simulink model "dynamicsSimulation"  (R2023a)
settings: Solver=VariableStepAuto  StartTime=0.0  StopTime=35  RelTol=1e-3
(part 2 of 2)

== matlab function dynamicsSimulation/MATLAB Function ==
  data: q input; qpp output; qp input; T input
function qpp = qpp_rrr(q,qp,T)
q2 = q(2);
q3 = q(3);
qp1 = qp(1);
qp2 = qp(2);
qp3 = qp(3);
t1 = T(1);
t2 = T(2);
t3 = T(3);
Ixx1 = 0.1;
Ixx2 = 0.1;
Ixx3 = 0.1;
Iyy2 = 0.1;
Iyy3 = 0.1;
Izz2 = 0.1;
Izz3 = 0.1;
g = 9.81;
l2 = 0.15;
lcm2 = 0.075;
lcm3 = 0.1;
m2 = 0.5;
m3 = 0.4;
%    This function was generated by the Symbolic Math Toolbox version 9.3.
%    05-Oct-2023 00:48:23

t5 = cos(q2);
t6 = cos(q3);
t7 = sin(q2);
t8 = sin(q3);
t9 = Ixx2.^2;
t10 = Ixx3.^2;
t11 = Iyy3.^2;
t12 = Izz2.^2;
t13 = Izz3.^2;
t14 = l2.^2;
t15 = l2.^3;
t17 = l2.^5;
t18 = lcm2.^2;
t19 = lcm2.^3;
t20 = lcm3.^2;
t22 = lcm3.^3;
t24 = lcm3.^5;
t25 = m2.^2;
t26 = m3.^2;
t27 = m3.^3;
t28 = q2.*2.0;
t29 = q3.*2.0;
t30 = qp1.^2;
t31 = qp2.^2;
t32 = qp3.^2;
t40 = Ixx1.*Iyy2.*Iyy3;
t41 = Ixx1.*Iyy3.*Izz3;
t42 = Iyy2.*Iyy3.*Izz2;
t43 = Iyy3.*Izz2.*Izz3;
t16 = t14.^2;
t21 = t18.^2;
t23 = t20.^2;
t33 = t5.^2;
t34 = t5.^3;
t35 = t6.^2;
t37 = t6.^3;
t39 = t6.^5;
t44 = sin(t28);
t45 = sin(t29);
t46 = t7.^2;
t47 = t7.^3;
t48 = t8.^2;
t49 = t8.^3;
t50 = Ixx1.*Iyy3.*m3.*t14;
t51 = Iyy2.*Iyy3.*m3.*t14;
t52 = Iyy3.*Izz2.*m3.*t14;
t53 = Iyy3.*Izz3.*m3.*t14;
t54 = Ixx1.*Iyy3.*m2.*t18;
t55 = Ixx1.*Iyy2.*m3.*t20;
t56 = Iyy2.*Iyy3.*m2.*t18;
t57 = Ixx1.*Izz3.*m3.*t20;
t58 = Iyy3.*Izz2.*m2.*t18;
t59 = Iyy2.*Izz2.*m3.*t20;
t60 = Iyy3.*Izz3.*m2.*t18;
t61 = Izz2.*Izz3.*m3.*t20;
t78 = Ixx1.*Iyy3.*l2.*lcm3.*m3.*t6.*2.0;
t79 = Iyy3.*Izz2.*l2.*lcm3.*m3.*t6.*2.0;
t80 = Ixx1.*m2.*m3.*t18.*t20;
t81 = Iyy2.*m2.*m3.*t18.*t20;
t82 = Izz2.*m2.*m3.*t18.*t20;
t83 = Izz3.*m2.*m3.*t18.*t20;
t91 = Ixx1.*t14.*t20.*t26;
t92 = Iyy2.*t14.*t20.*t26;
t93 = Izz2.*t14.*t20.*t26;
t94 = Izz3.*t14.*t20.*t26;
t95 = Iyy3.*m2.*m3.*t14.*t18.*2.0;
t131 = Ixx1.*l2.*t6.*t22.*t26.*2.0;
t132 = Iyy3.*lcm3.*t6.*t15.*t26.*2.0;
t133 = Izz2.*l2.*t6.*t22.*t26.*2.0;
t140 = Iyy3.*l2.*lcm3.*m2.*m3.*t6.*t18.*2.0;
t156 = t6.*t15.*t22.*t27.*2.0;
t190 = l2.*m2.*t6.*t18.*t22.*t26.*2.0;
t201 = m2.*t14.*t18.*t20.*t26.*2.0;
t36 = t33.^2;
t38 = t35.^2;
t62 = -t47;
t63 = -t49;
t64 = t46-1.0;
t65 = t48-1.0;
t66 = Iyy3.*t16.*t26;
t67 = Iyy3.*t21.*t25;
t68 = Ixx1.*Ixx3.*Iyy3.*t35;
t69 = Ixx2.*Iyy2.*Iyy3.*t33;
t70 = Ixx3.*Iyy2.*Iyy3.*t33;
t71 = t35.*t41;
t72 = Ixx2.*Iyy3.*Izz3.*t33;
t73 = Ixx3.*Iyy3.*Izz2.*t35;
t74 = Ixx3.*Iyy3.*Izz3.*t33;
t75 = t33.*t42;
t76 = t33.*t43;
t77 = t35.*t43;
t88 = t16.*t20.*t27;
t96 = m3.*t20.*t21.*t25;
t97 = Ixx2.*Iyy3.*m3.*t14.*t33;
t98 = Ixx3.*Iyy3.*m3.*t14.*t33;
t99 = Ixx3.*Iyy3.*m3.*t14.*t35;
t100 = t33.*t51;
t101 = t33.*t52;
t102 = t33.*t53;
t103 = t35.*t53;
t104 = Ixx1.*Ixx3.*m3.*t20.*t35;
t105 = Ixx2.*Iyy3.*m2.*t18.*t33;
t106 = Ixx2.*Iyy2.*m3.*t20.*t33;
t107 = Ixx3.*Iyy3.*m2.*t18.*t33;
t108 = Ixx1.*Iyy3.*m3.*t20.*t35;
t109 = Ixx3.*Iyy2.*m3.*t20.*t33;
t110 = Ixx3.*Iyy3.*m2.*t18.*t35;
t111 = t33.*t56;
t112 = t35.*t57;
t113 = Ixx2.*Izz3.*m3.*t20.*t33;
t114 = Iyy2.*Iyy3.*m3.*t20.*t33;
t115 = Ixx3.*Izz2.*m3.*t20.*t35;
t116 = Ixx3.*Izz3.*m3.*t20.*t33;
t117 = t33.*t58;
t118 = t33.*t59;
t119 = t33.*t60;
t120 = t35.*t60;
t121 = Iyy3.*Izz2.*m3.*t20.*t35;
t122 = Iyy3.*Izz3.*m3.*t20.*t33;
t123 = t33.*t61;
t124 = t35.*t61;
t126 = Ixx1.*t23.*t26.*t35;
t128 = Iyy2.*t23.*t26.*t33;
t129 = Izz2.*t23.*t26.*t35;
t130 = Izz3.*t23.*t26.*t33;
t134 = Ixx2.*Ixx3.*Iyy3.*t33.*t35;
t138 = Iyy2.*Iyy3.*Izz3.*t33.*t35;
t141 = Ixx2.*Iyy3.*l2.*lcm3.*m3.*t6.*t33.*2.0;
t143 = Iyy3.*Izz3.*l2.*lcm3.*m3.*t6.*t33.*2.0;
t157 = Iyy3.*Izz2.*l2.*lcm3.*m3.*t6.*t33.*-2.0;
t158 = Ixx2.*m2.*m3.*t18.*t20.*t33;
t159 = Ixx3.*m2.*m3.*t18.*t20.*t33;
t160 = Ixx3.*m2.*m3.*t18.*t20.*t35;
t161 = t33.*t81;
t162 = Iyy3.*m2.*m3.*t18.*t20.*t33;
t163 = Iyy3.*m2.*m3.*t18.*t20.*t35;
t164 = t33.*t82;
t165 = t33.*t83;
t166 = t35.*t83;
t173 = t14.*t23.*t27.*t35;
t176 = Ixx2.*t14.*t20.*t26.*t33;
t177 = Ixx3.*t14.*t20.*t26.*t33;
t178 = Ixx3.*t14.*t20.*t26.*t35;
t180 = t33.*t92;
t181 = t35.*t92;
t182 = Iyy3.*t14.*t20.*t26.*t35;
t183 = t33.*t93;
t184 = t33.*t94;
t187 = m2.*t18.*t23.*t26.*t33;
t189 = m2.*t18.*t23.*t26.*t35;
t191 = Ixx2.*Ixx3.*m3.*t20.*t33.*t35;
t192 = Ixx2.*Iyy3.*m3.*t20.*t33.*t35;
t197 = Iyy2.*Izz3.*m3.*t20.*t33.*t35;
t200 = t15.*t22.*t27.*t37.*2.0;
t203 = t35.*t94.*2.0;
t204 = Iyy3.*m2.*m3.*t14.*t18.*t33.*-2.0;
t213 = Ixx2.*t23.*t26.*t33.*t35;
t216 = Ixx2.*l2.*t6.*t22.*t26.*t33.*2.0;
t219 = Izz3.*l2.*t6.*t22.*t26.*t33.*2.0;
t224 = Iyy3.*l2.*lcm3.*m2.*m3.*t6.*t18.*t33.*-2.0;
t239 = Iyy3.*lcm3.*t6.*t15.*t26.*t33.*-2.0;
t240 = Izz2.*l2.*t6.*t22.*t26.*t33.*-2.0;
t245 = m2.*t14.*t18.*t20.*t26.*t35;
t248 = t6.*t15.*t22.*t27.*t33.*-2.0;
t250 = t33.*t201;
t260 = m2.*t14.*t18.*t20.*t26.*t33.*-2.0;
t267 = l2.*m2.*t6.*t18.*t22.*t26.*t33.*-2.0;
t84 = -t71;
t85 = -t75;
t86 = -t76;
t87 = -t77;
t89 = t7+t62;
t90 = t8+t63;
t125 = t33.*t66;
t127 = t33.*t67;
t135 = t35.*t70;
t136 = t35.*t72;
t137 = t33.*t73;
t139 = t35.*t76;
t144 = -t100;
t145 = -t101;
t146 = -t102;
t147 = -t103;
t148 = -t111;
t149 = -t112;
t150 = -t117;
t151 = -t118;
t152 = -t119;
t153 = -t120;
t154 = -t123;
t155 = -t124;
t172 = t33.*t88;
t174 = t35.*t88;
t175 = t14.*t23.*t27.*t38;
t179 = Ixx3.*t14.*t20.*t26.*t38;
t185 = t38.*t94;
t188 = t33.*t96;
t193 = t35.*t109;
t194 = t35.*t113;
t195 = t33.*t115;
t196 = t35.*t114;
t198 = t33.*t121;
t199 = t35.*t123;
t205 = -t161;
t206 = -t164;
t207 = -t165;
t208 = -t166;
t209 = t35.*t98.*2.0;
t210 = t35.*t102.*2.0;
t211 = t35.*t107.*2.0;
t212 = t35.*t119.*2.0;
t214 = t35.*t128;
t215 = t33.*t129;
t223 = -t200;
t226 = -t180;
t227 = -t181;
t228 = -t183;
t229 = -t184;
t230 = -t203;
t242 = t33.*t173;
t249 = t33.*t200;
t251 = t38.*t177;
t252 = t35.*t180;
t253 = t33.*t182;
t255 = t35.*t159.*2.0;
t256 = t35.*t162.*2.0;
t257 = t35.*t165.*2.0;
t261 = -t245;
t262 = t35.*t177.*2.0;
t263 = t35.*t184.*3.0;
t266 = t35.*t187.*2.0;
t272 = t33.*t245;
t167 = -t125;
t168 = -t127;
t169 = -t135;
t170 = -t136;
t171 = -t137;
t220 = -t172;
t221 = -t174;
t222 = -t175;
t225 = -t179;
t231 = -t188;
t232 = -t209;
t233 = -t193;
t234 = -t211;
t235 = -t194;
t236 = -t195;
t237 = -t196;
t238 = -t198;
t243 = t35.*t172;
t244 = t33.*t175;
t246 = -t214;
t247 = -t215;
t259 = -t242;
t264 = -t255;
t265 = -t256;
t268 = -t262;
t269 = -t253;
t270 = t38.*t229;
t271 = -t266;
t273 = t40+t41+t42+t43+t50+t51+t52+t53+t54+t55+t56+t57+t58+t59+t60+t61+t66+t67+t68+t69+t70+t72+t73+t74+t78+t79+t80+t81+t82+t83+t84+t85+t86+t87+t88+t91+t92+t93+t94+t95+t96+t97+t98+t99+t104+t105+t106+t107+t108+t109+t110+t113+t114+t115+t116+t121+t122+t126+t128+t129+t130+t131+t132+t133+t134+t138+t139+t140+t141+t143+t144+t145+t146+t147+t148+t149+t150+t151+t152+t153+t154+t155+t156+t157+t158+t159+t160+t162+t163+t167+t168+t169+t170+t171+t173+t176+t177+t178+t182+t185+t187+t189+t190+t191+t192+t197+t199+t201+t204+t205+t206+t207+t208+t210+t212+t213+t216+t219+t220+t221+t222+t223+t224+t225+t226+t227+t228+t229+t230+t231+t232+t233+t234+t235+t236+t237+t238+t239+t240+t243+t244+t246+t247+t248+t249+t251+t252+t257+t259+t260+t261+t263+t264+t265+t267+t268+t269+t270+t271+t272;
t274 = 1.0./t273;
et1 = Iyy2.*Iyy3.*t1+Iyy3.*Izz3.*t1-qp2.*qp3.*t5.*t53-qp2.*qp3.*t5.*t60-qp1.*qp2.*t42.*t44-qp1.*qp2.*t43.*t44-qp2.*qp3.*t5.*t83-qp1.*qp2.*t44.*t51-qp1.*qp2.*t44.*t52-(qp1.*qp2.*t44.*t53)./2.0-qp1.*qp2.*t44.*t56-qp2.*qp3.*t5.*t94-qp1.*qp2.*t44.*t58-qp1.*qp2.*t44.*t59-(qp1.*qp2.*t44.*t60)./2.0-qp1.*qp2.*t44.*t61-qp2.*qp3.*t5.*t99.*2.0-qp1.*qp2.*t44.*t66+qp2.*qp3.*t5.*t103.*2.0-qp1.*qp2.*t44.*t67-qp2.*qp3.*t5.*t110.*2.0-qp1.*qp2.*t44.*t81-qp1.*qp2.*t44.*t82-(qp1.*qp2.*t44.*t83)./2.0+qp2.*qp3.*t5.*t120.*2.0-qp1.*qp2.*t44.*t88-qp1.*qp2.*t44.*t92-qp1.*qp2.*t44.*t93;
et2 = qp1.*qp2.*t44.*t94.*(-1.0./2.0)-qp1.*qp2.*t44.*t96-qp2.*qp3.*t5.*t160.*2.0-qp2.*qp3.*t5.*t163.*2.0+qp2.*qp3.*t5.*t166.*2.0-qp2.*qp3.*t5.*t178.*2.0-qp2.*qp3.*t5.*t189.*2.0+qp2.*qp3.*t5.*t203+t1.*t14.*t20.*t26+t1.*t23.*t26.*t35+Ixx3.*Iyy3.*t1.*t35+Iyy2.*Iyy3.*t3.*t7+Iyy3.*Izz3.*t3.*t7-Iyy3.*Izz3.*t1.*t35+Iyy3.*m3.*t1.*t14+Iyy3.*m2.*t1.*t18+Iyy2.*m3.*t1.*t20+Izz3.*m3.*t1.*t20+Ixx3.*Iyy3.*t3.*t7.*t35-Iyy3.*Izz3.*t3.*t7.*t35+Ixx3.*m3.*t1.*t20.*t35+Iyy3.*m3.*t3.*t7.*t14+Iyy3.*m2.*t3.*t7.*t18+Iyy2.*m3.*t3.*t7.*t20+Iyy3.*m3.*t1.*t20.*t35+Izz3.*m3.*t3.*t7.*t20-Izz3.*m3.*t1.*t20.*t35+Iyy2.*qp2.*qp3.*t5.*t11-Iyy3.*qp2.*qp3.*t5.*t13-(Iyy2.*qp1.*qp2.*t11.*t44)./2.0+(Iyy3.*qp1.*qp2.*t13.*t44)./2.0;
et3 = Izz3.*qp2.*qp3.*t5.*t11-(Izz3.*qp1.*qp2.*t11.*t44)./2.0+m2.*m3.*t1.*t18.*t20+l2.*t1.*t6.*t22.*t26.*2.0-qp1.*qp2.*t5.*t7.*t73.*2.0-qp1.*qp3.*t6.*t8.*t70.*2.0+qp1.*qp2.*t5.*t7.*t77.*2.0-qp1.*qp2.*t5.*t7.*t99.*2.0-qp1.*qp3.*t6.*t8.*t98.*2.0+qp1.*qp2.*t5.*t7.*t103.*2.0+qp1.*qp3.*t6.*t8.*t102.*2.0-qp1.*qp2.*t5.*t7.*t110.*2.0-qp1.*qp3.*t6.*t8.*t107.*2.0-qp1.*qp3.*t6.*t8.*t109.*2.0-qp1.*qp2.*t5.*t7.*t115.*2.0-qp1.*qp3.*t6.*t8.*t114.*2.0+qp1.*qp2.*t5.*t7.*t120.*2.0-qp1.*qp2.*t5.*t7.*t121.*2.0+qp1.*qp3.*t6.*t8.*t119.*2.0+qp1.*qp2.*t5.*t7.*t124.*2.0-qp1.*qp3.*t6.*t8.*t122.*2.0-qp1.*qp2.*t5.*t7.*t129.*2.0-qp1.*qp3.*t6.*t8.*t128.*2.0-qp1.*qp3.*t6.*t8.*t130-qp1.*qp2.*t5.*t7.*t160.*2.0-qp1.*qp3.*t6.*t8.*t159.*2.0;
et4 = qp1.*qp2.*t5.*t7.*t163.*-2.0-qp1.*qp3.*t6.*t8.*t162.*2.0+qp1.*qp2.*t5.*t7.*t166.*2.0+qp1.*qp3.*t6.*t8.*t165.*2.0-qp1.*qp2.*t5.*t7.*t173.*6.0+qp1.*qp2.*t5.*t7.*t174.*2.0+qp1.*qp2.*t5.*t7.*t175.*6.0-qp1.*qp2.*t5.*t7.*t178.*4.0+qp1.*qp2.*t5.*t7.*t179.*6.0-qp1.*qp3.*t6.*t8.*t177.*2.0+qp1.*qp2.*t5.*t7.*t181.*2.0-qp1.*qp2.*t5.*t7.*t182.*4.0-qp1.*qp2.*t5.*t7.*t185.*6.0+qp1.*qp3.*t6.*t8.*t184.*2.0-qp1.*qp2.*t5.*t7.*t189.*2.0-qp1.*qp3.*t6.*t8.*t187.*2.0+t3.*t7.*t14.*t20.*t26+t3.*t7.*t23.*t26.*t35+t6.*t7.*t8.*t30.*t70-t6.*t7.*t8.*t30.*t72+t6.*t7.*t8.*t30.*t76-t6.*t7.*t8.*t30.*t88-t6.*t7.*t8.*t31.*t88-t6.*t7.*t8.*t30.*t92-t6.*t7.*t8.*t31.*t92-t6.*t7.*t8.*t30.*t94;
et5 = -t6.*t7.*t8.*t31.*t94+t6.*t7.*t8.*t30.*t109-t6.*t7.*t8.*t30.*t113+t6.*t7.*t8.*t30.*t114+t6.*t7.*t8.*t30.*t122.*2.0+t6.*t7.*t8.*t30.*t123+t7.*t8.*t30.*t37.*t94+t7.*t8.*t31.*t37.*t94.*3.0+t6.*t7.*t8.*t30.*t128+t6.*t7.*t8.*t30.*t130+t6.*t7.*t8.*t30.*t172+t6.*t7.*t8.*t30.*t180+t6.*t7.*t8.*t30.*t184+t7.*t8.*t30.*t37.*t177.*3.0-t7.*t8.*t30.*t37.*t184.*3.0+m2.*m3.*t3.*t7.*t18.*t20+l2.*qp1.*qp3.*t24.*t27.*t90.*2.0+m3.*qp2.*qp3.*t5.*t11.*t14+m2.*qp2.*qp3.*t5.*t11.*t18-m3.*qp2.*qp3.*t5.*t13.*t20-(m3.*qp1.*qp2.*t11.*t14.*t44)./2.0-(m2.*qp1.*qp2.*t11.*t18.*t44)./2.0+(m3.*qp1.*qp2.*t13.*t20.*t44)./2.0-l2.*t2.*t5.*t8.*t22.*t26+l2.*t3.*t6.*t7.*t22.*t26.*2.0+l2.*t3.*t7.*t22.*t26.*t37+lcm3.*t3.*t6.*t7.*t15.*t26;
et6 = qp1.*qp3.*t8.*t15.*t22.*t27.*2.0+qp1.*qp3.*t14.*t23.*t27.*t45.*2.0+qp1.*qp2.*t5.*t7.*t35.*t94.*6.0+qp1.*qp2.*t5.*t7.*t35.*t201-t2.*t5.*t6.*t8.*t23.*t26+t3.*t7.*t14.*t20.*t26.*t35.*2.0-t7.*t8.*t15.*t22.*t27.*t30-t7.*t8.*t15.*t22.*t27.*t32+Ixx3.*Iyy2.*Iyy3.*qp2.*qp3.*t5+Ixx2.*Iyy2.*Iyy3.*qp1.*qp2.*t44+(Ixx3.*Iyy2.*Iyy3.*qp1.*qp2.*t44)./2.0+Ixx3.*Iyy3.*Izz3.*qp2.*qp3.*t5+Ixx2.*Iyy3.*Izz3.*qp1.*qp2.*t44+(Ixx3.*Iyy3.*Izz3.*qp1.*qp2.*t44)./2.0-Iyy2.*Iyy3.*Izz3.*qp2.*qp3.*t5+(Iyy2.*Iyy3.*Izz3.*qp1.*qp2.*t44)./2.0-Ixx3.*Iyy3.*t2.*t5.*t6.*t8+Iyy3.*Izz3.*t2.*t5.*t6.*t8+Iyy3.*l2.*lcm3.*m3.*t1.*t6.*2.0+Ixx3.*m3.*t3.*t7.*t20.*t35+Iyy3.*m3.*t3.*t7.*t20.*t35-Izz3.*m3.*t3.*t7.*t20.*t35+Ixx3.*qp2.*qp3.*t5.*t11.*t35-Iyy3.*qp2.*qp3.*t5.*t10.*t35;
et7 = Iyy2.*qp2.*qp3.*t5.*t23.*t26.*2.0+Iyy3.*qp2.*qp3.*t5.*t13.*t35-Izz3.*qp2.*qp3.*t5.*t11.*t35+Izz3.*qp2.*qp3.*t5.*t23.*t26.*2.0-Ixx3.*Iyy2.*Iyy3.*qp2.*qp3.*t5.*t35.*2.0+Iyy2.*Iyy3.*Izz3.*qp2.*qp3.*t5.*t35.*2.0+Ixx3.*Iyy3.*m3.*qp2.*qp3.*t5.*t14+Ixx3.*Iyy3.*m2.*qp2.*qp3.*t5.*t18+Ixx3.*Iyy2.*m3.*qp2.*qp3.*t5.*t20+Ixx2.*Iyy3.*m3.*qp1.*qp2.*t14.*t44+(Ixx3.*Iyy3.*m3.*qp1.*qp2.*t14.*t44)./2.0+Ixx2.*Iyy3.*m2.*qp1.*qp2.*t18.*t44+(Ixx3.*Iyy3.*m2.*qp1.*qp2.*t18.*t44)./2.0+Ixx2.*Iyy2.*m3.*qp1.*qp2.*t20.*t44+(Ixx3.*Iyy2.*m3.*qp1.*qp2.*t20.*t44)./2.0+Iyy2.*Iyy3.*m3.*qp2.*qp3.*t5.*t20.*3.0+Ixx3.*Izz3.*m3.*qp2.*qp3.*t5.*t20+Ixx2.*Izz3.*m3.*qp1.*qp2.*t20.*t44-(Iyy2.*Iyy3.*m3.*qp1.*qp2.*t20.*t44)./2.0+(Ixx3.*Izz3.*m3.*qp1.*qp2.*t20.*t44)./2.0-Iyy2.*Izz3.*m3.*qp2.*qp3.*t5.*t20+Iyy3.*Izz3.*m3.*qp2.*qp3.*t5.*t20.*3.0;
et8 = (Iyy2.*Izz3.*m3.*qp1.*qp2.*t20.*t44)./2.0-(Iyy3.*Izz3.*m3.*qp1.*qp2.*t20.*t44)./2.0+Ixx3.*l2.*lcm3.*m3.*t3.*t7.*t37+Iyy2.*l2.*lcm3.*m3.*t3.*t6.*t7-Iyy3.*l2.*lcm3.*m3.*t2.*t5.*t8+Iyy3.*l2.*lcm3.*m3.*t3.*t6.*t7.*2.0+Izz3.*l2.*lcm3.*m3.*t3.*t6.*t7-Izz3.*l2.*lcm3.*m3.*t3.*t7.*t37+Ixx3.*l2.*qp1.*qp3.*t22.*t26.*t90.*2.0+Iyy2.*l2.*qp1.*qp3.*t8.*t22.*t26.*2.0+Iyy3.*l2.*qp1.*qp3.*t22.*t26.*t90.*2.0+Izz3.*l2.*qp1.*qp3.*t8.*t22.*t26.*2.0-Izz3.*l2.*qp1.*qp3.*t22.*t26.*t90.*2.0+Iyy2.*g.*t5.*t7.*t8.*t22.*t26+Izz3.*g.*t5.*t7.*t8.*t22.*t26+Iyy3.*lcm3.*qp1.*qp3.*t8.*t15.*t26.*2.0-Iyy2.*l2.*t7.*t8.*t22.*t26.*t30-Iyy2.*l2.*t7.*t8.*t22.*t26.*t32-Izz3.*l2.*t7.*t8.*t22.*t26.*t30-Izz3.*l2.*t7.*t8.*t22.*t26.*t32-Iyy3.*lcm3.*t7.*t8.*t15.*t26.*t30;
et9 = -Iyy3.*lcm3.*t7.*t8.*t15.*t26.*t32-Ixx3.*m3.*t2.*t5.*t6.*t8.*t20-Iyy3.*m3.*t2.*t5.*t6.*t8.*t20+Izz3.*m3.*t2.*t5.*t6.*t8.*t20-Ixx3.*qp1.*qp2.*t5.*t7.*t11.*t35+Ixx3.*qp1.*qp3.*t6.*t8.*t11.*t33+Ixx3.*qp2.*qp3.*t5.*t14.*t20.*t26-Ixx3.*qp2.*qp3.*t5.*t23.*t26.*t35+Ixx2.*qp1.*qp2.*t14.*t20.*t26.*t44+(Ixx3.*qp1.*qp2.*t14.*t20.*t26.*t44)./2.0+Iyy3.*qp1.*qp2.*t5.*t7.*t10.*t35-Iyy3.*qp1.*qp3.*t6.*t8.*t10.*t33-Iyy3.*qp1.*qp2.*t5.*t7.*t13.*t35+Iyy3.*qp1.*qp3.*t6.*t8.*t13.*t33+Iyy3.*qp2.*qp3.*t5.*t14.*t20.*t26-Iyy2.*qp2.*qp3.*t5.*t23.*t26.*t35.*2.0+Iyy3.*qp2.*qp3.*t5.*t23.*t26.*t35-(Iyy3.*qp1.*qp2.*t14.*t20.*t26.*t44)./2.0+Iyy3.*qp1.*qp3.*t14.*t20.*t26.*t45.*2.0+Izz3.*qp1.*qp2.*t5.*t7.*t11.*t35-Izz3.*qp1.*qp3.*t6.*t8.*t11.*t33;
et10 = -Izz3.*qp2.*qp3.*t5.*t23.*t26.*t35-Ixx3.*t6.*t7.*t8.*t11.*t30.*t33+Iyy3.*t6.*t7.*t8.*t10.*t30.*t33-Iyy3.*t6.*t7.*t8.*t13.*t30.*t33+Izz3.*t6.*t7.*t8.*t11.*t30.*t33-m3.*qp2.*qp3.*t5.*t10.*t20.*t35+m2.*qp2.*qp3.*t5.*t18.*t23.*t26.*2.0+m3.*qp2.*qp3.*t5.*t11.*t20.*t35+m3.*qp2.*qp3.*t5.*t13.*t20.*t35-l2.*t7.*t8.*t24.*t27.*t31.*t38+l2.*t7.*t8.*t24.*t27.*t30.*t65+l2.*t7.*t8.*t24.*t27.*t32.*t65-qp1.*qp3.*t8.*t15.*t22.*t27.*t33.*2.0-t6.*t7.*t8.*t14.*t23.*t27.*t30.*2.0-t6.*t7.*t8.*t14.*t23.*t27.*t32.*2.0-t7.*t8.*t14.*t23.*t27.*t30.*t37-t7.*t8.*t14.*t23.*t27.*t31.*t37.*3.0+t7.*t8.*t15.*t22.*t27.*t30.*t65.*2.0+t7.*t8.*t15.*t22.*t27.*t31.*t65.*3.0+Ixx2.*Ixx3.*Iyy3.*qp1.*qp2.*t5.*t7.*t35.*2.0-Ixx2.*Iyy3.*Izz3.*qp1.*qp2.*t5.*t7.*t35.*2.0;
et11 = Iyy2.*Iyy3.*Izz3.*qp1.*qp3.*t6.*t8.*t33.*2.0+Ixx2.*Ixx3.*Iyy3.*t6.*t7.*t8.*t30.*t33-Ixx3.*Iyy3.*Izz2.*t6.*t7.*t8.*t30.*t33-Iyy2.*Iyy3.*Izz3.*t6.*t7.*t8.*t30.*t33+Ixx3.*Iyy3.*l2.*lcm3.*m3.*qp1.*qp3.*t90.*2.0+Iyy2.*Iyy3.*l2.*lcm3.*m3.*qp1.*qp3.*t8.*2.0+Iyy3.*Izz3.*l2.*lcm3.*m3.*qp1.*qp3.*t8.*2.0-Iyy3.*Izz3.*l2.*lcm3.*m3.*qp1.*qp3.*t90.*2.0+Iyy2.*Iyy3.*g.*lcm3.*m3.*t5.*t7.*t8+Iyy3.*Izz3.*g.*lcm3.*m3.*t5.*t7.*t8-Iyy2.*Iyy3.*l2.*lcm3.*m3.*t7.*t8.*t30-Iyy2.*Iyy3.*l2.*lcm3.*m3.*t7.*t8.*t32-Iyy3.*Izz3.*l2.*lcm3.*m3.*t7.*t8.*t30-Iyy3.*Izz3.*l2.*lcm3.*m3.*t7.*t8.*t32-Ixx3.*Iyy2.*m3.*qp2.*qp3.*t5.*t20.*t35.*2.0-Iyy2.*Iyy3.*m3.*qp2.*qp3.*t5.*t20.*t35.*2.0+Iyy2.*Izz3.*m3.*qp2.*qp3.*t5.*t20.*t35.*2.0-Iyy3.*Izz3.*m3.*qp2.*qp3.*t5.*t20.*t35.*2.0+Ixx3.*m2.*m3.*qp2.*qp3.*t5.*t18.*t20;
et12 = Ixx2.*m2.*m3.*qp1.*qp2.*t18.*t20.*t44+(Ixx3.*m2.*m3.*qp1.*qp2.*t18.*t20.*t44)./2.0+Iyy3.*m2.*m3.*qp2.*qp3.*t5.*t18.*t20.*3.0-Iyy3.*m2.*m3.*qp1.*qp2.*t14.*t18.*t44.*2.0-(Iyy3.*m2.*m3.*qp1.*qp2.*t18.*t20.*t44)./2.0-Ixx3.*l2.*qp2.*qp3.*t5.*t6.*t22.*t26.*2.0-Ixx3.*l2.*qp1.*qp3.*t8.*t22.*t26.*t33+Iyy3.*l2.*qp2.*qp3.*t5.*t6.*t22.*t26.*2.0-Iyy2.*l2.*qp1.*qp3.*t8.*t22.*t26.*t33.*2.0+Iyy3.*l2.*qp1.*qp3.*t8.*t22.*t26.*t33+Izz3.*l2.*qp2.*qp3.*t5.*t6.*t22.*t26.*2.0-Izz3.*l2.*qp1.*qp3.*t8.*t22.*t26.*t33-Iyy3.*lcm3.*qp1.*qp3.*t8.*t15.*t26.*t33.*2.0-Ixx3.*l2.*t7.*t8.*t22.*t26.*t31.*t38.*2.0-Ixx2.*l2.*t7.*t8.*t22.*t26.*t30.*t64-Ixx3.*l2.*t7.*t8.*t22.*t26.*t30.*t64+Ixx3.*l2.*t7.*t8.*t22.*t26.*t30.*t65+Ixx3.*l2.*t7.*t8.*t22.*t26.*t32.*t65;
et13 = -Iyy2.*l2.*t7.*t8.*t22.*t26.*t30.*t64+Iyy3.*l2.*t7.*t8.*t22.*t26.*t30.*t64+Iyy2.*l2.*t7.*t8.*t22.*t26.*t31.*t65+Iyy3.*l2.*t7.*t8.*t22.*t26.*t30.*t65+Iyy3.*l2.*t7.*t8.*t22.*t26.*t32.*t65+Izz3.*l2.*t7.*t8.*t22.*t26.*t31.*t38.*2.0+Izz2.*l2.*t7.*t8.*t22.*t26.*t30.*t64-Izz3.*l2.*t7.*t8.*t22.*t26.*t30.*t64-Izz3.*l2.*t7.*t8.*t22.*t26.*t30.*t65+Izz3.*l2.*t7.*t8.*t22.*t26.*t31.*t65-Izz3.*l2.*t7.*t8.*t22.*t26.*t32.*t65+Ixx3.*lcm3.*t7.*t8.*t15.*t26.*t31.*t65-Izz3.*lcm3.*t7.*t8.*t15.*t26.*t31.*t65+Ixx2.*qp1.*qp2.*t5.*t7.*t23.*t26.*t35.*2.0+Ixx3.*qp1.*qp2.*t5.*t7.*t23.*t26.*t35-Ixx3.*qp1.*qp3.*t6.*t8.*t23.*t26.*t33-Iyy3.*qp1.*qp2.*t5.*t7.*t23.*t26.*t35+Iyy3.*qp1.*qp3.*t6.*t8.*t23.*t26.*t33+Izz3.*qp1.*qp2.*t5.*t7.*t23.*t26.*t35+Ixx2.*t6.*t7.*t8.*t23.*t26.*t30.*t33;
et14 = Ixx3.*t6.*t7.*t8.*t23.*t26.*t30.*t33-Ixx3.*t7.*t8.*t14.*t20.*t26.*t30.*t37-Ixx3.*t7.*t8.*t14.*t20.*t26.*t31.*t37.*3.0-Iyy3.*t6.*t7.*t8.*t14.*t20.*t26.*t30.*2.0-Iyy3.*t6.*t7.*t8.*t14.*t20.*t26.*t32.*2.0-Iyy3.*t6.*t7.*t8.*t23.*t26.*t30.*t33-Izz2.*t6.*t7.*t8.*t23.*t26.*t30.*t33+l2.*lcm3.*m2.*m3.*t3.*t6.*t7.*t18+l2.*lcm3.*m3.*qp2.*qp3.*t5.*t6.*t11.*2.0+l2.*lcm3.*m3.*qp1.*qp3.*t8.*t11.*t33-l2.*lcm3.*m3.*t7.*t8.*t10.*t31.*t38-l2.*lcm3.*m3.*t7.*t8.*t13.*t31.*t38+l2.*lcm3.*m3.*t7.*t8.*t11.*t30.*t64-l2.*lcm3.*m3.*t7.*t8.*t13.*t31.*t65+g.*l2.*t5.*t7.*t8.*t23.*t27.*t37+l2.*m2.*qp1.*qp3.*t8.*t18.*t22.*t26.*2.0+g.*m2.*t5.*t7.*t8.*t18.*t22.*t26-l2.*m2.*t7.*t8.*t18.*t22.*t26.*t30-l2.*m2.*t7.*t8.*t18.*t22.*t26.*t32;
et15 = l2.*qp1.*qp2.*t5.*t7.*t24.*t27.*t37.*-2.0+l2.*qp1.*qp2.*t5.*t7.*t24.*t27.*t39.*2.0-l2.*qp1.*qp3.*t8.*t24.*t27.*t33.*t35.*2.0+g.*t5.*t6.*t7.*t8.*t15.*t20.*t27+g.*t5.*t7.*t8.*t14.*t22.*t27.*t35.*2.0+m3.*qp1.*qp2.*t5.*t7.*t10.*t20.*t35-m3.*qp1.*qp2.*t5.*t7.*t11.*t20.*t35-m3.*qp1.*qp3.*t6.*t8.*t10.*t20.*t33+m3.*qp1.*qp3.*t6.*t8.*t11.*t20.*t33-m3.*qp1.*qp2.*t5.*t7.*t13.*t20.*t35+m3.*qp1.*qp3.*t6.*t8.*t13.*t20.*t33-m2.*qp1.*qp2.*t14.*t18.*t20.*t26.*t44.*2.0+l2.*t7.*t8.*t24.*t27.*t30.*t33.*t38+m3.*t6.*t7.*t8.*t10.*t20.*t30.*t33-m3.*t6.*t7.*t8.*t11.*t20.*t30.*t33-m3.*t6.*t7.*t8.*t13.*t20.*t30.*t33-qp1.*qp2.*t5.*t6.*t7.*t15.*t22.*t27.*6.0-qp1.*qp3.*t6.*t8.*t14.*t23.*t27.*t33.*4.0+qp1.*qp2.*t5.*t7.*t15.*t22.*t27.*t37.*6.0;
et16 = t7.*t8.*t15.*t22.*t27.*t30.*t33.*t35.*3.0+t7.*t8.*t14.*t23.*t27.*t30.*t33.*t37.*3.0-Ixx3.*Iyy3.*g.*l2.*m3.*t5.*t6.*t7.*t8+Iyy3.*Izz3.*g.*l2.*m3.*t5.*t6.*t7.*t8-Ixx3.*Iyy3.*l2.*lcm3.*m3.*qp2.*qp3.*t5.*t6.*2.0-Ixx3.*Iyy3.*l2.*lcm3.*m3.*qp1.*qp3.*t8.*t33-Iyy2.*Iyy3.*l2.*lcm3.*m3.*qp1.*qp3.*t8.*t33.*2.0+Iyy3.*Izz3.*l2.*lcm3.*m3.*qp2.*qp3.*t5.*t6.*2.0-Iyy3.*Izz3.*l2.*lcm3.*m3.*qp1.*qp3.*t8.*t33-Ixx3.*Iyy3.*g.*lcm2.*m2.*t5.*t6.*t7.*t8+Iyy3.*Izz3.*g.*lcm2.*m2.*t5.*t6.*t7.*t8-Ixx2.*Iyy3.*l2.*lcm3.*m3.*t7.*t8.*t30.*t64-Ixx3.*Iyy3.*l2.*lcm3.*m3.*t7.*t8.*t30.*t64+Ixx3.*Iyy2.*l2.*lcm3.*m3.*t7.*t8.*t31.*t65+Ixx3.*Iyy3.*l2.*lcm3.*m3.*t7.*t8.*t30.*t65+Ixx3.*Iyy3.*l2.*lcm3.*m3.*t7.*t8.*t32.*t65+Ixx3.*Izz3.*l2.*lcm3.*m3.*t7.*t8.*t31.*t38.*2.0-Iyy2.*Iyy3.*l2.*lcm3.*m3.*t7.*t8.*t30.*t64;
et17 = Ixx3.*Izz3.*l2.*lcm3.*m3.*t7.*t8.*t31.*t65+Iyy3.*Izz2.*l2.*lcm3.*m3.*t7.*t8.*t30.*t64-Iyy3.*Izz3.*l2.*lcm3.*m3.*t7.*t8.*t30.*t64-Iyy2.*Izz3.*l2.*lcm3.*m3.*t7.*t8.*t31.*t65-Iyy3.*Izz3.*l2.*lcm3.*m3.*t7.*t8.*t30.*t65-Iyy3.*Izz3.*l2.*lcm3.*m3.*t7.*t8.*t32.*t65+Ixx2.*Ixx3.*m3.*qp1.*qp2.*t5.*t7.*t20.*t35.*2.0+Ixx2.*Iyy3.*m3.*qp1.*qp2.*t5.*t7.*t20.*t35.*2.0-Ixx2.*Izz3.*m3.*qp1.*qp2.*t5.*t7.*t20.*t35.*2.0+Iyy2.*Izz3.*m3.*qp1.*qp3.*t6.*t8.*t20.*t33.*2.0+Iyy3.*Izz3.*m3.*qp1.*qp2.*t5.*t7.*t20.*t35.*2.0+Ixx2.*Ixx3.*m3.*t6.*t7.*t8.*t20.*t30.*t33+Ixx2.*Iyy3.*m3.*t6.*t7.*t8.*t20.*t30.*t33-Ixx3.*Izz2.*m3.*t6.*t7.*t8.*t20.*t30.*t33-Iyy2.*Izz3.*m3.*t6.*t7.*t8.*t20.*t30.*t33-Iyy3.*Izz2.*m3.*t6.*t7.*t8.*t20.*t30.*t33+Iyy3.*l2.*lcm3.*m2.*m3.*qp1.*qp3.*t8.*t18.*2.0;
et18 = Iyy3.*g.*lcm3.*m2.*m3.*t5.*t7.*t8.*t18-Iyy3.*l2.*lcm3.*m2.*m3.*t7.*t8.*t18.*t30-Iyy3.*l2.*lcm3.*m2.*m3.*t7.*t8.*t18.*t32-Ixx3.*g.*l2.*t5.*t6.*t7.*t8.*t20.*t26+Ixx3.*g.*l2.*t5.*t7.*t8.*t20.*t26.*t37+Iyy2.*g.*l2.*t5.*t6.*t7.*t8.*t20.*t26+Izz3.*g.*l2.*t5.*t6.*t7.*t8.*t20.*t26.*2.0-Izz3.*g.*l2.*t5.*t7.*t8.*t20.*t26.*t37+Ixx2.*l2.*qp1.*qp2.*t5.*t6.*t7.*t22.*t26.*4.0+Ixx3.*l2.*qp1.*qp2.*t5.*t6.*t7.*t22.*t26.*2.0-Ixx3.*l2.*qp1.*qp2.*t5.*t7.*t22.*t26.*t37.*3.0+Ixx3.*l2.*qp1.*qp2.*t5.*t7.*t22.*t26.*t39.*4.0-Ixx3.*l2.*qp1.*qp3.*t8.*t22.*t26.*t33.*t35.*2.0-Iyy2.*l2.*qp1.*qp2.*t5.*t6.*t7.*t22.*t26.*2.0-Iyy3.*l2.*qp1.*qp2.*t5.*t6.*t7.*t22.*t26.*2.0+Iyy2.*l2.*qp1.*qp2.*t5.*t7.*t22.*t26.*t37.*2.0-Iyy3.*l2.*qp1.*qp2.*t5.*t7.*t22.*t26.*t37;
et19 = Iyy3.*l2.*qp1.*qp3.*t8.*t22.*t26.*t33.*t35.*-2.0-Izz2.*l2.*qp1.*qp2.*t5.*t6.*t7.*t22.*t26.*4.0+Izz3.*l2.*qp1.*qp2.*t5.*t7.*t22.*t26.*t37.*5.0-Izz3.*l2.*qp1.*qp2.*t5.*t7.*t22.*t26.*t39.*4.0+Izz3.*l2.*qp1.*qp3.*t8.*t22.*t26.*t33.*t35.*2.0-Ixx3.*lcm3.*qp1.*qp2.*t5.*t6.*t7.*t15.*t26+Ixx3.*lcm3.*qp1.*qp2.*t5.*t7.*t15.*t26.*t37.*2.0-Iyy3.*lcm3.*qp1.*qp2.*t5.*t6.*t7.*t15.*t26.*5.0+Izz3.*lcm3.*qp1.*qp2.*t5.*t6.*t7.*t15.*t26-Izz3.*lcm3.*qp1.*qp2.*t5.*t7.*t15.*t26.*t37.*2.0+Ixx3.*l2.*t7.*t8.*t22.*t26.*t30.*t33.*t38.*2.0+Iyy2.*l2.*t7.*t8.*t22.*t26.*t30.*t33.*t35+Izz3.*l2.*t7.*t8.*t22.*t26.*t30.*t33.*t35-Izz3.*l2.*t7.*t8.*t22.*t26.*t30.*t33.*t38.*2.0+Ixx3.*lcm3.*t7.*t8.*t15.*t26.*t30.*t33.*t35-Izz3.*lcm3.*t7.*t8.*t15.*t26.*t30.*t33.*t35-Iyy3.*qp1.*qp3.*t6.*t8.*t14.*t20.*t26.*t33.*4.0;
et20 = -g.*l2.*lcm2.*m2.*t5.*t7.*t8.*t22.*t26-l2.*lcm3.*m3.*qp1.*qp2.*t5.*t6.*t7.*t11.*2.0+l2.*lcm3.*m3.*qp1.*qp2.*t5.*t6.*t7.*t13-l2.*lcm3.*m3.*qp1.*qp2.*t5.*t7.*t10.*t37+l2.*lcm3.*m3.*qp1.*qp2.*t5.*t7.*t10.*t39.*2.0-l2.*lcm3.*m3.*qp1.*qp2.*t5.*t7.*t13.*t37.*3.0+l2.*lcm3.*m3.*qp1.*qp2.*t5.*t7.*t13.*t39.*2.0-g.*lcm2.*m2.*t5.*t6.*t7.*t8.*t23.*t26+l2.*lcm3.*m3.*t7.*t8.*t10.*t30.*t33.*t38-l2.*lcm3.*m3.*t7.*t8.*t13.*t30.*t33.*t35+l2.*lcm3.*m3.*t7.*t8.*t13.*t30.*t33.*t38-l2.*m2.*qp1.*qp3.*t8.*t18.*t22.*t26.*t33.*2.0+l2.*m2.*t7.*t8.*t18.*t22.*t26.*t31.*t65-m2.*t6.*t7.*t8.*t14.*t18.*t20.*t26.*t30-m2.*t6.*t7.*t8.*t14.*t18.*t20.*t26.*t31+Ixx2.*Iyy3.*l2.*lcm3.*m3.*qp1.*qp2.*t5.*t6.*t7.*4.0-Ixx3.*Iyy2.*l2.*lcm3.*m3.*qp1.*qp2.*t5.*t6.*t7;
et21 = Ixx3.*Iyy3.*l2.*lcm3.*m3.*qp1.*qp2.*t5.*t6.*t7.*2.0+Ixx3.*Iyy2.*l2.*lcm3.*m3.*qp1.*qp2.*t5.*t7.*t37.*2.0-Ixx3.*Iyy3.*l2.*lcm3.*m3.*qp1.*qp2.*t5.*t7.*t37-Ixx3.*Iyy3.*l2.*lcm3.*m3.*qp1.*qp3.*t8.*t33.*t35.*2.0-Iyy2.*Iyy3.*l2.*lcm3.*m3.*qp1.*qp2.*t5.*t6.*t7-Ixx3.*Izz3.*l2.*lcm3.*m3.*qp1.*qp2.*t5.*t6.*t7+Ixx3.*Izz3.*l2.*lcm3.*m3.*qp1.*qp2.*t5.*t7.*t37.*4.0-Ixx3.*Izz3.*l2.*lcm3.*m3.*qp1.*qp2.*t5.*t7.*t39.*4.0+Iyy2.*Izz3.*l2.*lcm3.*m3.*qp1.*qp2.*t5.*t6.*t7-Iyy3.*Izz2.*l2.*lcm3.*m3.*qp1.*qp2.*t5.*t6.*t7.*4.0+Iyy3.*Izz3.*l2.*lcm3.*m3.*qp1.*qp2.*t5.*t6.*t7-Iyy2.*Izz3.*l2.*lcm3.*m3.*qp1.*qp2.*t5.*t7.*t37.*2.0+Iyy3.*Izz3.*l2.*lcm3.*m3.*qp1.*qp2.*t5.*t7.*t37+Iyy3.*Izz3.*l2.*lcm3.*m3.*qp1.*qp3.*t8.*t33.*t35.*2.0+Ixx3.*Iyy2.*l2.*lcm3.*m3.*t7.*t8.*t30.*t33.*t35+Ixx3.*Izz3.*l2.*lcm3.*m3.*t7.*t8.*t30.*t33.*t35;
et22 = Ixx3.*Izz3.*l2.*lcm3.*m3.*t7.*t8.*t30.*t33.*t38.*-2.0-Iyy2.*Izz3.*l2.*lcm3.*m3.*t7.*t8.*t30.*t33.*t35-Iyy3.*g.*l2.*lcm2.*lcm3.*m2.*m3.*t5.*t7.*t8-Iyy3.*l2.*lcm3.*m2.*m3.*qp1.*qp3.*t8.*t18.*t33.*2.0-Ixx3.*g.*lcm2.*m2.*m3.*t5.*t6.*t7.*t8.*t20-Iyy3.*g.*lcm2.*m2.*m3.*t5.*t6.*t7.*t8.*t20+Izz3.*g.*lcm2.*m2.*m3.*t5.*t6.*t7.*t8.*t20+Ixx3.*l2.*lcm3.*m2.*m3.*t7.*t8.*t18.*t31.*t65-Izz3.*l2.*lcm3.*m2.*m3.*t7.*t8.*t18.*t31.*t65+g.*l2.*m2.*t5.*t6.*t7.*t8.*t18.*t20.*t26-l2.*m2.*qp1.*qp2.*t5.*t6.*t7.*t18.*t22.*t26.*6.0+l2.*m2.*qp1.*qp2.*t5.*t7.*t18.*t22.*t26.*t37.*2.0+l2.*m2.*t7.*t8.*t18.*t22.*t26.*t30.*t33.*t35+m2.*t6.*t7.*t8.*t14.*t18.*t20.*t26.*t30.*t33-Ixx3.*l2.*lcm3.*m2.*m3.*qp1.*qp2.*t5.*t6.*t7.*t18+Ixx3.*l2.*lcm3.*m2.*m3.*qp1.*qp2.*t5.*t7.*t18.*t37.*2.0;
et23 = Iyy3.*l2.*lcm3.*m2.*m3.*qp1.*qp2.*t5.*t6.*t7.*t18.*-5.0+Izz3.*l2.*lcm3.*m2.*m3.*qp1.*qp2.*t5.*t6.*t7.*t18-Izz3.*l2.*lcm3.*m2.*m3.*qp1.*qp2.*t5.*t7.*t18.*t37.*2.0+Ixx3.*l2.*lcm3.*m2.*m3.*t7.*t8.*t18.*t30.*t33.*t35-Izz3.*l2.*lcm3.*m2.*m3.*t7.*t8.*t18.*t30.*t33.*t35;
et24 = Ixx1.*Iyy3.*t2.*2.0+Iyy3.*Izz2.*t2.*2.0+t30.*t44.*t50+t30.*t44.*t52.*2.0+t30.*t44.*t54+t30.*t44.*t58.*2.0+t30.*t44.*t66+t30.*t44.*t67+t30.*t44.*t80+t30.*t44.*t82.*2.0+t30.*t44.*t88+t30.*t44.*t91+t30.*t44.*t93.*2.0+t30.*t44.*t95+t30.*t44.*t96+t30.*t44.*t201+Ixx1.*t11.*t30.*t44+Iyy3.*t12.*t30.*t44+Izz2.*t11.*t30.*t44-qp1.*qp3.*t5.*t41.*2.0-qp1.*qp3.*t5.*t43.*2.0-qp1.*qp3.*t5.*t53.*2.0-qp1.*qp3.*t5.*t57.*2.0-qp1.*qp3.*t5.*t60.*2.0-qp1.*qp3.*t5.*t61.*2.0-qp1.*qp3.*t5.*t68.*4.0+qp1.*qp3.*t5.*t71.*4.0+qp1.*qp3.*t34.*t43.*2.0-qp1.*qp3.*t5.*t73.*4.0+qp1.*qp3.*t5.*t77.*4.0+qp1.*qp3.*t34.*t53.*2.0-qp2.*qp3.*t41.*t45.*2.0-qp1.*qp3.*t5.*t83.*2.0-qp2.*qp3.*t43.*t45.*2.0+qp1.*qp3.*t34.*t60.*2.0+qp1.*qp3.*t34.*t61.*2.0;
et25 = qp1.*qp3.*t5.*t94.*-2.0-qp2.*qp3.*t45.*t53.*2.0-qp2.*qp3.*t45.*t57.*2.0-qp1.*qp3.*t5.*t99.*4.0-qp2.*qp3.*t45.*t60.*2.0+qp1.*qp3.*t34.*t73.*4.0-qp2.*qp3.*t45.*t61.*2.0+qp1.*qp3.*t5.*t103.*4.0-qp1.*qp3.*t5.*t104.*4.0-qp1.*qp3.*t34.*t77.*4.0-qp1.*qp3.*t5.*t108.*4.0-qp1.*qp3.*t5.*t110.*4.0+qp1.*qp3.*t5.*t112.*4.0+qp1.*qp3.*t34.*t83.*2.0-qp1.*qp3.*t5.*t115.*4.0+qp1.*qp3.*t5.*t120.*4.0-qp1.*qp3.*t5.*t121.*4.0+qp1.*qp3.*t34.*t94.*2.0+qp1.*qp3.*t5.*t124.*4.0-qp2.*qp3.*t45.*t83.*2.0-qp1.*qp3.*t5.*t126.*4.0+qp1.*qp3.*t34.*t99.*4.0-qp1.*qp3.*t5.*t129.*4.0-qp1.*qp3.*t34.*t103.*4.0-qp2.*qp3.*t45.*t94.*2.0+qp1.*qp3.*t34.*t110.*4.0+qp1.*qp3.*t34.*t115.*4.0-qp1.*qp3.*t34.*t120.*4.0+qp1.*qp3.*t34.*t121.*4.0-qp1.*qp3.*t34.*t124.*4.0;
et26 = qp1.*qp3.*t34.*t129.*4.0-qp1.*qp3.*t5.*t160.*4.0-qp1.*qp3.*t5.*t163.*4.0+qp1.*qp3.*t5.*t166.*4.0+qp1.*qp3.*t5.*t175.*4.0-qp1.*qp3.*t5.*t178.*6.0+qp1.*qp3.*t5.*t179.*4.0+qp1.*qp3.*t5.*t182.*2.0-qp1.*qp3.*t5.*t185.*4.0-qp1.*qp3.*t5.*t189.*4.0+qp1.*qp3.*t34.*t160.*4.0+qp1.*qp3.*t34.*t163.*4.0-qp1.*qp3.*t34.*t166.*4.0-qp1.*qp3.*t34.*t175.*4.0+qp1.*qp3.*t34.*t178.*6.0-qp1.*qp3.*t34.*t179.*4.0-qp1.*qp3.*t34.*t182.*2.0+qp1.*qp3.*t34.*t185.*4.0+qp1.*qp3.*t34.*t189.*4.0+t2.*t14.*t20.*t26.*2.0+t2.*t23.*t26.*t33.*2.0+t5.*t7.*t30.*t68.*2.0-t5.*t7.*t30.*t71.*2.0+t5.*t7.*t30.*t73.*2.0-t5.*t7.*t30.*t77.*2.0-t7.*t30.*t34.*t52.*4.0-t7.*t30.*t34.*t58.*4.0-t7.*t30.*t34.*t66.*2.0-t7.*t30.*t34.*t67.*2.0+t5.*t7.*t30.*t99.*2.0;
et27 = t7.*t30.*t34.*t73.*-4.0-t5.*t7.*t30.*t103.*2.0+t5.*t7.*t30.*t104.*2.0+t7.*t30.*t34.*t77.*4.0+t5.*t7.*t30.*t108.*2.0+t5.*t7.*t30.*t110.*2.0-t7.*t30.*t34.*t82.*4.0-t5.*t7.*t30.*t112.*2.0+t5.*t7.*t30.*t115.*2.0-t7.*t30.*t34.*t88.*2.0-t5.*t7.*t30.*t120.*2.0+t5.*t7.*t30.*t121.*2.0-t7.*t30.*t34.*t93.*4.0-t5.*t7.*t30.*t124.*2.0-t7.*t30.*t34.*t96.*2.0+t5.*t7.*t30.*t126.*2.0-t7.*t30.*t34.*t99.*4.0+t5.*t7.*t30.*t129.*2.0+t7.*t30.*t34.*t103.*4.0-t7.*t30.*t34.*t110.*4.0-t7.*t30.*t34.*t115.*4.0+t7.*t30.*t34.*t120.*4.0-t7.*t30.*t34.*t121.*4.0+t7.*t30.*t34.*t124.*4.0+t5.*t7.*t31.*t156-t7.*t30.*t34.*t129.*4.0+t5.*t7.*t30.*t160.*2.0+t5.*t7.*t30.*t163.*2.0-t5.*t7.*t30.*t166.*2.0+t5.*t7.*t30.*t173.*2.0;
et28 = t5.*t7.*t30.*t174.*-2.0+t5.*t7.*t31.*t173.*4.0-t5.*t7.*t30.*t175.*4.0-t5.*t7.*t32.*t173.*2.0-t5.*t7.*t31.*t175.*4.0+t5.*t7.*t30.*t178.*6.0-t5.*t7.*t30.*t179.*4.0+t5.*t7.*t31.*t178.*4.0-t5.*t7.*t31.*t179.*4.0-t5.*t7.*t30.*t182.*2.0-t5.*t7.*t32.*t182.*2.0+t5.*t7.*t30.*t185.*4.0+t5.*t7.*t31.*t185.*4.0+t5.*t7.*t30.*t189.*2.0-t7.*t30.*t34.*t160.*4.0-t7.*t30.*t34.*t163.*4.0+t7.*t30.*t34.*t166.*4.0-t7.*t30.*t34.*t173.*6.0+t7.*t30.*t34.*t174.*2.0+t7.*t30.*t34.*t175.*6.0-t7.*t30.*t34.*t178.*1.0e+1+t7.*t30.*t34.*t179.*6.0-t7.*t30.*t34.*t185.*6.0-t7.*t30.*t34.*t189.*4.0-t5.*t7.*t30.*t245.*2.0+Ixx2.*Iyy3.*t2.*t33.*2.0+Ixx3.*Iyy3.*t2.*t33.*2.0-Iyy3.*Izz2.*t2.*t33.*2.0+Ixx1.*m3.*t2.*t20.*2.0+Iyy3.*m3.*t2.*t14.*2.0;
et29 = Iyy3.*m2.*t2.*t18.*2.0+Izz2.*m3.*t2.*t20.*2.0-Ixx1.*Ixx2.*Iyy3.*t30.*t44-Ixx1.*Ixx3.*Iyy3.*t30.*t44+Ixx1.*Iyy3.*Izz2.*t30.*t44-Ixx2.*Iyy3.*Izz2.*t30.*t44-Ixx3.*Iyy3.*Izz2.*t30.*t44-Ixx3.*Iyy3.*t2.*t33.*t35.*2.0+Iyy3.*Izz3.*t2.*t33.*t35.*2.0+Iyy3.*g.*t7.*t15.*t26.*2.0+Iyy3.*g.*t7.*t19.*t25.*2.0-Iyy3.*g.*t15.*t26.*t89.*2.0-Iyy3.*g.*t19.*t25.*t89.*2.0+Ixx2.*m3.*t2.*t20.*t33.*2.0+Ixx3.*m3.*t2.*t20.*t33.*2.0-Iyy3.*m3.*t2.*t14.*t33.*2.0-Iyy3.*m2.*t2.*t18.*t33.*2.0+Iyy3.*m3.*t2.*t20.*t33.*2.0-Izz2.*m3.*t2.*t20.*t33.*2.0-Ixx1.*qp1.*qp3.*t5.*t11.*2.0-Ixx2.*qp1.*qp3.*t11.*t34.*2.0-Ixx3.*qp1.*qp3.*t11.*t34.*2.0+Iyy3.*qp1.*qp3.*t10.*t34.*2.0-Izz2.*qp1.*qp3.*t5.*t11.*2.0+Izz2.*qp1.*qp3.*t11.*t34.*2.0+Ixx2.*t7.*t11.*t30.*t34.*2.0+Ixx3.*t7.*t11.*t30.*t34.*2.0;
et30 = Iyy3.*t7.*t9.*t30.*t34.*-2.0-Iyy3.*t7.*t10.*t30.*t34.*2.0-Iyy3.*t7.*t12.*t30.*t34.*2.0-Izz2.*t7.*t11.*t30.*t34.*2.0+m2.*m3.*t2.*t18.*t20.*2.0+g.*t7.*t15.*t20.*t27.*2.0-g.*t15.*t20.*t27.*t89.*2.0+m3.*t11.*t14.*t30.*t44+m2.*t11.*t18.*t30.*t44+m3.*t12.*t20.*t30.*t44-qp2.*qp3.*t6.*t8.*t72.*4.0+qp2.*qp3.*t6.*t8.*t76.*4.0-qp2.*qp3.*t6.*t8.*t98.*4.0+qp2.*qp3.*t6.*t8.*t102.*4.0-qp2.*qp3.*t6.*t8.*t107.*4.0-qp2.*qp3.*t6.*t8.*t113.*4.0+qp1.*qp3.*t5.*t35.*t94.*6.0+qp2.*qp3.*t6.*t8.*t119.*4.0+qp2.*qp3.*t6.*t8.*t122.*4.0+qp2.*qp3.*t6.*t8.*t123.*4.0+qp2.*qp3.*t8.*t37.*t94.*4.0+qp2.*qp3.*t6.*t8.*t130.*2.0-qp1.*qp3.*t34.*t35.*t94.*6.0-qp2.*qp3.*t6.*t8.*t159.*4.0-qp2.*qp3.*t6.*t8.*t162.*4.0+qp2.*qp3.*t6.*t8.*t165.*4.0-qp2.*qp3.*t6.*t8.*t177.*4.0;
et31 = qp2.*qp3.*t6.*t8.*t184.*4.0-qp2.*qp3.*t6.*t8.*t187.*4.0+qp2.*qp3.*t8.*t37.*t177.*4.0-qp2.*qp3.*t8.*t37.*t184.*4.0-t2.*t14.*t20.*t26.*t33.*2.0-t2.*t14.*t20.*t26.*t35.*2.0-t2.*t23.*t26.*t33.*t35.*2.0+t14.*t23.*t27.*t30.*t44+t14.*t23.*t27.*t32.*t44-t5.*t7.*t30.*t35.*t93.*2.0-t5.*t7.*t30.*t35.*t94.*4.0-t5.*t7.*t31.*t35.*t94.*4.0+t7.*t30.*t34.*t35.*t93.*2.0+t7.*t30.*t34.*t35.*t94.*8.0+t7.*t30.*t34.*t35.*t201+g.*m3.*t7.*t19.*t20.*t25.*2.0-g.*m3.*t19.*t20.*t25.*t89.*2.0-m2.*m3.*t2.*t18.*t20.*t33.*2.0+g.*t6.*t7.*t14.*t22.*t27.*2.0-g.*t7.*t15.*t20.*t27.*t35.*2.0-g.*t7.*t14.*t22.*t27.*t37.*2.0-m3.*qp1.*qp3.*t5.*t11.*t14.*2.0-m2.*qp1.*qp3.*t5.*t11.*t18.*2.0+m3.*qp1.*qp3.*t11.*t14.*t34.*2.0+m2.*qp1.*qp3.*t11.*t18.*t34.*2.0;
et32 = m3.*qp1.*qp3.*t10.*t20.*t34.*2.0-m3.*qp1.*qp3.*t11.*t20.*t34.*2.0-l2.*t1.*t5.*t8.*t22.*t26.*2.0-m3.*t7.*t11.*t14.*t30.*t34.*2.0-m2.*t7.*t11.*t18.*t30.*t34.*2.0-m3.*t7.*t9.*t20.*t30.*t34.*2.0-m3.*t7.*t10.*t20.*t30.*t34.*2.0+m3.*t7.*t11.*t20.*t30.*t34.*2.0-m3.*t7.*t12.*t20.*t30.*t34.*2.0-qp1.*qp3.*t5.*t14.*t23.*t27.*4.0+qp2.*qp3.*t8.*t15.*t22.*t27.*4.0+qp1.*qp2.*t6.*t7.*t8.*t72.*4.0-qp1.*qp2.*t6.*t7.*t8.*t76.*4.0+qp1.*qp3.*t14.*t23.*t27.*t34.*4.0+qp2.*qp3.*t14.*t23.*t27.*t45.*2.0+qp1.*qp2.*t6.*t7.*t8.*t98.*4.0-qp1.*qp2.*t6.*t7.*t8.*t102.*4.0+qp1.*qp2.*t6.*t7.*t8.*t107.*4.0+qp1.*qp2.*t6.*t7.*t8.*t113.*4.0-qp1.*qp2.*t6.*t7.*t8.*t119.*4.0-qp1.*qp2.*t6.*t7.*t8.*t122.*4.0-qp1.*qp2.*t6.*t7.*t8.*t123.*4.0-qp1.*qp2.*t6.*t7.*t8.*t130.*2.0;
et33 = qp2.*qp3.*t15.*t22.*t27.*t90.*-4.0+qp1.*qp2.*t6.*t7.*t8.*t159.*4.0+qp1.*qp2.*t6.*t7.*t8.*t162.*4.0-qp1.*qp2.*t6.*t7.*t8.*t165.*4.0+qp1.*qp2.*t6.*t7.*t8.*t177.*6.0-qp1.*qp2.*t6.*t7.*t8.*t184.*6.0+qp1.*qp2.*t6.*t7.*t8.*t187.*4.0-qp1.*qp2.*t7.*t8.*t37.*t177.*8.0+qp1.*qp2.*t7.*t8.*t37.*t184.*8.0-t1.*t5.*t6.*t8.*t23.*t26.*2.0+t2.*t14.*t20.*t26.*t33.*t35.*2.0+Ixx1.*Ixx3.*Iyy3.*qp1.*qp3.*t5.*2.0+Ixx2.*Ixx3.*Iyy3.*qp1.*qp3.*t34.*2.0+Ixx1.*Ixx3.*Iyy3.*qp2.*qp3.*t45.*2.0+Ixx3.*Iyy3.*Izz2.*qp1.*qp3.*t5.*2.0-Ixx2.*Iyy3.*Izz3.*qp1.*qp3.*t34.*2.0-Ixx3.*Iyy3.*Izz2.*qp1.*qp3.*t34.*2.0-Ixx3.*Iyy3.*Izz3.*qp1.*qp3.*t34.*2.0+Ixx3.*Iyy3.*Izz2.*qp2.*qp3.*t45.*2.0-Ixx2.*Ixx3.*Iyy3.*t7.*t30.*t34.*4.0+Ixx2.*Iyy3.*Izz2.*t7.*t30.*t34.*4.0+Ixx3.*Iyy3.*Izz2.*t7.*t30.*t34.*4.0+Ixx1.*Iyy3.*g.*l2.*m3.*t7.*2.0;
et34 = Ixx2.*Iyy3.*g.*l2.*m3.*t89.*2.0+Ixx3.*Iyy3.*g.*l2.*m3.*t89.*2.0+Iyy3.*Izz2.*g.*l2.*m3.*t7.*2.0-Iyy3.*Izz2.*g.*l2.*m3.*t89.*2.0+Ixx1.*Iyy3.*g.*lcm2.*m2.*t7.*2.0+Ixx2.*Iyy3.*g.*lcm2.*m2.*t89.*2.0+Ixx3.*Iyy3.*g.*lcm2.*m2.*t89.*2.0+Iyy3.*Izz2.*g.*lcm2.*m2.*t7.*2.0-Iyy3.*Izz2.*g.*lcm2.*m2.*t89.*2.0-Ixx1.*Ixx2.*m3.*t20.*t30.*t44-Ixx1.*Ixx3.*m3.*t20.*t30.*t44-Ixx2.*Iyy3.*m3.*t14.*t30.*t44-Ixx3.*Iyy3.*m3.*t14.*t30.*t44-Ixx2.*Iyy3.*m2.*t18.*t30.*t44-Ixx3.*Iyy3.*m2.*t18.*t30.*t44+Ixx1.*Iyy3.*m3.*t20.*t30.*t44+Ixx1.*Izz2.*m3.*t20.*t30.*t44-Ixx2.*Izz2.*m3.*t20.*t30.*t44-Ixx3.*Izz2.*m3.*t20.*t30.*t44+Iyy3.*Izz2.*m3.*t20.*t30.*t44-Ixx3.*Iyy3.*t1.*t5.*t6.*t8.*2.0+Iyy3.*Izz3.*t1.*t5.*t6.*t8.*2.0+Ixx1.*g.*l2.*t7.*t20.*t26.*2.0+Ixx2.*g.*l2.*t20.*t26.*t89.*2.0;
et35 = Ixx3.*g.*l2.*t20.*t26.*t89.*2.0+Izz2.*g.*l2.*t7.*t20.*t26.*2.0-Izz2.*g.*l2.*t20.*t26.*t89.*2.0+Ixx1.*g.*t6.*t7.*t22.*t26.*2.0+Izz2.*g.*t6.*t7.*t22.*t26.*2.0-Ixx3.*m3.*t2.*t20.*t33.*t35.*2.0-Iyy3.*m3.*t2.*t20.*t33.*t35.*2.0+Izz3.*m3.*t2.*t20.*t33.*t35.*2.0+Ixx3.*qp1.*qp3.*t11.*t34.*t35.*2.0+Ixx3.*qp1.*qp3.*t23.*t26.*t34.*2.0+Ixx1.*qp2.*qp3.*t23.*t26.*t45.*2.0-Iyy3.*qp1.*qp3.*t10.*t34.*t35.*2.0+Iyy3.*qp1.*qp3.*t13.*t34.*t35.*2.0-Iyy3.*qp1.*qp3.*t23.*t26.*t34.*2.0-Izz3.*qp1.*qp3.*t11.*t34.*t35.*2.0-Izz3.*qp1.*qp3.*t23.*t26.*t34.*2.0+Izz2.*qp2.*qp3.*t23.*t26.*t45.*2.0-Ixx3.*t7.*t11.*t30.*t34.*t35.*2.0-Ixx2.*t7.*t23.*t26.*t30.*t34.*2.0-Ixx3.*t7.*t23.*t26.*t30.*t34.*2.0-Ixx2.*t14.*t20.*t26.*t30.*t44-Ixx3.*t14.*t20.*t26.*t30.*t44+Iyy3.*t7.*t10.*t30.*t34.*t35.*2.0;
et36 = Iyy3.*t7.*t13.*t30.*t34.*t35.*-2.0+Iyy3.*t7.*t23.*t26.*t30.*t34.*2.0+Iyy3.*t14.*t20.*t26.*t30.*t44.*2.0+Iyy3.*t14.*t20.*t26.*t32.*t44+Izz3.*t7.*t11.*t30.*t34.*t35.*2.0+Izz2.*t7.*t23.*t26.*t30.*t34.*2.0+g.*lcm2.*m2.*t23.*t26.*t89.*2.0-Ixx2.*Ixx3.*Iyy3.*qp1.*qp3.*t34.*t35.*4.0+Ixx2.*Iyy3.*Izz3.*qp1.*qp3.*t34.*t35.*4.0+Ixx2.*Ixx3.*Iyy3.*t7.*t30.*t34.*t35.*4.0-Ixx2.*Iyy3.*Izz3.*t7.*t30.*t34.*t35.*4.0+Ixx1.*Iyy3.*g.*lcm3.*m3.*t6.*t7.*2.0+Iyy3.*Izz2.*g.*lcm3.*m3.*t6.*t7.*2.0+Ixx1.*Ixx3.*m3.*qp1.*qp3.*t5.*t20.*2.0+Ixx2.*Ixx3.*m3.*qp1.*qp3.*t20.*t34.*2.0+Ixx1.*Ixx3.*m3.*qp2.*qp3.*t20.*t45.*2.0+Ixx3.*Iyy3.*m3.*qp1.*qp3.*t5.*t14.*2.0+Ixx3.*Iyy3.*m2.*qp1.*qp3.*t5.*t18.*2.0-Ixx1.*Iyy3.*m3.*qp1.*qp3.*t5.*t20.*2.0-Ixx3.*Iyy3.*m3.*qp1.*qp3.*t14.*t34.*2.0-Ixx3.*Iyy3.*m2.*qp1.*qp3.*t18.*t34.*2.0-Ixx2.*Iyy3.*m3.*qp1.*qp3.*t20.*t34.*2.0;
et37 = Ixx3.*Iyy3.*m3.*qp2.*qp3.*t14.*t45.*2.0+Ixx3.*Iyy3.*m2.*qp2.*qp3.*t18.*t45.*2.0+Ixx1.*Iyy3.*m3.*qp2.*qp3.*t20.*t45.*2.0+Ixx3.*Izz2.*m3.*qp1.*qp3.*t5.*t20.*2.0-Ixx2.*Izz3.*m3.*qp1.*qp3.*t20.*t34.*2.0-Ixx3.*Izz2.*m3.*qp1.*qp3.*t20.*t34.*2.0-Ixx3.*Izz3.*m3.*qp1.*qp3.*t20.*t34.*2.0+Ixx3.*Izz2.*m3.*qp2.*qp3.*t20.*t45.*2.0-Iyy3.*Izz2.*m3.*qp1.*qp3.*t5.*t20.*2.0+Iyy3.*Izz2.*m3.*qp1.*qp3.*t20.*t34.*2.0-Iyy3.*Izz3.*m3.*qp1.*qp3.*t20.*t34.*2.0+Iyy3.*Izz2.*m3.*qp2.*qp3.*t20.*t45.*2.0-Ixx2.*Ixx3.*m3.*t7.*t20.*t30.*t34.*4.0+Ixx2.*Iyy3.*m3.*t7.*t14.*t30.*t34.*4.0+Ixx3.*Iyy3.*m3.*t7.*t14.*t30.*t34.*4.0+Ixx2.*Iyy3.*m2.*t7.*t18.*t30.*t34.*4.0+Ixx3.*Iyy3.*m2.*t7.*t18.*t30.*t34.*4.0+Ixx2.*Izz2.*m3.*t7.*t20.*t30.*t34.*4.0+Ixx3.*Izz2.*m3.*t7.*t20.*t30.*t34.*4.0-Ixx3.*Iyy3.*t3.*t5.*t6.*t7.*t8.*2.0+Iyy3.*Izz3.*t3.*t5.*t6.*t7.*t8.*2.0;
et38 = Iyy3.*g.*l2.*m2.*m3.*t7.*t18.*2.0-Iyy3.*g.*l2.*m2.*m3.*t18.*t89.*2.0+Ixx1.*g.*lcm2.*m2.*m3.*t7.*t20.*2.0+Ixx2.*g.*lcm2.*m2.*m3.*t20.*t89.*2.0+Ixx3.*g.*lcm2.*m2.*m3.*t20.*t89.*2.0+Iyy3.*g.*lcm2.*m2.*m3.*t7.*t14.*2.0-Iyy3.*g.*lcm2.*m2.*m3.*t14.*t89.*2.0+Iyy3.*g.*lcm2.*m2.*m3.*t20.*t89.*2.0+Izz2.*g.*lcm2.*m2.*m3.*t7.*t20.*2.0-Izz2.*g.*lcm2.*m2.*m3.*t20.*t89.*2.0-Iyy3.*l2.*lcm3.*m3.*t1.*t5.*t8.*2.0+Iyy3.*g.*lcm3.*t6.*t7.*t14.*t26.*2.0-Ixx2.*m2.*m3.*t18.*t20.*t30.*t44-Ixx3.*m2.*m3.*t18.*t20.*t30.*t44+Iyy3.*m2.*m3.*t18.*t20.*t30.*t44+Ixx1.*l2.*qp2.*qp3.*t8.*t22.*t26.*4.0+Izz2.*l2.*qp2.*qp3.*t8.*t22.*t26.*4.0+Ixx2.*g.*t6.*t7.*t22.*t26.*t33.*2.0-Izz2.*g.*t6.*t7.*t22.*t26.*t33.*2.0+Izz3.*g.*t6.*t7.*t22.*t26.*t33.*2.0+Iyy3.*lcm3.*qp2.*qp3.*t8.*t15.*t26.*4.0;
et39 = Ixx3.*m3.*t1.*t5.*t6.*t8.*t20.*-2.0-Iyy3.*m3.*t1.*t5.*t6.*t8.*t20.*2.0+Izz3.*m3.*t1.*t5.*t6.*t8.*t20.*2.0-Ixx3.*qp2.*qp3.*t6.*t8.*t11.*t33.*2.0+Ixx3.*qp1.*qp3.*t5.*t14.*t20.*t26.*2.0-Ixx3.*qp1.*qp3.*t14.*t20.*t26.*t34.*2.0+Ixx3.*qp2.*qp3.*t14.*t20.*t26.*t45.*2.0-Ixx2.*qp1.*qp3.*t23.*t26.*t34.*t35.*4.0-Ixx3.*qp1.*qp3.*t23.*t26.*t34.*t35.*2.0+Iyy3.*qp2.*qp3.*t6.*t8.*t10.*t33.*2.0-Iyy3.*qp2.*qp3.*t6.*t8.*t13.*t33.*2.0-Iyy3.*qp1.*qp3.*t5.*t14.*t20.*t26.*6.0+Iyy3.*qp1.*qp3.*t14.*t20.*t26.*t34.*6.0+Iyy3.*qp2.*qp3.*t14.*t20.*t26.*t45.*2.0+Iyy3.*qp1.*qp3.*t23.*t26.*t34.*t35.*2.0+Izz3.*qp2.*qp3.*t6.*t8.*t11.*t33.*2.0-Izz3.*qp1.*qp3.*t23.*t26.*t34.*t35.*2.0+Ixx2.*t7.*t14.*t20.*t26.*t30.*t34.*4.0+Ixx3.*t7.*t14.*t20.*t26.*t30.*t34.*4.0+Ixx2.*t7.*t23.*t26.*t30.*t34.*t35.*4.0+Ixx3.*t7.*t23.*t26.*t30.*t34.*t35.*2.0;
et40 = Iyy3.*t7.*t14.*t20.*t26.*t30.*t34.*-2.0-Iyy3.*t7.*t23.*t26.*t30.*t34.*t35.*2.0+Izz3.*t7.*t23.*t26.*t30.*t34.*t35.*2.0+g.*l2.*m2.*t7.*t18.*t20.*t26.*2.0-g.*l2.*m2.*t18.*t20.*t26.*t89.*2.0+g.*lcm2.*m2.*t7.*t14.*t20.*t26.*2.0-g.*lcm2.*m2.*t14.*t20.*t26.*t89.*2.0-g.*l2.*t7.*t23.*t27.*t33.*t35.*2.0+g.*l2.*t7.*t23.*t27.*t33.*t38.*2.0+g.*m2.*t6.*t7.*t18.*t22.*t26.*2.0-l2.*qp1.*qp3.*t5.*t6.*t24.*t27.*4.0+l2.*qp1.*qp3.*t6.*t24.*t27.*t34.*4.0+l2.*qp1.*qp3.*t5.*t24.*t27.*t37.*4.0-l2.*qp1.*qp3.*t24.*t27.*t34.*t37.*4.0-g.*t6.*t7.*t14.*t22.*t27.*t33.*4.0+g.*t7.*t15.*t20.*t27.*t33.*t35.*2.0+g.*t7.*t14.*t22.*t27.*t33.*t37.*4.0-m3.*qp1.*qp3.*t10.*t20.*t34.*t35.*2.0+m3.*qp1.*qp3.*t11.*t20.*t34.*t35.*2.0+m3.*qp1.*qp3.*t13.*t20.*t34.*t35.*2.0+m2.*qp2.*qp3.*t18.*t23.*t26.*t45.*2.0;
et41 = l2.*t3.*t5.*t7.*t8.*t22.*t26.*-2.0+l2.*t5.*t6.*t7.*t24.*t27.*t30.*2.0+l2.*t5.*t6.*t7.*t24.*t27.*t32.*2.0-l2.*t5.*t7.*t24.*t27.*t30.*t37.*2.0+l2.*t5.*t7.*t24.*t27.*t31.*t37.*2.0-l2.*t5.*t7.*t24.*t27.*t32.*t37.*2.0-l2.*t5.*t7.*t24.*t27.*t31.*t39.*2.0-l2.*t7.*t24.*t27.*t30.*t34.*t37.*2.0+l2.*t7.*t24.*t27.*t30.*t34.*t39.*2.0+m3.*t7.*t10.*t20.*t30.*t34.*t35.*2.0+m2.*t7.*t18.*t23.*t26.*t30.*t34.*2.0-m3.*t7.*t11.*t20.*t30.*t34.*t35.*2.0-m3.*t7.*t13.*t20.*t30.*t34.*t35.*2.0-qp1.*qp3.*t5.*t6.*t15.*t22.*t27.*4.0+qp1.*qp3.*t6.*t15.*t22.*t27.*t34.*4.0+qp1.*qp3.*t5.*t15.*t22.*t27.*t37.*4.0-qp2.*qp3.*t8.*t15.*t22.*t27.*t33.*4.0-qp2.*qp3.*t8.*t14.*t23.*t27.*t37.*4.0-qp1.*qp3.*t15.*t22.*t27.*t34.*t37.*4.0-t3.*t5.*t6.*t7.*t8.*t23.*t26.*2.0;
et42 = t5.*t6.*t7.*t15.*t22.*t27.*t30.*6.0-t6.*t7.*t15.*t22.*t27.*t30.*t34.*6.0-t5.*t7.*t15.*t22.*t27.*t30.*t37.*6.0-t5.*t7.*t15.*t22.*t27.*t31.*t37.*2.0+t7.*t15.*t22.*t27.*t30.*t34.*t37.*6.0+Ixx2.*Ixx3.*Iyy3.*qp2.*qp3.*t6.*t8.*t33.*4.0-Ixx3.*Iyy3.*Izz2.*qp2.*qp3.*t6.*t8.*t33.*4.0-Ixx3.*Iyy3.*g.*l2.*m3.*t7.*t33.*t35.*2.0+Iyy3.*Izz3.*g.*l2.*m3.*t7.*t33.*t35.*2.0+Ixx1.*Iyy3.*l2.*lcm3.*m3.*qp2.*qp3.*t8.*4.0+Iyy3.*Izz2.*l2.*lcm3.*m3.*qp2.*qp3.*t8.*4.0+Ixx2.*Iyy3.*g.*lcm3.*m3.*t6.*t7.*t33.*2.0-Ixx3.*Iyy3.*g.*lcm2.*m2.*t7.*t33.*t35.*2.0-Iyy3.*Izz2.*g.*lcm3.*m3.*t6.*t7.*t33.*2.0+Iyy3.*Izz3.*g.*lcm3.*m3.*t6.*t7.*t33.*2.0+Iyy3.*Izz3.*g.*lcm2.*m2.*t7.*t33.*t35.*2.0-Ixx2.*Ixx3.*m3.*qp1.*qp3.*t20.*t34.*t35.*4.0-Ixx2.*Iyy3.*m3.*qp1.*qp3.*t20.*t34.*t35.*4.0+Ixx2.*Izz3.*m3.*qp1.*qp3.*t20.*t34.*t35.*4.0;
et43 = Iyy3.*Izz3.*m3.*qp1.*qp3.*t20.*t34.*t35.*-4.0+Ixx2.*Ixx3.*m3.*t7.*t20.*t30.*t34.*t35.*4.0+Ixx2.*Iyy3.*m3.*t7.*t20.*t30.*t34.*t35.*4.0-Ixx2.*Izz3.*m3.*t7.*t20.*t30.*t34.*t35.*4.0+Iyy3.*Izz3.*m3.*t7.*t20.*t30.*t34.*t35.*4.0+Iyy3.*g.*lcm3.*m2.*m3.*t6.*t7.*t18.*2.0-Iyy3.*l2.*lcm3.*m3.*t3.*t5.*t7.*t8.*2.0-Ixx3.*g.*l2.*t7.*t20.*t26.*t33.*t35.*4.0+Ixx3.*g.*l2.*t7.*t20.*t26.*t33.*t38.*2.0+Izz3.*g.*l2.*t7.*t20.*t26.*t33.*t35.*4.0-Izz3.*g.*l2.*t7.*t20.*t26.*t33.*t38.*2.0-Iyy3.*g.*lcm3.*t6.*t7.*t14.*t26.*t33.*2.0+Ixx3.*m2.*m3.*qp1.*qp3.*t5.*t18.*t20.*2.0-Ixx3.*m2.*m3.*qp1.*qp3.*t18.*t20.*t34.*2.0+Ixx3.*m2.*m3.*qp2.*qp3.*t18.*t20.*t45.*2.0-Iyy3.*m2.*m3.*qp1.*qp3.*t5.*t18.*t20.*2.0+Iyy3.*m2.*m3.*qp1.*qp3.*t18.*t20.*t34.*2.0+Iyy3.*m2.*m3.*qp2.*qp3.*t18.*t20.*t45.*2.0+Ixx2.*m2.*m3.*t7.*t18.*t20.*t30.*t34.*4.0;
et44 = Ixx3.*m2.*m3.*t7.*t18.*t20.*t30.*t34.*4.0-Iyy3.*m2.*m3.*t7.*t14.*t18.*t30.*t34.*4.0-Ixx1.*l2.*qp1.*qp3.*t5.*t6.*t22.*t26.*4.0-Ixx3.*l2.*qp1.*qp3.*t5.*t6.*t22.*t26.*4.0-Ixx2.*l2.*qp1.*qp3.*t6.*t22.*t26.*t34.*4.0+Ixx3.*l2.*qp1.*qp3.*t6.*t22.*t26.*t34.*4.0+Ixx2.*l2.*qp2.*qp3.*t8.*t22.*t26.*t33.*4.0+Ixx3.*l2.*qp1.*qp3.*t5.*t22.*t26.*t37.*4.0+Ixx3.*l2.*qp2.*qp3.*t8.*t22.*t26.*t33.*2.0-Ixx3.*l2.*qp1.*qp3.*t22.*t26.*t34.*t37.*4.0-Iyy3.*l2.*qp1.*qp3.*t5.*t6.*t22.*t26.*4.0+Iyy3.*l2.*qp1.*qp3.*t6.*t22.*t26.*t34.*4.0+Iyy3.*l2.*qp1.*qp3.*t5.*t22.*t26.*t37.*4.0-Iyy3.*l2.*qp2.*qp3.*t8.*t22.*t26.*t33.*2.0-Iyy3.*l2.*qp1.*qp3.*t22.*t26.*t34.*t37.*4.0-Izz2.*l2.*qp1.*qp3.*t5.*t6.*t22.*t26.*4.0+Izz3.*l2.*qp1.*qp3.*t5.*t6.*t22.*t26.*4.0+Izz2.*l2.*qp1.*qp3.*t6.*t22.*t26.*t34.*4.0;
et45 = Izz3.*l2.*qp1.*qp3.*t6.*t22.*t26.*t34.*-8.0-Izz2.*l2.*qp2.*qp3.*t8.*t22.*t26.*t33.*4.0-Izz3.*l2.*qp1.*qp3.*t5.*t22.*t26.*t37.*4.0+Izz3.*l2.*qp2.*qp3.*t8.*t22.*t26.*t33.*2.0+Izz3.*l2.*qp1.*qp3.*t22.*t26.*t34.*t37.*4.0-Iyy3.*lcm3.*qp1.*qp3.*t5.*t6.*t15.*t26.*4.0+Iyy3.*lcm3.*qp1.*qp3.*t6.*t15.*t26.*t34.*4.0-Iyy3.*lcm3.*qp2.*qp3.*t8.*t15.*t26.*t33.*4.0+Ixx1.*l2.*t5.*t6.*t7.*t22.*t26.*t30.*4.0+Ixx3.*l2.*t5.*t6.*t7.*t22.*t26.*t30.*2.0+Ixx3.*l2.*t5.*t6.*t7.*t22.*t26.*t32.*2.0+Ixx2.*l2.*t6.*t7.*t22.*t26.*t30.*t34.*4.0-Ixx3.*l2.*t5.*t7.*t22.*t26.*t30.*t37.*2.0+Ixx3.*l2.*t5.*t7.*t22.*t26.*t31.*t37.*4.0-Ixx3.*l2.*t5.*t7.*t22.*t26.*t32.*t37.*2.0-Ixx3.*l2.*t5.*t7.*t22.*t26.*t31.*t39.*4.0-Ixx3.*l2.*t7.*t22.*t26.*t30.*t34.*t37.*4.0+Ixx3.*l2.*t7.*t22.*t26.*t30.*t34.*t39.*4.0+Iyy3.*l2.*t5.*t6.*t7.*t22.*t26.*t30.*2.0;
et46 = Iyy3.*l2.*t5.*t6.*t7.*t22.*t26.*t32.*2.0-Iyy3.*l2.*t5.*t7.*t22.*t26.*t30.*t37.*2.0-Iyy3.*l2.*t5.*t7.*t22.*t26.*t32.*t37.*2.0+Izz2.*l2.*t5.*t6.*t7.*t22.*t26.*t30.*4.0-Izz3.*l2.*t5.*t6.*t7.*t22.*t26.*t30.*2.0-Izz3.*l2.*t5.*t6.*t7.*t22.*t26.*t32.*2.0-Izz2.*l2.*t6.*t7.*t22.*t26.*t30.*t34.*4.0+Izz3.*l2.*t6.*t7.*t22.*t26.*t30.*t34.*4.0+Izz3.*l2.*t5.*t7.*t22.*t26.*t30.*t37.*2.0-Izz3.*l2.*t5.*t7.*t22.*t26.*t31.*t37.*4.0+Izz3.*l2.*t5.*t7.*t22.*t26.*t32.*t37.*2.0+Izz3.*l2.*t5.*t7.*t22.*t26.*t31.*t39.*4.0+Izz3.*l2.*t7.*t22.*t26.*t30.*t34.*t37.*4.0-Izz3.*l2.*t7.*t22.*t26.*t30.*t34.*t39.*4.0+Iyy3.*lcm3.*t5.*t6.*t7.*t15.*t26.*t30.*4.0-Iyy3.*lcm3.*t6.*t7.*t15.*t26.*t30.*t34.*4.0-Ixx3.*m3.*t3.*t5.*t6.*t7.*t8.*t20.*2.0-Iyy3.*m3.*t3.*t5.*t6.*t7.*t8.*t20.*2.0+Izz3.*m3.*t3.*t5.*t6.*t7.*t8.*t20.*2.0;
et47 = Ixx3.*qp1.*qp2.*t6.*t7.*t8.*t11.*t33.*2.0+Ixx2.*qp2.*qp3.*t6.*t8.*t23.*t26.*t33.*4.0+Ixx3.*qp2.*qp3.*t6.*t8.*t23.*t26.*t33.*2.0-Ixx3.*qp2.*qp3.*t8.*t14.*t20.*t26.*t37.*4.0-Iyy3.*qp1.*qp2.*t6.*t7.*t8.*t10.*t33.*2.0+Iyy3.*qp1.*qp2.*t6.*t7.*t8.*t13.*t33.*2.0-Iyy3.*qp2.*qp3.*t6.*t8.*t23.*t26.*t33.*2.0-Izz3.*qp1.*qp2.*t6.*t7.*t8.*t11.*t33.*2.0-Izz2.*qp2.*qp3.*t6.*t8.*t23.*t26.*t33.*4.0+Ixx2.*t5.*t7.*t14.*t20.*t26.*t30.*t35.*2.0-Ixx2.*t7.*t14.*t20.*t26.*t30.*t34.*t35.*2.0-l2.*lcm3.*m3.*qp2.*qp3.*t8.*t11.*t33.*2.0-g.*lcm2.*m2.*t7.*t14.*t20.*t26.*t35.*2.0-g.*lcm2.*m2.*t7.*t23.*t26.*t33.*t35.*2.0+l2.*lcm3.*m3.*t5.*t7.*t10.*t31.*t37.*2.0-l2.*lcm3.*m3.*t5.*t7.*t10.*t31.*t39.*2.0+l2.*lcm3.*m3.*t5.*t7.*t13.*t31.*t37.*2.0-l2.*lcm3.*m3.*t5.*t7.*t13.*t31.*t39.*2.0;
et48 = l2.*lcm3.*m3.*t7.*t10.*t30.*t34.*t37.*-2.0+l2.*lcm3.*m3.*t7.*t10.*t30.*t34.*t39.*2.0-l2.*lcm3.*m3.*t7.*t13.*t30.*t34.*t37.*2.0+l2.*lcm3.*m3.*t7.*t13.*t30.*t34.*t39.*2.0+l2.*m2.*qp2.*qp3.*t8.*t18.*t22.*t26.*4.0-g.*m2.*t6.*t7.*t18.*t22.*t26.*t33.*2.0+m3.*qp2.*qp3.*t6.*t8.*t10.*t20.*t33.*2.0-m3.*qp2.*qp3.*t6.*t8.*t11.*t20.*t33.*2.0-m3.*qp2.*qp3.*t6.*t8.*t13.*t20.*t33.*2.0-l2.*t3.*t5.*t7.*t8.*t22.*t26.*t35.*2.0-m2.*t7.*t14.*t18.*t20.*t26.*t30.*t34.*4.0-qp2.*qp3.*t6.*t8.*t14.*t23.*t27.*t33.*4.0+qp2.*qp3.*t8.*t15.*t22.*t27.*t33.*t35.*4.0-qp1.*qp2.*t7.*t8.*t15.*t22.*t27.*t64.*4.0+qp2.*qp3.*t8.*t14.*t23.*t27.*t33.*t37.*4.0-t3.*t5.*t6.*t7.*t8.*t14.*t20.*t26.*2.0-Ixx1.*Iyy3.*l2.*lcm3.*m3.*qp1.*qp3.*t5.*t6.*4.0-Ixx3.*Iyy3.*l2.*lcm3.*m3.*qp1.*qp3.*t5.*t6.*4.0;
et49 = Ixx2.*Iyy3.*l2.*lcm3.*m3.*qp1.*qp3.*t6.*t34.*-4.0+Ixx3.*Iyy3.*l2.*lcm3.*m3.*qp1.*qp3.*t6.*t34.*4.0+Ixx2.*Iyy3.*l2.*lcm3.*m3.*qp2.*qp3.*t8.*t33.*4.0+Ixx3.*Iyy3.*l2.*lcm3.*m3.*qp1.*qp3.*t5.*t37.*4.0+Ixx3.*Iyy3.*l2.*lcm3.*m3.*qp2.*qp3.*t8.*t33.*2.0-Ixx3.*Iyy3.*l2.*lcm3.*m3.*qp1.*qp3.*t34.*t37.*4.0-Iyy3.*Izz2.*l2.*lcm3.*m3.*qp1.*qp3.*t5.*t6.*4.0+Iyy3.*Izz3.*l2.*lcm3.*m3.*qp1.*qp3.*t5.*t6.*4.0+Iyy3.*Izz2.*l2.*lcm3.*m3.*qp1.*qp3.*t6.*t34.*4.0-Iyy3.*Izz3.*l2.*lcm3.*m3.*qp1.*qp3.*t6.*t34.*8.0-Iyy3.*Izz2.*l2.*lcm3.*m3.*qp2.*qp3.*t8.*t33.*4.0-Iyy3.*Izz3.*l2.*lcm3.*m3.*qp1.*qp3.*t5.*t37.*4.0+Iyy3.*Izz3.*l2.*lcm3.*m3.*qp2.*qp3.*t8.*t33.*2.0+Iyy3.*Izz3.*l2.*lcm3.*m3.*qp1.*qp3.*t34.*t37.*4.0+Ixx1.*Iyy3.*l2.*lcm3.*m3.*t5.*t6.*t7.*t30.*4.0+Ixx3.*Iyy3.*l2.*lcm3.*m3.*t5.*t6.*t7.*t30.*2.0+Ixx3.*Iyy3.*l2.*lcm3.*m3.*t5.*t6.*t7.*t32.*2.0;
et50 = Ixx2.*Iyy3.*l2.*lcm3.*m3.*t6.*t7.*t30.*t34.*4.0-Ixx3.*Iyy3.*l2.*lcm3.*m3.*t5.*t7.*t30.*t37.*2.0-Ixx3.*Iyy3.*l2.*lcm3.*m3.*t5.*t7.*t32.*t37.*2.0-Ixx3.*Izz3.*l2.*lcm3.*m3.*t5.*t7.*t31.*t37.*4.0+Ixx3.*Izz3.*l2.*lcm3.*m3.*t5.*t7.*t31.*t39.*4.0+Ixx3.*Izz3.*l2.*lcm3.*m3.*t7.*t30.*t34.*t37.*4.0-Ixx3.*Izz3.*l2.*lcm3.*m3.*t7.*t30.*t34.*t39.*4.0+Iyy3.*Izz2.*l2.*lcm3.*m3.*t5.*t6.*t7.*t30.*4.0-Iyy3.*Izz3.*l2.*lcm3.*m3.*t5.*t6.*t7.*t30.*2.0-Iyy3.*Izz3.*l2.*lcm3.*m3.*t5.*t6.*t7.*t32.*2.0-Iyy3.*Izz2.*l2.*lcm3.*m3.*t6.*t7.*t30.*t34.*4.0+Iyy3.*Izz3.*l2.*lcm3.*m3.*t6.*t7.*t30.*t34.*4.0+Iyy3.*Izz3.*l2.*lcm3.*m3.*t5.*t7.*t30.*t37.*2.0+Iyy3.*Izz3.*l2.*lcm3.*m3.*t5.*t7.*t32.*t37.*2.0+Ixx2.*Ixx3.*m3.*qp2.*qp3.*t6.*t8.*t20.*t33.*4.0+Ixx2.*Iyy3.*m3.*qp2.*qp3.*t6.*t8.*t20.*t33.*4.0-Ixx3.*Izz2.*m3.*qp2.*qp3.*t6.*t8.*t20.*t33.*4.0;
et51 = Iyy3.*Izz2.*m3.*qp2.*qp3.*t6.*t8.*t20.*t33.*-4.0+Iyy3.*l2.*lcm3.*m2.*m3.*qp2.*qp3.*t8.*t18.*4.0-Ixx3.*g.*lcm2.*m2.*m3.*t7.*t20.*t33.*t35.*2.0-Iyy3.*g.*lcm3.*m2.*m3.*t6.*t7.*t18.*t33.*2.0-Iyy3.*g.*lcm2.*m2.*m3.*t7.*t20.*t33.*t35.*2.0+Izz3.*g.*lcm2.*m2.*m3.*t7.*t20.*t33.*t35.*2.0-Ixx3.*l2.*lcm3.*m3.*t3.*t5.*t7.*t8.*t35.*2.0+Izz3.*l2.*lcm3.*m3.*t3.*t5.*t7.*t8.*t35.*2.0+Ixx2.*l2.*qp1.*qp2.*t7.*t8.*t22.*t26.*t64.*4.0+Ixx3.*l2.*qp1.*qp2.*t7.*t8.*t22.*t26.*t64.*2.0-Iyy3.*l2.*qp1.*qp2.*t7.*t8.*t22.*t26.*t64.*2.0-Izz2.*l2.*qp1.*qp2.*t7.*t8.*t22.*t26.*t64.*4.0+Izz3.*l2.*qp1.*qp2.*t7.*t8.*t22.*t26.*t64.*2.0-Iyy3.*lcm3.*qp1.*qp2.*t7.*t8.*t15.*t26.*t64.*4.0-Ixx2.*qp1.*qp2.*t6.*t7.*t8.*t23.*t26.*t33.*4.0-Ixx3.*qp1.*qp2.*t6.*t7.*t8.*t23.*t26.*t33.*2.0+Iyy3.*qp1.*qp2.*t6.*t7.*t8.*t23.*t26.*t33.*2.0;
et52 = Iyy3.*qp2.*qp3.*t6.*t8.*t14.*t20.*t26.*t33.*-4.0+Izz2.*qp1.*qp2.*t6.*t7.*t8.*t23.*t26.*t33.*4.0-l2.*lcm3.*m3.*qp1.*qp2.*t7.*t8.*t11.*t64.*2.0+g.*lcm2.*m2.*t7.*t14.*t20.*t26.*t33.*t35.*2.0-l2.*m2.*qp1.*qp3.*t5.*t6.*t18.*t22.*t26.*4.0+l2.*m2.*qp1.*qp3.*t6.*t18.*t22.*t26.*t34.*4.0-l2.*m2.*qp2.*qp3.*t8.*t18.*t22.*t26.*t33.*4.0+l2.*m2.*t5.*t6.*t7.*t18.*t22.*t26.*t30.*4.0-l2.*m2.*t6.*t7.*t18.*t22.*t26.*t30.*t34.*4.0+l2.*qp1.*qp2.*t7.*t8.*t24.*t27.*t33.*t35.*4.0-l2.*qp1.*qp2.*t7.*t8.*t24.*t27.*t33.*t38.*4.0-m3.*qp1.*qp2.*t6.*t7.*t8.*t10.*t20.*t33.*2.0+m3.*qp1.*qp2.*t6.*t7.*t8.*t11.*t20.*t33.*2.0+m3.*qp1.*qp2.*t6.*t7.*t8.*t13.*t20.*t33.*2.0+qp1.*qp2.*t6.*t7.*t8.*t14.*t23.*t27.*t33.*8.0-qp1.*qp2.*t7.*t8.*t15.*t22.*t27.*t33.*t35.*4.0-qp1.*qp2.*t7.*t8.*t14.*t23.*t27.*t33.*t37.*8.0;
et53 = Ixx2.*Ixx3.*Iyy3.*qp1.*qp2.*t6.*t7.*t8.*t33.*-4.0+Ixx3.*Iyy3.*Izz2.*qp1.*qp2.*t6.*t7.*t8.*t33.*4.0+Ixx2.*Iyy3.*l2.*lcm3.*m3.*qp1.*qp2.*t7.*t8.*t64.*4.0+Ixx3.*Iyy3.*l2.*lcm3.*m3.*qp1.*qp2.*t7.*t8.*t64.*2.0-Iyy3.*Izz2.*l2.*lcm3.*m3.*qp1.*qp2.*t7.*t8.*t64.*4.0+Iyy3.*Izz3.*l2.*lcm3.*m3.*qp1.*qp2.*t7.*t8.*t64.*2.0-Ixx2.*Ixx3.*m3.*qp1.*qp2.*t6.*t7.*t8.*t20.*t33.*4.0-Ixx2.*Iyy3.*m3.*qp1.*qp2.*t6.*t7.*t8.*t20.*t33.*4.0+Ixx3.*Izz2.*m3.*qp1.*qp2.*t6.*t7.*t8.*t20.*t33.*4.0+Iyy3.*Izz2.*m3.*qp1.*qp2.*t6.*t7.*t8.*t20.*t33.*4.0-Iyy3.*l2.*lcm3.*m2.*m3.*qp1.*qp3.*t5.*t6.*t18.*4.0+Iyy3.*l2.*lcm3.*m2.*m3.*qp1.*qp3.*t6.*t18.*t34.*4.0-Iyy3.*l2.*lcm3.*m2.*m3.*qp2.*qp3.*t8.*t18.*t33.*4.0+Iyy3.*l2.*lcm3.*m2.*m3.*t5.*t6.*t7.*t18.*t30.*4.0-Iyy3.*l2.*lcm3.*m2.*m3.*t6.*t7.*t18.*t30.*t34.*4.0+Ixx3.*l2.*qp1.*qp2.*t7.*t8.*t22.*t26.*t33.*t35.*6.0;
et54 = Ixx3.*l2.*qp1.*qp2.*t7.*t8.*t22.*t26.*t33.*t38.*-8.0+Iyy3.*l2.*qp1.*qp2.*t7.*t8.*t22.*t26.*t33.*t35.*2.0-Izz3.*l2.*qp1.*qp2.*t7.*t8.*t22.*t26.*t33.*t35.*6.0+Izz3.*l2.*qp1.*qp2.*t7.*t8.*t22.*t26.*t33.*t38.*8.0+Iyy3.*qp1.*qp2.*t6.*t7.*t8.*t14.*t20.*t26.*t33.*6.0+l2.*lcm3.*m3.*qp1.*qp2.*t7.*t8.*t10.*t33.*t35.*2.0-l2.*lcm3.*m3.*qp1.*qp2.*t7.*t8.*t10.*t33.*t38.*4.0+l2.*lcm3.*m3.*qp1.*qp2.*t7.*t8.*t13.*t33.*t35.*2.0-l2.*lcm3.*m3.*qp1.*qp2.*t7.*t8.*t13.*t33.*t38.*4.0-l2.*m2.*qp1.*qp2.*t7.*t8.*t18.*t22.*t26.*t64.*4.0-Iyy3.*l2.*lcm3.*m2.*m3.*qp1.*qp2.*t7.*t8.*t18.*t64.*4.0+Ixx3.*Iyy3.*l2.*lcm3.*m3.*qp1.*qp2.*t7.*t8.*t33.*t35.*2.0-Ixx3.*Izz3.*l2.*lcm3.*m3.*qp1.*qp2.*t7.*t8.*t33.*t35.*4.0+Ixx3.*Izz3.*l2.*lcm3.*m3.*qp1.*qp2.*t7.*t8.*t33.*t38.*8.0-Iyy3.*Izz3.*l2.*lcm3.*m3.*qp1.*qp2.*t7.*t8.*t33.*t35.*2.0;
et55 = Ixx1.*Iyy2.*t3.*2.0+Ixx1.*Izz3.*t3.*2.0+Iyy2.*Iyy3.*t3.*2.0+Iyy2.*Izz2.*t3.*2.0+Iyy3.*Izz3.*t3.*2.0+Izz2.*Izz3.*t3.*2.0+t3.*t16.*t26.*2.0+t3.*t21.*t25.*2.0-t31.*t45.*t55-t31.*t45.*t57-t31.*t45.*t59-t31.*t45.*t61-t31.*t45.*t80-t31.*t45.*t81-t31.*t45.*t82-t31.*t45.*t83-t30.*t45.*t88.*4.0-t31.*t45.*t88.*4.0-t32.*t45.*t88-t30.*t45.*t91.*2.0-t30.*t45.*t92.*2.0-t31.*t45.*t91.*3.0-t30.*t45.*t93.*2.0-t31.*t45.*t92.*2.0-t30.*t45.*t94.*2.0-t31.*t45.*t93.*3.0-t32.*t45.*t92-t31.*t45.*t94.*2.0-t32.*t45.*t94-t31.*t45.*t96+Ixx1.*t13.*t31.*t45+Izz2.*t13.*t31.*t45+qp1.*qp2.*t5.*t40.*2.0+qp1.*qp2.*t5.*t41.*2.0;
et56 = qp1.*qp2.*t5.*t42.*-2.0-qp1.*qp2.*t5.*t43.*2.0+qp1.*qp2.*t5.*t50.*2.0-qp1.*qp2.*t5.*t51.*2.0-qp1.*qp2.*t5.*t52.*2.0+qp1.*qp2.*t5.*t54.*2.0-qp1.*qp2.*t5.*t56.*2.0-qp1.*qp2.*t5.*t58.*2.0-qp1.*qp2.*t5.*t59.*4.0-qp1.*qp2.*t5.*t61.*4.0-qp1.*qp2.*t5.*t66.*2.0-qp1.*qp2.*t5.*t67.*2.0+qp1.*qp2.*t5.*t68.*2.0-qp1.*qp2.*t5.*t71.*2.0+qp1.*qp2.*t34.*t42.*2.0+qp1.*qp2.*t34.*t43.*2.0-qp1.*qp2.*t5.*t73.*2.0+qp1.*qp2.*t5.*t77.*2.0+qp1.*qp2.*t34.*t51.*2.0-qp1.*qp2.*t5.*t81.*4.0+qp1.*qp2.*t34.*t52.*2.0-qp1.*qp2.*t5.*t82.*4.0-qp1.*qp2.*t5.*t83.*2.0+qp1.*qp2.*t34.*t56.*2.0+qp1.*qp2.*t34.*t58.*2.0-qp1.*qp2.*t5.*t88.*4.0+qp1.*qp2.*t34.*t59.*4.0+qp1.*qp2.*t34.*t61.*4.0-qp1.*qp2.*t5.*t92.*4.0-qp1.*qp2.*t5.*t93.*4.0;
et57 = qp1.*qp2.*t5.*t94.*-2.0-qp2.*qp3.*t44.*t53+qp1.*qp2.*t34.*t66.*2.0-qp1.*qp2.*t5.*t96.*4.0+qp1.*qp2.*t34.*t67.*2.0-qp1.*qp2.*t5.*t99.*2.0-qp2.*qp3.*t44.*t60+qp1.*qp2.*t34.*t73.*2.0+qp1.*qp2.*t5.*t103.*2.0-qp1.*qp2.*t5.*t104.*2.0-qp1.*qp2.*t34.*t77.*2.0+qp1.*qp2.*t5.*t108.*2.0-qp1.*qp2.*t5.*t110.*2.0+qp1.*qp2.*t34.*t81.*4.0+qp1.*qp2.*t34.*t82.*4.0+qp1.*qp2.*t5.*t112.*6.0+qp1.*qp2.*t34.*t83.*4.0-qp1.*qp2.*t5.*t115.*6.0+qp1.*qp2.*t34.*t88.*4.0+qp1.*qp2.*t5.*t120.*2.0-qp1.*qp2.*t5.*t121.*2.0+qp1.*qp2.*t34.*t92.*4.0+qp1.*qp2.*t34.*t93.*4.0+qp1.*qp2.*t34.*t94.*2.0+qp1.*qp2.*t5.*t124.*1.0e+1-qp2.*qp3.*t44.*t83+qp1.*qp2.*t34.*t96.*4.0-qp1.*qp2.*t5.*t129.*4.0-qp2.*qp3.*t44.*t94+qp1.*qp2.*t34.*t115.*6.0+qp1.*qp2.*t34.*t121.*2.0;
et58 = qp1.*qp2.*t34.*t124.*-1.0e+1+qp1.*qp2.*t34.*t129.*4.0-qp1.*qp2.*t5.*t160.*6.0-qp1.*qp2.*t5.*t163.*2.0+qp1.*qp2.*t5.*t166.*1.0e+1-qp1.*qp2.*t5.*t173.*1.2e+1+qp1.*qp2.*t5.*t174.*4.0+qp1.*qp2.*t5.*t175.*1.2e+1-qp1.*qp2.*t5.*t178.*6.0+qp1.*qp2.*t5.*t179.*1.6e+1+qp1.*qp2.*t5.*t181.*4.0-qp1.*qp2.*t5.*t182.*1.0e+1-qp1.*qp2.*t5.*t185.*1.6e+1-qp1.*qp2.*t5.*t189.*4.0+qp1.*qp2.*t34.*t160.*1.6e+1-qp1.*qp2.*t34.*t166.*1.6e+1+qp1.*qp2.*t34.*t173.*1.2e+1-qp1.*qp2.*t34.*t174.*4.0-qp1.*qp2.*t34.*t175.*1.2e+1+qp1.*qp2.*t34.*t178.*1.0e+1-qp1.*qp2.*t34.*t179.*2.0e+1-qp1.*qp2.*t34.*t181.*4.0+qp1.*qp2.*t34.*t182.*1.0e+1+qp1.*qp2.*t34.*t185.*2.0e+1+qp1.*qp2.*t34.*t189.*8.0+qp1.*qp2.*t5.*t245.*8.0-qp1.*qp2.*t34.*t245.*8.0+t3.*t14.*t20.*t26.*2.0;
et59 = t3.*t16.*t26.*t33.*-2.0-t3.*t21.*t25.*t33.*2.0+t3.*t23.*t26.*t35.*2.0+t6.*t8.*t30.*t70.*2.0-t6.*t8.*t30.*t72.*2.0+t6.*t8.*t30.*t76.*2.0+t8.*t31.*t37.*t57.*4.0+t8.*t31.*t37.*t61.*4.0-t6.*t8.*t31.*t106.*2.0+t6.*t8.*t30.*t109.*2.0-t6.*t8.*t31.*t109.*4.0-t6.*t8.*t30.*t113.*2.0+t6.*t8.*t30.*t114.*2.0-t6.*t8.*t31.*t113.*2.0+t8.*t31.*t37.*t83.*4.0-t6.*t8.*t31.*t116.*4.0+t6.*t8.*t30.*t118.*2.0+t6.*t8.*t31.*t118.*2.0+t6.*t8.*t30.*t122.*4.0+t6.*t8.*t30.*t123.*4.0+t6.*t8.*t31.*t123.*2.0+t8.*t30.*t37.*t94.*4.0+t8.*t31.*t37.*t94.*1.0e+1+t8.*t32.*t37.*t94.*2.0+t6.*t8.*t30.*t128.*2.0-t6.*t8.*t31.*t128.*2.0+t6.*t8.*t30.*t130.*2.0-t6.*t8.*t31.*t130.*2.0+t8.*t31.*t37.*t109.*4.0+t8.*t31.*t37.*t113.*4.0-t8.*t30.*t37.*t123.*4.0;
et60 = t8.*t31.*t37.*t123.*-4.0-t6.*t8.*t31.*t158.*2.0-t6.*t8.*t31.*t159.*4.0+t8.*t31.*t37.*t128.*2.0+t6.*t8.*t30.*t161.*2.0+t6.*t8.*t31.*t161.*2.0+t6.*t8.*t30.*t164.*2.0+t6.*t8.*t30.*t165.*2.0+t6.*t8.*t31.*t164.*2.0+t6.*t8.*t31.*t165.*4.0+t6.*t8.*t30.*t172.*1.6e+1+t6.*t8.*t31.*t172.*8.0+t6.*t8.*t32.*t172.*2.0-t6.*t8.*t30.*t176.*2.0+t6.*t8.*t30.*t177.*2.0-t6.*t8.*t31.*t176.*6.0-t6.*t8.*t31.*t177.*2.0+t6.*t8.*t30.*t180.*1.0e+1+t6.*t8.*t31.*t180.*4.0+t6.*t8.*t32.*t180.*2.0+t6.*t8.*t30.*t183.*8.0+t6.*t8.*t30.*t184.*6.0+t6.*t8.*t31.*t183.*6.0+t6.*t8.*t32.*t184.*2.0+t6.*t8.*t30.*t188.*2.0-t6.*t8.*t31.*t187.*2.0+t6.*t8.*t31.*t188.*2.0+t8.*t30.*t37.*t159.*4.0+t8.*t31.*t37.*t159.*8.0-t8.*t30.*t37.*t165.*4.0;
et61 = t8.*t31.*t37.*t165.*-8.0+t8.*t30.*t37.*t177.*1.4e+1+t8.*t31.*t37.*t177.*1.2e+1+t8.*t32.*t37.*t177.*2.0-t8.*t30.*t37.*t184.*1.4e+1-t8.*t31.*t37.*t184.*1.2e+1-t8.*t32.*t37.*t184.*2.0+t8.*t30.*t37.*t187.*2.0+t8.*t31.*t37.*t187.*4.0+t6.*t8.*t32.*t250+Ixx1.*Ixx3.*t3.*t35.*2.0+Ixx2.*Iyy2.*t3.*t33.*2.0+Ixx3.*Iyy2.*t3.*t33.*2.0+Ixx3.*Iyy3.*t3.*t35.*2.0+Iyy2.*Iyy3.*t1.*t7.*2.0+Ixx2.*Izz3.*t3.*t33.*2.0-Iyy2.*Iyy3.*t3.*t33.*2.0-Ixx1.*Izz3.*t3.*t35.*2.0+Ixx3.*Izz3.*t3.*t33.*2.0+Ixx3.*Izz2.*t3.*t35.*2.0+Iyy3.*Izz3.*t1.*t7.*2.0-Iyy2.*Izz2.*t3.*t33.*2.0-Iyy3.*Izz3.*t3.*t33.*2.0-Iyy3.*Izz3.*t3.*t35.*2.0-Izz2.*Izz3.*t3.*t33.*2.0-Izz2.*Izz3.*t3.*t35.*2.0+Ixx1.*m3.*t3.*t14.*2.0+Ixx1.*m2.*t3.*t18.*2.0+Iyy2.*m3.*t3.*t14.*2.0+Iyy3.*m3.*t3.*t14.*2.0;
et62 = Iyy2.*m2.*t3.*t18.*2.0+Iyy3.*m2.*t3.*t18.*2.0+Iyy2.*m3.*t3.*t20.*2.0+Izz2.*m3.*t3.*t14.*2.0+Izz3.*m3.*t3.*t14.*2.0+Izz2.*m2.*t3.*t18.*2.0+Izz3.*m2.*t3.*t18.*2.0+Izz3.*m3.*t3.*t20.*2.0-Ixx1.*Ixx3.*Iyy2.*t31.*t45-Ixx1.*Ixx3.*Izz3.*t31.*t45+Ixx1.*Iyy2.*Izz3.*t31.*t45-Ixx3.*Iyy2.*Izz2.*t31.*t45-Ixx3.*Izz2.*Izz3.*t31.*t45+Iyy2.*Izz2.*Izz3.*t31.*t45+Ixx2.*Ixx3.*t3.*t33.*t35.*2.0+Ixx3.*Iyy3.*t1.*t7.*t35.*2.0-Ixx3.*Iyy2.*t3.*t33.*t35.*2.0-Ixx3.*Iyy3.*t3.*t33.*t35.*2.0-Ixx2.*Izz3.*t3.*t33.*t35.*2.0-Ixx3.*Izz2.*t3.*t33.*t35.*2.0-Iyy3.*Izz3.*t1.*t7.*t35.*2.0+Iyy2.*Izz3.*t3.*t33.*t35.*2.0+Iyy3.*Izz3.*t3.*t33.*t35.*2.0+Izz2.*Izz3.*t3.*t33.*t35.*2.0+Ixx2.*m3.*t3.*t14.*t33.*2.0+Ixx3.*m3.*t3.*t14.*t33.*2.0+Ixx2.*m2.*t3.*t18.*t33.*2.0+Ixx3.*m3.*t3.*t14.*t35.*2.0;
et63 = Ixx3.*m2.*t3.*t18.*t33.*2.0+Ixx3.*m2.*t3.*t18.*t35.*2.0+Ixx1.*m3.*t3.*t20.*t35.*2.0+Ixx3.*m3.*t3.*t20.*t35.*2.0+Iyy3.*m3.*t1.*t7.*t14.*2.0+Iyy3.*m2.*t1.*t7.*t18.*2.0+Iyy2.*m3.*t1.*t7.*t20.*2.0-Iyy2.*m3.*t3.*t14.*t33.*2.0-Iyy3.*m3.*t3.*t14.*t33.*2.0-Iyy2.*m2.*t3.*t18.*t33.*2.0-Iyy3.*m2.*t3.*t18.*t33.*2.0+Iyy3.*m3.*t3.*t20.*t35.*2.0+Izz3.*m3.*t1.*t7.*t20.*2.0-Izz2.*m3.*t3.*t14.*t33.*2.0-Izz3.*m3.*t3.*t14.*t33.*2.0-Izz2.*m2.*t3.*t18.*t33.*2.0-Izz3.*m3.*t3.*t14.*t35.*2.0-Izz3.*m2.*t3.*t18.*t33.*2.0-Izz3.*m2.*t3.*t18.*t35.*2.0+Izz2.*m3.*t3.*t20.*t35.*2.0-Izz3.*m3.*t3.*t20.*t35.*2.0+Ixx1.*qp1.*qp2.*t5.*t13.*2.0+Ixx2.*qp1.*qp2.*t13.*t34.*2.0+Ixx3.*qp1.*qp2.*t13.*t34.*2.0-Iyy2.*qp1.*qp2.*t5.*t11.*2.0+Iyy3.*qp1.*qp2.*t5.*t13.*2.0;
et64 = Iyy2.*qp1.*qp2.*t10.*t34.*-2.0+Iyy2.*qp1.*qp2.*t11.*t34.*2.0-Iyy3.*qp1.*qp2.*t13.*t34.*2.0+Iyy2.*qp2.*qp3.*t11.*t44-Iyy3.*qp2.*qp3.*t13.*t44-Izz3.*qp1.*qp2.*t5.*t11.*2.0+Izz2.*qp1.*qp2.*t5.*t13.*2.0-Izz3.*qp1.*qp2.*t10.*t34.*2.0+Izz3.*qp1.*qp2.*t11.*t34.*2.0-Izz2.*qp1.*qp2.*t13.*t34.*2.0+Izz3.*qp2.*qp3.*t11.*t44-Ixx1.*t8.*t10.*t31.*t37.*2.0-Ixx1.*t8.*t13.*t31.*t37.*2.0-Ixx3.*t16.*t26.*t31.*t45-Ixx3.*t21.*t25.*t31.*t45-Izz2.*t8.*t10.*t31.*t37.*2.0-Izz2.*t8.*t13.*t31.*t37.*2.0+Izz3.*t16.*t26.*t31.*t45+Izz3.*t21.*t25.*t31.*t45+m2.*m3.*t3.*t14.*t18.*4.0+m2.*m3.*t3.*t18.*t20.*2.0+l2.*t3.*t6.*t22.*t26.*4.0+l2.*t3.*t22.*t26.*t37.*4.0-l2.*t8.*t24.*t27.*t30.*2.0-l2.*t8.*t24.*t27.*t32.*2.0+l2.*t24.*t27.*t30.*t49.*2.0+l2.*t24.*t27.*t32.*t49.*2.0;
et65 = lcm3.*t3.*t6.*t15.*t26.*8.0-lcm3.*t8.*t17.*t27.*t30.*2.0-lcm3.*t8.*t17.*t27.*t31.*2.0+m3.*t13.*t14.*t31.*t45+m2.*t13.*t18.*t31.*t45+qp1.*qp2.*t5.*t35.*t55.*4.0+qp1.*qp2.*t5.*t35.*t59.*4.0-qp1.*qp2.*t5.*t38.*t57.*8.0-qp1.*qp2.*t5.*t38.*t61.*8.0-qp2.*qp3.*t5.*t7.*t99.*4.0+qp2.*qp3.*t5.*t7.*t103.*4.0+qp1.*qp2.*t5.*t35.*t80.*4.0+qp1.*qp2.*t5.*t35.*t81.*4.0+qp1.*qp2.*t5.*t35.*t82.*4.0-qp2.*qp3.*t5.*t7.*t110.*4.0-qp1.*qp2.*t5.*t38.*t83.*8.0-qp1.*qp2.*t34.*t35.*t59.*4.0+qp1.*qp2.*t5.*t35.*t91.*1.2e+1+qp1.*qp2.*t5.*t35.*t93.*4.0+qp1.*qp2.*t34.*t38.*t61.*8.0+qp1.*qp2.*t5.*t35.*t94.*1.8e+1+qp2.*qp3.*t5.*t7.*t120.*4.0+qp1.*qp2.*t5.*t35.*t96.*4.0+qp2.*qp3.*t5.*t7.*t132-qp1.*qp2.*t34.*t35.*t81.*4.0-qp1.*qp2.*t34.*t35.*t82.*4.0;
et66 = qp2.*qp3.*t5.*t7.*t140+qp1.*qp2.*t34.*t38.*t83.*1.6e+1-qp1.*qp2.*t34.*t35.*t93.*4.0-qp1.*qp2.*t34.*t35.*t94.*1.0e+1-qp1.*qp2.*t34.*t35.*t96.*4.0-qp2.*qp3.*t5.*t7.*t160.*4.0-qp2.*qp3.*t5.*t7.*t163.*4.0+qp2.*qp3.*t5.*t7.*t166.*4.0-qp2.*qp3.*t5.*t7.*t178.*8.0+qp2.*qp3.*t5.*t7.*t182.*4.0-qp2.*qp3.*t5.*t7.*t189.*4.0+t1.*t7.*t14.*t20.*t26.*2.0+t1.*t7.*t23.*t26.*t35.*2.0-t3.*t14.*t20.*t26.*t33.*2.0+t3.*t14.*t20.*t26.*t35.*1.0e+1-t8.*t15.*t22.*t27.*t30.*1.2e+1-t8.*t15.*t22.*t27.*t31.*1.2e+1-t8.*t15.*t22.*t27.*t32.*6.0-t3.*t23.*t26.*t33.*t35.*2.0-t6.*t8.*t30.*t36.*t43.*2.0+t6.*t8.*t30.*t33.*t55.*2.0+t6.*t8.*t30.*t33.*t57.*2.0-t6.*t8.*t30.*t36.*t59.*2.0-t14.*t23.*t27.*t30.*t45.*2.0-t6.*t8.*t30.*t36.*t61.*4.0;
et67 = t14.*t23.*t27.*t32.*t45.*-2.0+t15.*t22.*t27.*t30.*t49.*1.0e+1+t15.*t22.*t27.*t31.*t49.*1.2e+1+t15.*t22.*t27.*t32.*t49.*4.0+t6.*t8.*t30.*t33.*t80.*2.0-t6.*t8.*t30.*t36.*t81.*2.0-t6.*t8.*t30.*t36.*t82.*2.0-t6.*t8.*t30.*t36.*t83.*4.0-t8.*t30.*t33.*t37.*t57.*4.0+t6.*t8.*t30.*t33.*t91.*6.0-t6.*t8.*t30.*t36.*t88.*8.0-t6.*t8.*t30.*t36.*t92.*6.0+t8.*t30.*t36.*t37.*t61.*4.0-t6.*t8.*t30.*t36.*t93.*4.0-t6.*t8.*t30.*t36.*t94.*2.0-t6.*t8.*t30.*t36.*t96.*2.0+t8.*t30.*t36.*t37.*t83.*8.0+t8.*t30.*t36.*t37.*t94.*1.2e+1+l2.*lcm3.*m3.*t8.*t13.*t31.*2.0-l2.*lcm3.*m3.*t13.*t31.*t49.*2.0+g.*lcm3.*t5.*t8.*t16.*t27.*2.0-g.*lcm3.*t8.*t16.*t27.*t34.*2.0+m2.*m3.*t1.*t7.*t18.*t20.*2.0-m2.*m3.*t3.*t14.*t18.*t33.*4.0+m2.*m3.*t3.*t18.*t20.*t35.*2.0;
et68 = m3.*qp1.*qp2.*t5.*t11.*t14.*-2.0+m3.*qp1.*qp2.*t5.*t13.*t14.*2.0-m2.*qp1.*qp2.*t5.*t11.*t18.*2.0+m2.*qp1.*qp2.*t5.*t13.*t18.*2.0+m3.*qp1.*qp2.*t5.*t13.*t20.*2.0-m3.*qp1.*qp2.*t10.*t14.*t34.*2.0+m3.*qp1.*qp2.*t11.*t14.*t34.*2.0-m2.*qp1.*qp2.*t10.*t18.*t34.*2.0-m3.*qp1.*qp2.*t13.*t14.*t34.*2.0+m2.*qp1.*qp2.*t11.*t18.*t34.*2.0-m2.*qp1.*qp2.*t13.*t18.*t34.*2.0+m3.*qp2.*qp3.*t11.*t14.*t44+m2.*qp2.*qp3.*t11.*t18.*t44-m3.*qp2.*qp3.*t13.*t20.*t44+l2.*t1.*t6.*t7.*t22.*t26.*4.0-l2.*t3.*t6.*t22.*t26.*t33.*4.0+l2.*t1.*t7.*t22.*t26.*t37.*2.0-l2.*t3.*t22.*t26.*t33.*t37.*4.0-l2.*t8.*t24.*t27.*t31.*t38.*2.0+lcm3.*t1.*t6.*t7.*t15.*t26.*2.0-lcm3.*t3.*t6.*t15.*t26.*t33.*8.0+lcm3.*t8.*t17.*t27.*t30.*t33.*4.0+lcm3.*t8.*t17.*t27.*t31.*t33.*2.0;
et69 = lcm3.*t8.*t17.*t27.*t30.*t36.*-2.0-m3.*t8.*t10.*t14.*t31.*t37.*2.0-m2.*t8.*t10.*t18.*t31.*t37.*2.0-m3.*t8.*t13.*t14.*t31.*t37.*2.0-m2.*t8.*t13.*t18.*t31.*t37.*2.0-qp1.*qp3.*t6.*t7.*t8.*t70.*4.0+qp1.*qp3.*t6.*t7.*t8.*t88.*4.0+qp1.*qp3.*t6.*t7.*t8.*t92.*4.0+qp1.*qp3.*t6.*t7.*t8.*t94.*4.0-qp1.*qp3.*t6.*t7.*t8.*t98.*4.0+qp1.*qp3.*t6.*t7.*t8.*t102.*4.0-qp1.*qp3.*t6.*t7.*t8.*t107.*4.0-qp1.*qp3.*t6.*t7.*t8.*t109.*4.0-qp1.*qp3.*t6.*t7.*t8.*t114.*4.0+qp1.*qp3.*t6.*t7.*t8.*t119.*4.0+qp2.*qp3.*t5.*t7.*t35.*t94.*8.0-qp1.*qp3.*t6.*t7.*t8.*t122.*4.0-qp1.*qp3.*t7.*t8.*t37.*t94.*4.0-qp1.*qp3.*t6.*t7.*t8.*t128.*4.0-qp1.*qp3.*t6.*t7.*t8.*t130.*2.0-qp1.*qp3.*t6.*t7.*t8.*t159.*4.0-qp1.*qp3.*t6.*t7.*t8.*t162.*4.0;
et70 = qp1.*qp3.*t6.*t7.*t8.*t165.*4.0-qp1.*qp3.*t6.*t7.*t8.*t172.*4.0-qp1.*qp3.*t6.*t7.*t8.*t177.*6.0-qp1.*qp3.*t6.*t7.*t8.*t180.*4.0+qp1.*qp3.*t6.*t7.*t8.*t184.*2.0-qp1.*qp3.*t6.*t7.*t8.*t187.*4.0-qp1.*qp3.*t7.*t8.*t37.*t177.*4.0+qp1.*qp3.*t7.*t8.*t37.*t184.*4.0+t1.*t7.*t14.*t20.*t26.*t35.*4.0-t3.*t14.*t20.*t26.*t33.*t35.*1.0e+1+t8.*t15.*t22.*t27.*t30.*t33.*2.0+t8.*t15.*t22.*t27.*t32.*t33.*2.0-t8.*t14.*t23.*t27.*t30.*t37.*4.0-t8.*t14.*t23.*t27.*t31.*t37.*8.0-t8.*t14.*t23.*t27.*t32.*t37.*2.0-Ixx1.*Ixx3.*Iyy2.*qp1.*qp2.*t5.*2.0-Ixx2.*Ixx3.*Iyy2.*qp1.*qp2.*t34.*2.0-Ixx1.*Ixx3.*Izz3.*qp1.*qp2.*t5.*2.0+Ixx2.*Iyy2.*Iyy3.*qp1.*qp2.*t5.*4.0+Ixx3.*Iyy2.*Iyy3.*qp1.*qp2.*t5.*2.0-Ixx2.*Iyy2.*Iyy3.*qp1.*qp2.*t34.*2.0-Ixx2.*Ixx3.*Izz3.*qp1.*qp2.*t34.*2.0+Ixx3.*Iyy2.*Iyy3.*qp2.*qp3.*t44;
et71 = Ixx1.*Iyy2.*Izz3.*qp1.*qp2.*t5.*2.0-Ixx3.*Iyy2.*Izz2.*qp1.*qp2.*t5.*2.0+Ixx2.*Iyy3.*Izz3.*qp1.*qp2.*t5.*4.0+Ixx3.*Iyy3.*Izz3.*qp1.*qp2.*t5.*2.0+Ixx2.*Iyy2.*Izz3.*qp1.*qp2.*t34.*2.0+Ixx3.*Iyy2.*Izz2.*qp1.*qp2.*t34.*2.0-Ixx2.*Iyy3.*Izz3.*qp1.*qp2.*t34.*2.0+Ixx3.*Iyy2.*Izz3.*qp1.*qp2.*t34.*2.0+Ixx3.*Iyy3.*Izz3.*qp2.*qp3.*t44-Ixx3.*Izz2.*Izz3.*qp1.*qp2.*t5.*2.0+Iyy2.*Iyy3.*Izz3.*qp1.*qp2.*t5.*2.0+Ixx3.*Izz2.*Izz3.*qp1.*qp2.*t34.*2.0-Iyy2.*Iyy3.*Izz3.*qp1.*qp2.*t34.*2.0-Iyy2.*Iyy3.*Izz3.*qp2.*qp3.*t44+Iyy2.*Izz2.*Izz3.*qp1.*qp2.*t5.*2.0-Iyy2.*Izz2.*Izz3.*qp1.*qp2.*t34.*2.0+Ixx1.*Ixx3.*Izz3.*t8.*t31.*t37.*4.0+Ixx3.*Izz2.*Izz3.*t8.*t31.*t37.*4.0-Ixx1.*Ixx3.*m3.*t14.*t31.*t45-Ixx1.*Ixx3.*m2.*t18.*t31.*t45-Ixx3.*Iyy2.*m3.*t14.*t31.*t45-Ixx3.*Iyy2.*m2.*t18.*t31.*t45+Ixx1.*Izz3.*m3.*t14.*t31.*t45;
et72 = -Ixx3.*Izz2.*m3.*t14.*t31.*t45-Ixx3.*Izz3.*m3.*t14.*t31.*t45+Ixx1.*Izz3.*m2.*t18.*t31.*t45-Ixx3.*Izz2.*m2.*t18.*t31.*t45-Ixx3.*Izz3.*m2.*t18.*t31.*t45+Iyy2.*Izz3.*m3.*t14.*t31.*t45+Iyy2.*Izz3.*m2.*t18.*t31.*t45+Izz2.*Izz3.*m3.*t14.*t31.*t45+Izz2.*Izz3.*m2.*t18.*t31.*t45+Ixx1.*l2.*lcm3.*m3.*t3.*t6.*4.0+Ixx3.*l2.*lcm3.*m3.*t3.*t37.*4.0+Iyy2.*l2.*lcm3.*m3.*t3.*t6.*4.0+Iyy3.*l2.*lcm3.*m3.*t3.*t6.*4.0+Izz2.*l2.*lcm3.*m3.*t3.*t6.*4.0+Izz3.*l2.*lcm3.*m3.*t3.*t6.*4.0-Izz3.*l2.*lcm3.*m3.*t3.*t37.*4.0+Iyy2.*g.*t5.*t8.*t22.*t26.*2.0+Izz3.*g.*t5.*t8.*t22.*t26.*2.0-Ixx1.*l2.*t8.*t22.*t26.*t30.*2.0-Ixx1.*l2.*t8.*t22.*t26.*t31.*6.0-Ixx3.*l2.*t8.*t22.*t26.*t30.*2.0-Ixx3.*l2.*t8.*t22.*t26.*t32.*2.0+Ixx1.*l2.*t22.*t26.*t30.*t49.*2.0+Ixx1.*l2.*t22.*t26.*t31.*t49.*6.0;
et73 = Ixx3.*l2.*t22.*t26.*t30.*t49.*2.0+Ixx3.*l2.*t22.*t26.*t32.*t49.*2.0-Iyy2.*l2.*t8.*t22.*t26.*t30.*2.0-Iyy2.*l2.*t8.*t22.*t26.*t31.*2.0-Iyy3.*l2.*t8.*t22.*t26.*t30.*2.0-Iyy2.*l2.*t8.*t22.*t26.*t32.*2.0-Iyy3.*l2.*t8.*t22.*t26.*t32.*2.0+Iyy2.*l2.*t22.*t26.*t31.*t49.*2.0+Iyy3.*l2.*t22.*t26.*t30.*t49.*2.0+Iyy3.*l2.*t22.*t26.*t32.*t49.*2.0-Izz2.*l2.*t8.*t22.*t26.*t30.*2.0-Izz2.*l2.*t8.*t22.*t26.*t31.*6.0-Izz3.*l2.*t8.*t22.*t26.*t31.*2.0+Izz2.*l2.*t22.*t26.*t30.*t49.*2.0+Izz2.*l2.*t22.*t26.*t31.*t49.*6.0-Izz3.*l2.*t22.*t26.*t30.*t49.*2.0+Izz3.*l2.*t22.*t26.*t31.*t49.*2.0-Izz3.*l2.*t22.*t26.*t32.*t49.*2.0-Ixx1.*lcm3.*t8.*t15.*t26.*t30.*2.0-Ixx1.*lcm3.*t8.*t15.*t26.*t31.*2.0-Ixx3.*lcm3.*t8.*t15.*t26.*t30.*2.0-Ixx3.*lcm3.*t8.*t15.*t26.*t31.*8.0+Ixx3.*lcm3.*t15.*t26.*t30.*t49.*2.0;
et74 = Ixx3.*lcm3.*t15.*t26.*t31.*t49.*8.0-Iyy2.*lcm3.*t8.*t15.*t26.*t30.*2.0-Iyy2.*lcm3.*t8.*t15.*t26.*t31.*2.0-Iyy3.*lcm3.*t8.*t15.*t26.*t30.*2.0-Iyy3.*lcm3.*t8.*t15.*t26.*t32.*2.0-Izz2.*lcm3.*t8.*t15.*t26.*t30.*2.0-Izz2.*lcm3.*t8.*t15.*t26.*t31.*2.0+Izz3.*lcm3.*t8.*t15.*t26.*t31.*6.0-Izz3.*lcm3.*t15.*t26.*t30.*t49.*2.0-Izz3.*lcm3.*t15.*t26.*t31.*t49.*8.0+Ixx3.*m3.*t1.*t7.*t20.*t35.*2.0-Ixx3.*m3.*t3.*t14.*t33.*t35.*4.0-Ixx3.*m2.*t3.*t18.*t33.*t35.*4.0+Ixx2.*m3.*t3.*t20.*t33.*t35.*2.0-Ixx3.*m3.*t3.*t20.*t33.*t35.*2.0+Iyy3.*m3.*t1.*t7.*t20.*t35.*2.0-Iyy2.*m3.*t3.*t20.*t33.*t35.*2.0-Iyy3.*m3.*t3.*t20.*t33.*t35.*2.0-Izz3.*m3.*t1.*t7.*t20.*t35.*2.0+Izz3.*m3.*t3.*t14.*t33.*t35.*4.0+Izz3.*m2.*t3.*t18.*t33.*t35.*4.0-Izz2.*m3.*t3.*t20.*t33.*t35.*2.0;
et75 = Izz3.*m3.*t3.*t20.*t33.*t35.*2.0-Ixx3.*qp1.*qp2.*t5.*t16.*t26.*2.0-Ixx1.*qp1.*qp2.*t5.*t10.*t35.*2.0+Ixx1.*qp1.*qp2.*t5.*t10.*t38.*4.0-Ixx1.*qp1.*qp2.*t5.*t13.*t35.*6.0-Ixx3.*qp1.*qp2.*t5.*t11.*t35.*2.0-Ixx3.*qp1.*qp2.*t5.*t21.*t25.*2.0+Ixx1.*qp1.*qp2.*t5.*t13.*t38.*4.0+Ixx3.*qp1.*qp2.*t16.*t26.*t34.*2.0-Ixx2.*qp1.*qp2.*t10.*t34.*t35.*2.0+Ixx3.*qp1.*qp2.*t11.*t34.*t35.*2.0+Ixx3.*qp1.*qp2.*t21.*t25.*t34.*2.0+Ixx2.*qp1.*qp2.*t10.*t34.*t38.*4.0-Ixx2.*qp1.*qp2.*t13.*t34.*t35.*6.0-Ixx3.*qp1.*qp2.*t13.*t34.*t35.*4.0+Ixx2.*qp1.*qp2.*t13.*t34.*t38.*4.0+Iyy3.*qp1.*qp2.*t5.*t10.*t35.*2.0-Iyy3.*qp1.*qp2.*t5.*t13.*t35.*2.0+Iyy2.*qp1.*qp2.*t10.*t34.*t35.*6.0-Iyy3.*qp1.*qp2.*t10.*t34.*t35.*2.0-Iyy2.*qp1.*qp2.*t10.*t34.*t38.*4.0+Iyy2.*qp1.*qp2.*t13.*t34.*t35.*2.0+Iyy3.*qp1.*qp2.*t13.*t34.*t35.*2.0;
et76 = Iyy2.*qp1.*qp2.*t13.*t34.*t38.*-4.0+Iyy2.*qp2.*qp3.*t23.*t26.*t44.*2.0+Izz3.*qp1.*qp2.*t5.*t16.*t26.*2.0-Izz2.*qp1.*qp2.*t5.*t10.*t35.*2.0+Izz3.*qp1.*qp2.*t5.*t11.*t35.*2.0+Izz3.*qp1.*qp2.*t5.*t21.*t25.*2.0+Izz2.*qp1.*qp2.*t5.*t10.*t38.*4.0-Izz2.*qp1.*qp2.*t5.*t13.*t35.*6.0+Izz2.*qp1.*qp2.*t5.*t13.*t38.*4.0-Izz3.*qp1.*qp2.*t16.*t26.*t34.*2.0+Izz2.*qp1.*qp2.*t10.*t34.*t35.*2.0+Izz3.*qp1.*qp2.*t10.*t34.*t35.*4.0-Izz3.*qp1.*qp2.*t11.*t34.*t35.*2.0-Izz3.*qp1.*qp2.*t21.*t25.*t34.*2.0-Izz2.*qp1.*qp2.*t10.*t34.*t38.*4.0+Izz2.*qp1.*qp2.*t13.*t34.*t35.*6.0-Izz2.*qp1.*qp2.*t13.*t34.*t38.*4.0+Izz3.*qp2.*qp3.*t23.*t26.*t44.*2.0-Ixx1.*t6.*t8.*t13.*t30.*t33.*2.0-Ixx3.*t6.*t8.*t11.*t30.*t33.*2.0+Ixx2.*t6.*t8.*t13.*t31.*t33.*2.0+Ixx3.*t6.*t8.*t11.*t30.*t36.*2.0+Ixx3.*t6.*t8.*t13.*t31.*t33.*2.0;
et77 = Ixx2.*t6.*t8.*t13.*t30.*t36.*-2.0-Ixx3.*t6.*t8.*t13.*t30.*t36.*2.0+Ixx1.*t8.*t10.*t30.*t33.*t37.*2.0-Ixx2.*t8.*t10.*t31.*t33.*t37.*2.0+Ixx1.*t8.*t13.*t30.*t33.*t37.*2.0+Ixx2.*t8.*t10.*t30.*t36.*t37.*2.0-Ixx2.*t8.*t13.*t31.*t33.*t37.*2.0-Ixx1.*t8.*t23.*t26.*t31.*t37.*2.0+Ixx2.*t8.*t13.*t30.*t36.*t37.*2.0-Iyy2.*t6.*t8.*t10.*t31.*t33.*2.0+Iyy3.*t6.*t8.*t10.*t30.*t33.*2.0+Iyy2.*t6.*t8.*t10.*t30.*t36.*2.0-Iyy3.*t6.*t8.*t10.*t30.*t36.*2.0-Iyy3.*t6.*t8.*t13.*t30.*t33.*2.0+Iyy3.*t6.*t8.*t13.*t30.*t36.*2.0+Iyy2.*t8.*t10.*t31.*t33.*t37.*2.0-Iyy2.*t8.*t10.*t30.*t36.*t37.*2.0+Iyy2.*t8.*t13.*t31.*t33.*t37.*2.0-Iyy2.*t8.*t13.*t30.*t36.*t37.*2.0-Iyy3.*t14.*t20.*t26.*t30.*t45.*2.0-Iyy3.*t14.*t20.*t26.*t32.*t45.*2.0-Izz3.*t6.*t8.*t10.*t31.*t33.*2.0+Izz3.*t6.*t8.*t11.*t30.*t33.*2.0;
et78 = Izz2.*t6.*t8.*t13.*t30.*t33.*-2.0-Izz2.*t6.*t8.*t13.*t31.*t33.*2.0+Izz3.*t6.*t8.*t10.*t30.*t36.*2.0-Izz3.*t6.*t8.*t11.*t30.*t36.*2.0+Izz2.*t6.*t8.*t13.*t30.*t36.*2.0+Izz2.*t8.*t10.*t30.*t33.*t37.*2.0+Izz2.*t8.*t10.*t31.*t33.*t37.*2.0-Izz2.*t8.*t10.*t30.*t36.*t37.*2.0+Izz2.*t8.*t13.*t30.*t33.*t37.*2.0+Izz2.*t8.*t13.*t31.*t33.*t37.*2.0-Izz2.*t8.*t13.*t30.*t36.*t37.*2.0-Izz2.*t8.*t23.*t26.*t31.*t37.*2.0+Ixx1.*Ixx3.*Iyy2.*qp1.*qp2.*t5.*t35.*4.0+Ixx2.*Ixx3.*Iyy3.*qp1.*qp2.*t5.*t35.*4.0+Ixx2.*Ixx3.*Iyy2.*qp1.*qp2.*t34.*t35.*4.0-Ixx2.*Ixx3.*Iyy3.*qp1.*qp2.*t34.*t35.*2.0+Ixx1.*Ixx3.*Izz3.*qp1.*qp2.*t5.*t35.*8.0-Ixx1.*Ixx3.*Izz3.*qp1.*qp2.*t5.*t38.*8.0+Ixx2.*Ixx3.*Izz3.*qp1.*qp2.*t34.*t35.*8.0-Ixx3.*Iyy2.*Iyy3.*qp1.*qp2.*t34.*t35.*2.0-Ixx2.*Ixx3.*Izz3.*qp1.*qp2.*t34.*t38.*8.0;
et79 = Ixx1.*Iyy2.*Izz3.*qp1.*qp2.*t5.*t35.*-4.0+Ixx3.*Iyy2.*Izz2.*qp1.*qp2.*t5.*t35.*4.0-Ixx2.*Iyy3.*Izz3.*qp1.*qp2.*t5.*t35.*4.0-Ixx2.*Iyy2.*Izz3.*qp1.*qp2.*t34.*t35.*4.0-Ixx3.*Iyy2.*Izz2.*qp1.*qp2.*t34.*t35.*4.0+Ixx2.*Iyy3.*Izz3.*qp1.*qp2.*t34.*t35.*2.0-Ixx3.*Iyy2.*Izz3.*qp1.*qp2.*t34.*t35.*8.0+Ixx3.*Iyy2.*Izz3.*qp1.*qp2.*t34.*t38.*8.0+Ixx3.*Izz2.*Izz3.*qp1.*qp2.*t5.*t35.*8.0-Ixx3.*Izz2.*Izz3.*qp1.*qp2.*t5.*t38.*8.0-Ixx3.*Izz2.*Izz3.*qp1.*qp2.*t34.*t35.*8.0+Iyy2.*Iyy3.*Izz3.*qp1.*qp2.*t34.*t35.*2.0+Ixx3.*Izz2.*Izz3.*qp1.*qp2.*t34.*t38.*8.0-Iyy2.*Izz2.*Izz3.*qp1.*qp2.*t5.*t35.*4.0+Iyy2.*Izz2.*Izz3.*qp1.*qp2.*t34.*t35.*4.0+Ixx1.*Ixx3.*Iyy2.*t6.*t8.*t30.*t33.*2.0-Ixx2.*Ixx3.*Iyy2.*t6.*t8.*t31.*t33.*2.0+Ixx2.*Ixx3.*Iyy3.*t6.*t8.*t30.*t33.*2.0+Ixx2.*Ixx3.*Iyy2.*t6.*t8.*t30.*t36.*2.0-Ixx2.*Ixx3.*Iyy3.*t6.*t8.*t30.*t36.*2.0;
et80 = Ixx1.*Ixx3.*Izz3.*t6.*t8.*t30.*t33.*2.0-Ixx2.*Ixx3.*Izz3.*t6.*t8.*t31.*t33.*2.0+Ixx2.*Ixx3.*Izz3.*t6.*t8.*t30.*t36.*2.0-Ixx3.*Iyy2.*Iyy3.*t6.*t8.*t30.*t36.*2.0-Ixx1.*Ixx3.*Izz3.*t8.*t30.*t33.*t37.*4.0+Ixx2.*Ixx3.*Izz3.*t8.*t31.*t33.*t37.*4.0-Ixx2.*Ixx3.*Izz3.*t8.*t30.*t36.*t37.*4.0-Ixx1.*Iyy2.*Izz3.*t6.*t8.*t30.*t33.*2.0+Ixx3.*Iyy2.*Izz2.*t6.*t8.*t30.*t33.*2.0+Ixx2.*Iyy2.*Izz3.*t6.*t8.*t31.*t33.*2.0+Ixx3.*Iyy2.*Izz2.*t6.*t8.*t31.*t33.*2.0-Ixx3.*Iyy3.*Izz2.*t6.*t8.*t30.*t33.*2.0+Ixx3.*Iyy2.*Izz3.*t6.*t8.*t31.*t33.*2.0-Ixx2.*Iyy2.*Izz3.*t6.*t8.*t30.*t36.*2.0-Ixx3.*Iyy2.*Izz2.*t6.*t8.*t30.*t36.*2.0+Ixx2.*Iyy3.*Izz3.*t6.*t8.*t30.*t36.*2.0-Ixx3.*Iyy2.*Izz3.*t6.*t8.*t30.*t36.*2.0+Ixx3.*Iyy3.*Izz2.*t6.*t8.*t30.*t36.*2.0-Ixx3.*Iyy2.*Izz3.*t8.*t31.*t33.*t37.*4.0+Ixx3.*Iyy2.*Izz3.*t8.*t30.*t36.*t37.*4.0+Ixx3.*Izz2.*Izz3.*t6.*t8.*t30.*t33.*2.0;
et81 = Iyy2.*Iyy3.*Izz3.*t6.*t8.*t30.*t33.*-2.0+Ixx3.*Izz2.*Izz3.*t6.*t8.*t31.*t33.*2.0-Ixx3.*Izz2.*Izz3.*t6.*t8.*t30.*t36.*2.0+Iyy2.*Iyy3.*Izz3.*t6.*t8.*t30.*t36.*2.0-Ixx3.*Izz2.*Izz3.*t8.*t30.*t33.*t37.*4.0-Ixx3.*Izz2.*Izz3.*t8.*t31.*t33.*t37.*4.0+Ixx3.*Izz2.*Izz3.*t8.*t30.*t36.*t37.*4.0-Iyy2.*Izz2.*Izz3.*t6.*t8.*t30.*t33.*2.0-Iyy2.*Izz2.*Izz3.*t6.*t8.*t31.*t33.*2.0+Iyy2.*Izz2.*Izz3.*t6.*t8.*t30.*t36.*2.0+Ixx1.*Iyy2.*g.*lcm3.*m3.*t5.*t8.*2.0+Ixx2.*Iyy2.*g.*lcm3.*m3.*t8.*t34.*2.0+Ixx3.*Iyy2.*g.*lcm3.*m3.*t8.*t34.*2.0+Ixx1.*Izz3.*g.*lcm3.*m3.*t5.*t8.*2.0+Iyy2.*Iyy3.*g.*lcm3.*m3.*t5.*t8.*2.0+Ixx2.*Izz3.*g.*lcm3.*m3.*t8.*t34.*2.0-Iyy2.*Iyy3.*g.*lcm3.*m3.*t8.*t34.*2.0+Ixx3.*Izz3.*g.*lcm3.*m3.*t8.*t34.*2.0+Iyy2.*Izz2.*g.*lcm3.*m3.*t5.*t8.*2.0+Iyy3.*Izz3.*g.*lcm3.*m3.*t5.*t8.*2.0-Iyy2.*Izz2.*g.*lcm3.*m3.*t8.*t34.*2.0;
et82 = Iyy3.*Izz3.*g.*lcm3.*m3.*t8.*t34.*-2.0+Izz2.*Izz3.*g.*lcm3.*m3.*t5.*t8.*2.0-Izz2.*Izz3.*g.*lcm3.*m3.*t8.*t34.*2.0-Ixx1.*Ixx3.*l2.*lcm3.*m3.*t8.*t30.*2.0-Ixx1.*Ixx3.*l2.*lcm3.*m3.*t8.*t31.*6.0+Ixx1.*Ixx3.*l2.*lcm3.*m3.*t30.*t49.*2.0+Ixx1.*Ixx3.*l2.*lcm3.*m3.*t31.*t49.*6.0-Ixx1.*Iyy2.*l2.*lcm3.*m3.*t8.*t30.*2.0-Ixx1.*Iyy2.*l2.*lcm3.*m3.*t8.*t31.*2.0-Ixx3.*Iyy2.*l2.*lcm3.*m3.*t8.*t31.*2.0-Ixx3.*Iyy3.*l2.*lcm3.*m3.*t8.*t30.*2.0-Ixx3.*Iyy3.*l2.*lcm3.*m3.*t8.*t32.*2.0+Ixx3.*Iyy2.*l2.*lcm3.*m3.*t31.*t49.*2.0+Ixx3.*Iyy3.*l2.*lcm3.*m3.*t30.*t49.*2.0+Ixx3.*Iyy3.*l2.*lcm3.*m3.*t32.*t49.*2.0+Ixx1.*Izz3.*l2.*lcm3.*m3.*t8.*t31.*4.0-Ixx3.*Izz2.*l2.*lcm3.*m3.*t8.*t30.*2.0-Iyy2.*Iyy3.*l2.*lcm3.*m3.*t8.*t30.*2.0-Ixx3.*Izz2.*l2.*lcm3.*m3.*t8.*t31.*6.0-Ixx3.*Izz3.*l2.*lcm3.*m3.*t8.*t31.*2.0;
et83 = Iyy2.*Iyy3.*l2.*lcm3.*m3.*t8.*t32.*-2.0-Ixx1.*Izz3.*l2.*lcm3.*m3.*t30.*t49.*2.0-Ixx1.*Izz3.*l2.*lcm3.*m3.*t31.*t49.*6.0+Ixx3.*Izz2.*l2.*lcm3.*m3.*t30.*t49.*2.0+Ixx3.*Izz2.*l2.*lcm3.*m3.*t31.*t49.*6.0+Ixx3.*Izz3.*l2.*lcm3.*m3.*t31.*t49.*2.0-Iyy2.*Izz2.*l2.*lcm3.*m3.*t8.*t30.*2.0-Iyy2.*Izz2.*l2.*lcm3.*m3.*t8.*t31.*2.0+Iyy2.*Izz3.*l2.*lcm3.*m3.*t8.*t31.*2.0-Iyy2.*Izz3.*l2.*lcm3.*m3.*t31.*t49.*2.0-Iyy3.*Izz3.*l2.*lcm3.*m3.*t30.*t49.*2.0-Iyy3.*Izz3.*l2.*lcm3.*m3.*t32.*t49.*2.0+Izz2.*Izz3.*l2.*lcm3.*m3.*t8.*t31.*4.0-Izz2.*Izz3.*l2.*lcm3.*m3.*t30.*t49.*2.0-Izz2.*Izz3.*l2.*lcm3.*m3.*t31.*t49.*6.0-Ixx1.*Ixx3.*m3.*qp1.*qp2.*t5.*t14.*2.0-Ixx1.*Ixx3.*m2.*qp1.*qp2.*t5.*t18.*2.0-Ixx2.*Ixx3.*m3.*qp1.*qp2.*t14.*t34.*2.0-Ixx2.*Ixx3.*m2.*qp1.*qp2.*t18.*t34.*2.0+Ixx2.*Iyy3.*m3.*qp1.*qp2.*t5.*t14.*4.0;
et84 = Ixx3.*Iyy2.*m3.*qp1.*qp2.*t5.*t14.*-2.0+Ixx3.*Iyy3.*m3.*qp1.*qp2.*t5.*t14.*2.0+Ixx2.*Iyy3.*m2.*qp1.*qp2.*t5.*t18.*4.0-Ixx3.*Iyy2.*m2.*qp1.*qp2.*t5.*t18.*2.0+Ixx3.*Iyy3.*m2.*qp1.*qp2.*t5.*t18.*2.0+Ixx2.*Iyy2.*m3.*qp1.*qp2.*t5.*t20.*4.0+Ixx3.*Iyy2.*m3.*qp1.*qp2.*t5.*t20.*2.0-Ixx2.*Iyy3.*m3.*qp1.*qp2.*t14.*t34.*2.0+Ixx3.*Iyy2.*m3.*qp1.*qp2.*t14.*t34.*2.0-Ixx2.*Iyy3.*m2.*qp1.*qp2.*t18.*t34.*2.0+Ixx3.*Iyy2.*m2.*qp1.*qp2.*t18.*t34.*2.0-Ixx2.*Iyy2.*m3.*qp1.*qp2.*t20.*t34.*4.0-Ixx3.*Iyy2.*m3.*qp1.*qp2.*t20.*t34.*4.0+Ixx3.*Iyy3.*m3.*qp2.*qp3.*t14.*t44+Ixx3.*Iyy3.*m2.*qp2.*qp3.*t18.*t44+Ixx3.*Iyy2.*m3.*qp2.*qp3.*t20.*t44+Ixx1.*Izz3.*m3.*qp1.*qp2.*t5.*t14.*2.0-Ixx3.*Izz2.*m3.*qp1.*qp2.*t5.*t14.*2.0-Ixx3.*Izz3.*m3.*qp1.*qp2.*t5.*t14.*2.0+Ixx1.*Izz3.*m2.*qp1.*qp2.*t5.*t18.*2.0-Ixx3.*Izz2.*m2.*qp1.*qp2.*t5.*t18.*2.0;
et85 = Ixx3.*Izz3.*m2.*qp1.*qp2.*t5.*t18.*-2.0+Ixx2.*Izz3.*m3.*qp1.*qp2.*t5.*t20.*4.0-Iyy2.*Iyy3.*m3.*qp1.*qp2.*t5.*t20.*2.0+Ixx3.*Izz3.*m3.*qp1.*qp2.*t5.*t20.*2.0+Ixx2.*Izz3.*m3.*qp1.*qp2.*t14.*t34.*2.0+Ixx3.*Izz2.*m3.*qp1.*qp2.*t14.*t34.*2.0+Ixx3.*Izz3.*m3.*qp1.*qp2.*t14.*t34.*4.0+Ixx2.*Izz3.*m2.*qp1.*qp2.*t18.*t34.*2.0+Ixx3.*Izz2.*m2.*qp1.*qp2.*t18.*t34.*2.0+Ixx3.*Izz3.*m2.*qp1.*qp2.*t18.*t34.*4.0-Ixx2.*Izz3.*m3.*qp1.*qp2.*t20.*t34.*4.0+Iyy2.*Iyy3.*m3.*qp1.*qp2.*t20.*t34.*4.0-Ixx3.*Izz3.*m3.*qp1.*qp2.*t20.*t34.*4.0+Iyy2.*Iyy3.*m3.*qp2.*qp3.*t20.*t44.*3.0+Ixx3.*Izz3.*m3.*qp2.*qp3.*t20.*t44+Iyy2.*Izz3.*m3.*qp1.*qp2.*t5.*t14.*2.0+Iyy2.*Izz3.*m2.*qp1.*qp2.*t5.*t18.*2.0+Iyy2.*Izz3.*m3.*qp1.*qp2.*t5.*t20.*2.0-Iyy3.*Izz3.*m3.*qp1.*qp2.*t5.*t20.*2.0-Iyy2.*Izz3.*m3.*qp1.*qp2.*t14.*t34.*2.0-Iyy2.*Izz3.*m2.*qp1.*qp2.*t18.*t34.*2.0;
et86 = Iyy3.*Izz3.*m3.*qp1.*qp2.*t20.*t34.*4.0-Iyy2.*Izz3.*m3.*qp2.*qp3.*t20.*t44+Iyy3.*Izz3.*m3.*qp2.*qp3.*t20.*t44.*3.0+Izz2.*Izz3.*m3.*qp1.*qp2.*t5.*t14.*2.0+Izz2.*Izz3.*m2.*qp1.*qp2.*t5.*t18.*2.0-Izz2.*Izz3.*m3.*qp1.*qp2.*t14.*t34.*2.0-Izz2.*Izz3.*m2.*qp1.*qp2.*t18.*t34.*2.0-Ixx1.*Ixx3.*m3.*t8.*t20.*t31.*t37.*4.0+Ixx3.*Izz3.*m3.*t8.*t14.*t31.*t37.*4.0+Ixx3.*Izz3.*m2.*t8.*t18.*t31.*t37.*4.0-Ixx3.*Izz2.*m3.*t8.*t20.*t31.*t37.*4.0-Ixx3.*Iyy3.*t2.*t5.*t6.*t7.*t8.*2.0+Iyy3.*Izz3.*t2.*t5.*t6.*t7.*t8.*2.0+Ixx2.*l2.*lcm3.*m3.*t3.*t6.*t33.*4.0+Ixx3.*l2.*lcm3.*m3.*t1.*t7.*t37.*2.0-Ixx3.*l2.*lcm3.*m3.*t3.*t33.*t37.*4.0+Iyy2.*l2.*lcm3.*m3.*t1.*t6.*t7.*2.0+Iyy3.*l2.*lcm3.*m3.*t1.*t6.*t7.*4.0-Iyy2.*l2.*lcm3.*m3.*t3.*t6.*t33.*4.0-Iyy3.*l2.*lcm3.*m3.*t3.*t6.*t33.*4.0+Izz3.*l2.*lcm3.*m3.*t1.*t6.*t7.*2.0;
et87 = Izz2.*l2.*lcm3.*m3.*t3.*t6.*t33.*-4.0-Izz3.*l2.*lcm3.*m3.*t1.*t7.*t37.*2.0+Izz3.*l2.*lcm3.*m3.*t3.*t33.*t37.*4.0+Ixx1.*g.*lcm3.*t5.*t8.*t14.*t26.*2.0+Ixx2.*g.*lcm3.*t8.*t14.*t26.*t34.*2.0+Ixx3.*g.*lcm3.*t8.*t14.*t26.*t34.*2.0+Iyy2.*g.*lcm3.*t5.*t8.*t14.*t26.*2.0-Iyy2.*g.*lcm3.*t8.*t14.*t26.*t34.*2.0+Izz2.*g.*lcm3.*t5.*t8.*t14.*t26.*2.0+Izz3.*g.*lcm3.*t5.*t8.*t14.*t26.*2.0-Izz2.*g.*lcm3.*t8.*t14.*t26.*t34.*2.0-Izz3.*g.*lcm3.*t8.*t14.*t26.*t34.*2.0-Ixx3.*m2.*m3.*t14.*t18.*t31.*t45.*2.0+Izz3.*m2.*m3.*t14.*t18.*t31.*t45.*2.0+Ixx1.*g.*t5.*t8.*t22.*t26.*t35.*2.0+Ixx2.*g.*t8.*t22.*t26.*t34.*t35.*2.0-Iyy2.*g.*t8.*t22.*t26.*t34.*t35.*2.0+Izz2.*g.*t5.*t8.*t22.*t26.*t35.*2.0-Izz2.*g.*t8.*t22.*t26.*t34.*t35.*2.0+Ixx2.*l2.*t8.*t22.*t26.*t30.*t33.*2.0+Ixx3.*l2.*t8.*t22.*t26.*t30.*t33.*2.0;
et88 = Ixx2.*l2.*t8.*t22.*t26.*t30.*t36.*-2.0-Ixx3.*l2.*t8.*t22.*t26.*t30.*t36.*2.0-Ixx3.*l2.*t8.*t22.*t26.*t31.*t38.*4.0+Iyy2.*l2.*t8.*t22.*t26.*t30.*t33.*2.0-Iyy2.*l2.*t8.*t22.*t26.*t31.*t33.*2.0-Iyy3.*l2.*t8.*t22.*t26.*t30.*t33.*2.0+Iyy2.*l2.*t8.*t22.*t26.*t32.*t33.*2.0+Iyy3.*l2.*t8.*t22.*t26.*t30.*t36.*2.0-Izz2.*l2.*t8.*t22.*t26.*t30.*t33.*2.0+Izz3.*l2.*t8.*t22.*t26.*t30.*t33.*2.0-Izz3.*l2.*t8.*t22.*t26.*t31.*t33.*2.0+Izz2.*l2.*t8.*t22.*t26.*t30.*t36.*2.0+Izz3.*l2.*t8.*t22.*t26.*t32.*t33.*2.0+Izz3.*l2.*t8.*t22.*t26.*t31.*t38.*4.0+Ixx1.*lcm3.*t8.*t15.*t26.*t30.*t33.*2.0-Ixx2.*lcm3.*t8.*t15.*t26.*t30.*t33.*2.0-Ixx2.*lcm3.*t8.*t15.*t26.*t31.*t33.*2.0-Ixx3.*lcm3.*t8.*t15.*t26.*t30.*t33.*2.0-Ixx3.*lcm3.*t8.*t15.*t26.*t31.*t33.*2.0+Ixx2.*lcm3.*t8.*t15.*t26.*t30.*t36.*2.0+Ixx3.*lcm3.*t8.*t15.*t26.*t30.*t36.*2.0;
et89 = Iyy2.*lcm3.*t8.*t15.*t26.*t30.*t33.*4.0+Iyy2.*lcm3.*t8.*t15.*t26.*t31.*t33.*2.0+Iyy3.*lcm3.*t8.*t15.*t26.*t30.*t33.*2.0-Iyy2.*lcm3.*t8.*t15.*t26.*t30.*t36.*2.0+Iyy3.*lcm3.*t8.*t15.*t26.*t32.*t33.*2.0+Izz2.*lcm3.*t8.*t15.*t26.*t30.*t33.*4.0+Izz2.*lcm3.*t8.*t15.*t26.*t31.*t33.*2.0+Izz3.*lcm3.*t8.*t15.*t26.*t30.*t33.*4.0+Izz3.*lcm3.*t8.*t15.*t26.*t31.*t33.*2.0-Izz2.*lcm3.*t8.*t15.*t26.*t30.*t36.*2.0-Izz3.*lcm3.*t8.*t15.*t26.*t30.*t36.*2.0+Ixx3.*qp2.*qp3.*t5.*t7.*t11.*t35.*2.0+Ixx2.*qp1.*qp2.*t5.*t14.*t20.*t26.*4.0+Ixx3.*qp1.*qp2.*t5.*t14.*t20.*t26.*2.0+Ixx3.*qp1.*qp2.*t5.*t16.*t26.*t35.*4.0+Ixx3.*qp1.*qp2.*t5.*t21.*t25.*t35.*4.0+Ixx2.*qp1.*qp2.*t5.*t23.*t26.*t35.*4.0+Ixx3.*qp1.*qp2.*t5.*t23.*t26.*t35.*2.0+Ixx1.*qp1.*qp2.*t5.*t23.*t26.*t38.*4.0-Ixx2.*qp1.*qp2.*t14.*t20.*t26.*t34.*4.0-Ixx3.*qp1.*qp2.*t14.*t20.*t26.*t34.*2.0;
et90 = Ixx3.*qp2.*qp3.*t14.*t20.*t26.*t44-Ixx3.*qp1.*qp2.*t16.*t26.*t34.*t35.*4.0-Ixx3.*qp1.*qp2.*t21.*t25.*t34.*t35.*4.0-Ixx2.*qp1.*qp2.*t23.*t26.*t34.*t35.*4.0-Ixx3.*qp1.*qp2.*t23.*t26.*t34.*t35.*2.0+Ixx2.*qp1.*qp2.*t23.*t26.*t34.*t38.*4.0-Iyy3.*qp2.*qp3.*t5.*t7.*t10.*t35.*2.0+Iyy3.*qp2.*qp3.*t5.*t7.*t13.*t35.*2.0-Iyy3.*qp1.*qp2.*t5.*t14.*t20.*t26.*2.0-Iyy3.*qp1.*qp2.*t5.*t23.*t26.*t35.*2.0+Iyy3.*qp1.*qp2.*t14.*t20.*t26.*t34.*2.0+Iyy3.*qp2.*qp3.*t14.*t20.*t26.*t44+Iyy2.*qp1.*qp2.*t23.*t26.*t34.*t35.*4.0+Iyy3.*qp1.*qp2.*t23.*t26.*t34.*t35.*2.0-Iyy2.*qp1.*qp2.*t23.*t26.*t34.*t38.*4.0-Izz3.*qp2.*qp3.*t5.*t7.*t11.*t35.*2.0-Izz3.*qp1.*qp2.*t5.*t16.*t26.*t35.*4.0-Izz3.*qp1.*qp2.*t5.*t21.*t25.*t35.*4.0+Izz3.*qp1.*qp2.*t5.*t23.*t26.*t35.*2.0+Izz2.*qp1.*qp2.*t5.*t23.*t26.*t38.*4.0+Izz3.*qp1.*qp2.*t16.*t26.*t34.*t35.*4.0;
et91 = Izz3.*qp1.*qp2.*t21.*t25.*t34.*t35.*4.0+Izz3.*qp1.*qp2.*t23.*t26.*t34.*t35.*2.0-Izz2.*qp1.*qp2.*t23.*t26.*t34.*t38.*4.0+Ixx3.*t6.*t8.*t16.*t26.*t30.*t33.*2.0+Ixx3.*t6.*t8.*t16.*t26.*t31.*t33.*2.0-Ixx3.*t6.*t8.*t16.*t26.*t30.*t36.*2.0+Ixx3.*t6.*t8.*t21.*t25.*t30.*t33.*2.0+Ixx3.*t6.*t8.*t21.*t25.*t31.*t33.*2.0+Ixx2.*t6.*t8.*t23.*t26.*t30.*t33.*2.0-Ixx3.*t6.*t8.*t21.*t25.*t30.*t36.*2.0+Ixx3.*t6.*t8.*t23.*t26.*t30.*t33.*2.0-Ixx2.*t6.*t8.*t23.*t26.*t30.*t36.*2.0-Ixx3.*t6.*t8.*t23.*t26.*t30.*t36.*2.0-Ixx3.*t8.*t14.*t20.*t26.*t30.*t37.*4.0-Ixx3.*t8.*t14.*t20.*t26.*t31.*t37.*1.0e+1-Ixx3.*t8.*t14.*t20.*t26.*t32.*t37.*2.0+Ixx1.*t8.*t23.*t26.*t30.*t33.*t37.*2.0-Ixx2.*t8.*t23.*t26.*t31.*t33.*t37.*2.0+Ixx2.*t8.*t23.*t26.*t30.*t36.*t37.*2.0-Iyy3.*t6.*t8.*t23.*t26.*t30.*t33.*2.0+Iyy3.*t6.*t8.*t23.*t26.*t30.*t36.*2.0;
et92 = Iyy2.*t8.*t23.*t26.*t30.*t36.*t37.*-2.0-Izz3.*t6.*t8.*t16.*t26.*t30.*t33.*2.0-Izz3.*t6.*t8.*t16.*t26.*t31.*t33.*2.0+Izz3.*t6.*t8.*t16.*t26.*t30.*t36.*2.0-Izz3.*t6.*t8.*t21.*t25.*t30.*t33.*2.0-Izz3.*t6.*t8.*t21.*t25.*t31.*t33.*2.0-Izz2.*t6.*t8.*t23.*t26.*t30.*t33.*2.0+Izz3.*t6.*t8.*t21.*t25.*t30.*t36.*2.0+Izz2.*t6.*t8.*t23.*t26.*t30.*t36.*2.0+Izz2.*t8.*t23.*t26.*t30.*t33.*t37.*2.0+Izz2.*t8.*t23.*t26.*t31.*t33.*t37.*2.0-Izz2.*t8.*t23.*t26.*t30.*t36.*t37.*2.0+l2.*lcm3.*m2.*m3.*t3.*t6.*t18.*8.0+g.*lcm3.*m3.*t5.*t8.*t21.*t25.*2.0-g.*lcm3.*m3.*t8.*t21.*t25.*t34.*2.0-l2.*lcm3.*m3.*t8.*t11.*t30.*t33.*2.0-l2.*lcm3.*m3.*t8.*t21.*t25.*t30.*2.0+l2.*lcm3.*m3.*t8.*t11.*t30.*t36.*2.0-l2.*lcm3.*m3.*t8.*t21.*t25.*t31.*2.0-l2.*lcm3.*m3.*t8.*t10.*t31.*t38.*2.0;
et93 = l2.*lcm3.*m3.*t8.*t13.*t31.*t38.*-2.0+g.*l2.*t5.*t8.*t23.*t27.*t37.*2.0-g.*l2.*t8.*t23.*t27.*t34.*t37.*2.0+g.*m2.*t5.*t8.*t18.*t22.*t26.*2.0-l2.*m2.*t8.*t18.*t22.*t26.*t30.*4.0-l2.*m2.*t8.*t18.*t22.*t26.*t31.*8.0-l2.*m2.*t8.*t18.*t22.*t26.*t32.*2.0+l2.*m2.*t18.*t22.*t26.*t30.*t49.*2.0+l2.*m2.*t18.*t22.*t26.*t31.*t49.*8.0-lcm3.*m2.*t8.*t15.*t18.*t26.*t30.*4.0-lcm3.*m2.*t8.*t15.*t18.*t26.*t31.*4.0-m2.*m3.*t3.*t18.*t20.*t33.*t35.*4.0+l2.*qp1.*qp3.*t7.*t8.*t24.*t27.*4.0-l2.*qp1.*qp2.*t5.*t24.*t27.*t37.*4.0+l2.*qp1.*qp2.*t5.*t24.*t27.*t39.*4.0-l2.*qp1.*qp3.*t7.*t24.*t27.*t49.*4.0+l2.*qp1.*qp2.*t24.*t27.*t34.*t37.*4.0-l2.*qp1.*qp2.*t24.*t27.*t34.*t39.*4.0+g.*t5.*t6.*t8.*t15.*t20.*t27.*6.0-g.*t6.*t8.*t15.*t20.*t27.*t34.*6.0;
et94 = g.*t5.*t8.*t14.*t22.*t27.*t35.*6.0-g.*t8.*t14.*t22.*t27.*t34.*t35.*6.0-m3.*qp1.*qp2.*t5.*t10.*t14.*t35.*2.0-m2.*qp1.*qp2.*t5.*t10.*t18.*t35.*2.0+m3.*qp1.*qp2.*t5.*t10.*t14.*t38.*4.0-m3.*qp1.*qp2.*t5.*t13.*t14.*t35.*6.0+m2.*qp1.*qp2.*t5.*t10.*t18.*t38.*4.0-m2.*qp1.*qp2.*t5.*t13.*t18.*t35.*6.0+m3.*qp1.*qp2.*t5.*t10.*t20.*t35.*2.0+m3.*qp1.*qp2.*t5.*t13.*t14.*t38.*4.0-m3.*qp1.*qp2.*t5.*t11.*t20.*t35.*2.0+m2.*qp1.*qp2.*t5.*t13.*t18.*t38.*4.0-m3.*qp1.*qp2.*t5.*t13.*t20.*t35.*2.0+m3.*qp1.*qp2.*t10.*t14.*t34.*t35.*8.0+m2.*qp1.*qp2.*t10.*t18.*t34.*t35.*8.0-m3.*qp1.*qp2.*t10.*t14.*t34.*t38.*8.0+m3.*qp1.*qp2.*t13.*t14.*t34.*t35.*8.0-m2.*qp1.*qp2.*t10.*t18.*t34.*t38.*8.0+m2.*qp1.*qp2.*t13.*t18.*t34.*t35.*8.0-m3.*qp1.*qp2.*t10.*t20.*t34.*t35.*2.0;
et95 = m3.*qp1.*qp2.*t13.*t14.*t34.*t38.*-8.0+m3.*qp1.*qp2.*t11.*t20.*t34.*t35.*2.0-m2.*qp1.*qp2.*t13.*t18.*t34.*t38.*8.0-m3.*qp1.*qp2.*t13.*t20.*t34.*t35.*2.0+m2.*qp2.*qp3.*t18.*t23.*t26.*t44.*2.0-l2.*t2.*t5.*t7.*t8.*t22.*t26.*2.0+l2.*t8.*t24.*t27.*t30.*t33.*t35.*2.0+l2.*t8.*t24.*t27.*t32.*t33.*t35.*2.0+l2.*t8.*t24.*t27.*t30.*t33.*t38.*2.0+l2.*t8.*t24.*t27.*t31.*t33.*t38.*2.0-l2.*t8.*t24.*t27.*t30.*t36.*t38.*2.0-m3.*t6.*t8.*t10.*t14.*t31.*t33.*2.0+m3.*t6.*t8.*t10.*t14.*t30.*t36.*2.0-m3.*t6.*t8.*t13.*t14.*t30.*t33.*2.0-m2.*t6.*t8.*t10.*t18.*t31.*t33.*2.0-m3.*t6.*t8.*t13.*t14.*t31.*t33.*2.0+m2.*t6.*t8.*t10.*t18.*t30.*t36.*2.0-m2.*t6.*t8.*t13.*t18.*t30.*t33.*2.0+m3.*t6.*t8.*t10.*t20.*t30.*t33.*2.0+m3.*t6.*t8.*t13.*t14.*t30.*t36.*2.0;
et96 = m2.*t6.*t8.*t13.*t18.*t31.*t33.*-2.0-m3.*t6.*t8.*t11.*t20.*t30.*t33.*2.0+m2.*t6.*t8.*t13.*t18.*t30.*t36.*2.0-m3.*t6.*t8.*t10.*t20.*t30.*t36.*2.0-m3.*t6.*t8.*t13.*t20.*t30.*t33.*2.0+m3.*t6.*t8.*t11.*t20.*t30.*t36.*2.0+m3.*t6.*t8.*t13.*t20.*t31.*t33.*2.0+m3.*t8.*t10.*t14.*t30.*t33.*t37.*2.0+m3.*t8.*t10.*t14.*t31.*t33.*t37.*4.0+m2.*t8.*t10.*t18.*t30.*t33.*t37.*2.0-m3.*t8.*t10.*t14.*t30.*t36.*t37.*4.0+m3.*t8.*t13.*t14.*t30.*t33.*t37.*2.0+m2.*t8.*t10.*t18.*t31.*t33.*t37.*4.0+m3.*t8.*t13.*t14.*t31.*t33.*t37.*4.0-m2.*t8.*t10.*t18.*t30.*t36.*t37.*4.0+m2.*t8.*t13.*t18.*t30.*t33.*t37.*2.0-m3.*t8.*t13.*t14.*t30.*t36.*t37.*4.0+m2.*t8.*t13.*t18.*t31.*t33.*t37.*4.0-m2.*t8.*t13.*t18.*t30.*t36.*t37.*4.0-m2.*t8.*t18.*t23.*t26.*t31.*t37.*2.0-m2.*t14.*t18.*t20.*t26.*t30.*t45.*4.0;
et97 = m2.*t14.*t18.*t20.*t26.*t31.*t45.*-5.0-m2.*t14.*t18.*t20.*t26.*t32.*t45-qp1.*qp2.*t5.*t6.*t15.*t22.*t27.*1.2e+1+qp1.*qp3.*t7.*t8.*t15.*t22.*t27.*8.0+qp1.*qp2.*t6.*t15.*t22.*t27.*t34.*1.2e+1+qp1.*qp2.*t5.*t15.*t22.*t27.*t37.*1.2e+1+qp1.*qp3.*t8.*t15.*t22.*t27.*t47.*4.0-qp1.*qp3.*t7.*t15.*t22.*t27.*t49.*8.0-qp1.*qp2.*t15.*t22.*t27.*t34.*t37.*1.2e+1-t2.*t5.*t6.*t7.*t8.*t23.*t26.*2.0+t6.*t8.*t14.*t23.*t27.*t30.*t33.*4.0+t6.*t8.*t14.*t23.*t27.*t32.*t33.*4.0+t8.*t15.*t22.*t27.*t30.*t33.*t35.*2.2e+1+t8.*t15.*t22.*t27.*t31.*t33.*t35.*1.2e+1+t8.*t14.*t23.*t27.*t30.*t33.*t37.*1.2e+1+t8.*t15.*t22.*t27.*t32.*t33.*t35.*4.0+t8.*t14.*t23.*t27.*t31.*t33.*t37.*8.0-t8.*t15.*t22.*t27.*t30.*t35.*t36.*1.2e+1+t8.*t14.*t23.*t27.*t32.*t33.*t37.*2.0-t8.*t14.*t23.*t27.*t30.*t36.*t37.*8.0;
et98 = Ixx3.*Iyy2.*Iyy3.*qp2.*qp3.*t5.*t7.*t35.*-4.0+Iyy2.*Iyy3.*Izz3.*qp2.*qp3.*t5.*t7.*t35.*4.0-Ixx3.*Iyy3.*g.*l2.*m3.*t5.*t6.*t8.*2.0+Ixx3.*Iyy3.*g.*l2.*m3.*t6.*t8.*t34.*2.0+Iyy3.*Izz3.*g.*l2.*m3.*t5.*t6.*t8.*2.0-Iyy3.*Izz3.*g.*l2.*m3.*t6.*t8.*t34.*2.0+Ixx1.*Ixx3.*g.*lcm3.*m3.*t5.*t8.*t35.*2.0+Ixx2.*Ixx3.*g.*lcm3.*m3.*t8.*t34.*t35.*2.0-Ixx3.*Iyy3.*g.*lcm2.*m2.*t5.*t6.*t8.*2.0+Ixx3.*Iyy3.*g.*lcm2.*m2.*t6.*t8.*t34.*2.0-Ixx3.*Iyy2.*g.*lcm3.*m3.*t8.*t34.*t35.*2.0-Ixx1.*Izz3.*g.*lcm3.*m3.*t5.*t8.*t35.*2.0+Ixx3.*Izz2.*g.*lcm3.*m3.*t5.*t8.*t35.*2.0-Ixx2.*Izz3.*g.*lcm3.*m3.*t8.*t34.*t35.*2.0-Ixx3.*Izz2.*g.*lcm3.*m3.*t8.*t34.*t35.*2.0+Iyy3.*Izz3.*g.*lcm2.*m2.*t5.*t6.*t8.*2.0-Iyy3.*Izz3.*g.*lcm2.*m2.*t6.*t8.*t34.*2.0+Iyy2.*Izz3.*g.*lcm3.*m3.*t8.*t34.*t35.*2.0-Izz2.*Izz3.*g.*lcm3.*m3.*t5.*t8.*t35.*2.0;
et99 = Izz2.*Izz3.*g.*lcm3.*m3.*t8.*t34.*t35.*2.0+Ixx1.*Iyy2.*l2.*lcm3.*m3.*t8.*t30.*t33.*2.0-Ixx2.*Iyy2.*l2.*lcm3.*m3.*t8.*t30.*t33.*2.0-Ixx2.*Iyy2.*l2.*lcm3.*m3.*t8.*t31.*t33.*2.0+Ixx2.*Iyy3.*l2.*lcm3.*m3.*t8.*t30.*t33.*2.0-Ixx3.*Iyy2.*l2.*lcm3.*m3.*t8.*t30.*t33.*2.0-Ixx3.*Iyy2.*l2.*lcm3.*m3.*t8.*t31.*t33.*2.0+Ixx3.*Iyy3.*l2.*lcm3.*m3.*t8.*t30.*t33.*2.0+Ixx2.*Iyy2.*l2.*lcm3.*m3.*t8.*t30.*t36.*2.0-Ixx2.*Iyy3.*l2.*lcm3.*m3.*t8.*t30.*t36.*2.0+Ixx3.*Iyy2.*l2.*lcm3.*m3.*t8.*t30.*t36.*2.0-Ixx3.*Iyy3.*l2.*lcm3.*m3.*t8.*t30.*t36.*2.0+Ixx1.*Izz3.*l2.*lcm3.*m3.*t8.*t30.*t33.*2.0-Ixx2.*Izz3.*l2.*lcm3.*m3.*t8.*t30.*t33.*2.0+Iyy2.*Iyy3.*l2.*lcm3.*m3.*t8.*t30.*t33.*4.0-Ixx2.*Izz3.*l2.*lcm3.*m3.*t8.*t31.*t33.*2.0-Ixx3.*Izz3.*l2.*lcm3.*m3.*t8.*t30.*t33.*2.0-Ixx3.*Izz3.*l2.*lcm3.*m3.*t8.*t31.*t33.*2.0+Iyy2.*Iyy3.*l2.*lcm3.*m3.*t8.*t32.*t33.*2.0;
et100 = Ixx2.*Izz3.*l2.*lcm3.*m3.*t8.*t30.*t36.*2.0-Iyy2.*Iyy3.*l2.*lcm3.*m3.*t8.*t30.*t36.*2.0+Ixx3.*Izz3.*l2.*lcm3.*m3.*t8.*t30.*t36.*2.0+Ixx3.*Izz3.*l2.*lcm3.*m3.*t8.*t31.*t38.*4.0+Iyy2.*Izz2.*l2.*lcm3.*m3.*t8.*t30.*t33.*4.0+Iyy2.*Izz2.*l2.*lcm3.*m3.*t8.*t31.*t33.*2.0-Iyy3.*Izz2.*l2.*lcm3.*m3.*t8.*t30.*t33.*2.0+Iyy3.*Izz3.*l2.*lcm3.*m3.*t8.*t30.*t33.*4.0-Iyy2.*Izz2.*l2.*lcm3.*m3.*t8.*t30.*t36.*2.0+Iyy3.*Izz2.*l2.*lcm3.*m3.*t8.*t30.*t36.*2.0+Iyy3.*Izz3.*l2.*lcm3.*m3.*t8.*t32.*t33.*2.0-Iyy3.*Izz3.*l2.*lcm3.*m3.*t8.*t30.*t36.*2.0+Izz2.*Izz3.*l2.*lcm3.*m3.*t8.*t30.*t33.*4.0+Izz2.*Izz3.*l2.*lcm3.*m3.*t8.*t31.*t33.*2.0-Izz2.*Izz3.*l2.*lcm3.*m3.*t8.*t30.*t36.*2.0+Ixx1.*Ixx3.*m3.*qp1.*qp2.*t5.*t14.*t35.*4.0+Ixx1.*Ixx3.*m2.*qp1.*qp2.*t5.*t18.*t35.*4.0+Ixx2.*Ixx3.*m3.*qp1.*qp2.*t5.*t20.*t35.*4.0+Ixx1.*Ixx3.*m3.*qp1.*qp2.*t5.*t20.*t38.*8.0;
et101 = Ixx2.*Ixx3.*m3.*qp1.*qp2.*t14.*t34.*t35.*4.0+Ixx2.*Ixx3.*m2.*qp1.*qp2.*t18.*t34.*t35.*4.0-Ixx2.*Ixx3.*m3.*qp1.*qp2.*t20.*t34.*t35.*6.0+Ixx2.*Ixx3.*m3.*qp1.*qp2.*t20.*t34.*t38.*8.0+Ixx3.*Iyy2.*m3.*qp1.*qp2.*t5.*t14.*t35.*4.0+Ixx3.*Iyy2.*m2.*qp1.*qp2.*t5.*t18.*t35.*4.0+Ixx2.*Iyy3.*m3.*qp1.*qp2.*t5.*t20.*t35.*4.0-Ixx3.*Iyy2.*m3.*qp1.*qp2.*t14.*t34.*t35.*4.0-Ixx3.*Iyy2.*m2.*qp1.*qp2.*t18.*t34.*t35.*4.0+Ixx2.*Iyy2.*m3.*qp1.*qp2.*t20.*t34.*t35.*4.0-Ixx2.*Iyy3.*m3.*qp1.*qp2.*t20.*t34.*t35.*2.0+Ixx3.*Iyy2.*m3.*qp1.*qp2.*t20.*t34.*t35.*1.0e+1-Ixx3.*Iyy2.*m3.*qp1.*qp2.*t20.*t34.*t38.*8.0-Ixx1.*Izz3.*m3.*qp1.*qp2.*t5.*t14.*t35.*4.0+Ixx3.*Izz2.*m3.*qp1.*qp2.*t5.*t14.*t35.*4.0+Ixx3.*Izz3.*m3.*qp1.*qp2.*t5.*t14.*t35.*8.0-Ixx1.*Izz3.*m2.*qp1.*qp2.*t5.*t18.*t35.*4.0+Ixx3.*Izz2.*m2.*qp1.*qp2.*t5.*t18.*t35.*4.0;
et102 = Ixx3.*Izz3.*m2.*qp1.*qp2.*t5.*t18.*t35.*8.0-Ixx3.*Izz3.*m3.*qp1.*qp2.*t5.*t14.*t38.*8.0-Ixx2.*Izz3.*m3.*qp1.*qp2.*t5.*t20.*t35.*4.0-Ixx3.*Izz3.*m2.*qp1.*qp2.*t5.*t18.*t38.*8.0+Ixx3.*Izz2.*m3.*qp1.*qp2.*t5.*t20.*t38.*8.0-Ixx2.*Izz3.*m3.*qp1.*qp2.*t14.*t34.*t35.*4.0-Ixx3.*Izz2.*m3.*qp1.*qp2.*t14.*t34.*t35.*4.0-Ixx3.*Izz3.*m3.*qp1.*qp2.*t14.*t34.*t35.*1.6e+1-Ixx2.*Izz3.*m2.*qp1.*qp2.*t18.*t34.*t35.*4.0-Ixx3.*Izz2.*m2.*qp1.*qp2.*t18.*t34.*t35.*4.0-Ixx3.*Izz3.*m2.*qp1.*qp2.*t18.*t34.*t35.*1.6e+1+Ixx3.*Izz3.*m3.*qp1.*qp2.*t14.*t34.*t38.*1.6e+1+Ixx2.*Izz3.*m3.*qp1.*qp2.*t20.*t34.*t35.*1.0e+1-Iyy2.*Iyy3.*m3.*qp1.*qp2.*t20.*t34.*t35.*2.0+Ixx3.*Izz3.*m2.*qp1.*qp2.*t18.*t34.*t38.*1.6e+1+Ixx3.*Izz3.*m3.*qp1.*qp2.*t20.*t34.*t35.*8.0-Ixx2.*Izz3.*m3.*qp1.*qp2.*t20.*t34.*t38.*8.0;
et103 = Ixx3.*Izz2.*m3.*qp1.*qp2.*t20.*t34.*t38.*-8.0-Iyy2.*Izz3.*m3.*qp1.*qp2.*t5.*t14.*t35.*4.0-Iyy2.*Izz3.*m2.*qp1.*qp2.*t5.*t18.*t35.*4.0+Iyy3.*Izz3.*m3.*qp1.*qp2.*t5.*t20.*t35.*4.0+Iyy2.*Izz3.*m3.*qp1.*qp2.*t14.*t34.*t35.*4.0+Iyy2.*Izz3.*m2.*qp1.*qp2.*t18.*t34.*t35.*4.0-Iyy2.*Izz3.*m3.*qp1.*qp2.*t20.*t34.*t35.*6.0-Iyy3.*Izz3.*m3.*qp1.*qp2.*t20.*t34.*t35.*4.0+Iyy2.*Izz3.*m3.*qp1.*qp2.*t20.*t34.*t38.*8.0-Izz2.*Izz3.*m3.*qp1.*qp2.*t5.*t14.*t35.*4.0-Izz2.*Izz3.*m2.*qp1.*qp2.*t5.*t18.*t35.*4.0+Izz2.*Izz3.*m3.*qp1.*qp2.*t14.*t34.*t35.*4.0+Izz2.*Izz3.*m2.*qp1.*qp2.*t18.*t34.*t35.*4.0+Ixx1.*Ixx3.*m3.*t6.*t8.*t14.*t30.*t33.*2.0-Ixx2.*Ixx3.*m3.*t6.*t8.*t14.*t31.*t33.*2.0+Ixx1.*Ixx3.*m2.*t6.*t8.*t18.*t30.*t33.*2.0+Ixx2.*Ixx3.*m3.*t6.*t8.*t14.*t30.*t36.*2.0-Ixx2.*Ixx3.*m2.*t6.*t8.*t18.*t31.*t33.*2.0;
et104 = Ixx2.*Ixx3.*m2.*t6.*t8.*t18.*t30.*t36.*2.0+Ixx2.*Ixx3.*m3.*t6.*t8.*t20.*t30.*t33.*2.0-Ixx2.*Ixx3.*m3.*t6.*t8.*t20.*t30.*t36.*2.0+Ixx1.*Ixx3.*m3.*t8.*t20.*t30.*t33.*t37.*4.0-Ixx2.*Ixx3.*m3.*t8.*t20.*t31.*t33.*t37.*4.0+Ixx2.*Ixx3.*m3.*t8.*t20.*t30.*t36.*t37.*4.0+Ixx3.*Iyy2.*m3.*t6.*t8.*t14.*t30.*t33.*2.0+Ixx3.*Iyy2.*m3.*t6.*t8.*t14.*t31.*t33.*2.0+Ixx3.*Iyy2.*m2.*t6.*t8.*t18.*t30.*t33.*2.0-Ixx3.*Iyy2.*m3.*t6.*t8.*t14.*t30.*t36.*2.0+Ixx3.*Iyy2.*m2.*t6.*t8.*t18.*t31.*t33.*2.0+Ixx2.*Iyy3.*m3.*t6.*t8.*t20.*t30.*t33.*2.0-Ixx3.*Iyy2.*m2.*t6.*t8.*t18.*t30.*t36.*2.0+Ixx2.*Iyy2.*m3.*t6.*t8.*t20.*t30.*t36.*2.0-Ixx2.*Iyy3.*m3.*t6.*t8.*t20.*t30.*t36.*2.0+Ixx3.*Iyy2.*m3.*t6.*t8.*t20.*t30.*t36.*2.0-Ixx3.*Iyy2.*m3.*t8.*t20.*t30.*t36.*t37.*4.0-Ixx1.*Izz3.*m3.*t6.*t8.*t14.*t30.*t33.*2.0+Ixx3.*Izz2.*m3.*t6.*t8.*t14.*t30.*t33.*2.0;
et105 = Ixx2.*Izz3.*m3.*t6.*t8.*t14.*t31.*t33.*2.0+Ixx3.*Izz2.*m3.*t6.*t8.*t14.*t31.*t33.*2.0+Ixx3.*Izz3.*m3.*t6.*t8.*t14.*t30.*t33.*2.0-Ixx1.*Izz3.*m2.*t6.*t8.*t18.*t30.*t33.*2.0+Ixx3.*Izz3.*m3.*t6.*t8.*t14.*t31.*t33.*4.0-Ixx2.*Izz3.*m3.*t6.*t8.*t14.*t30.*t36.*2.0+Ixx3.*Izz2.*m2.*t6.*t8.*t18.*t30.*t33.*2.0-Ixx3.*Izz2.*m3.*t6.*t8.*t14.*t30.*t36.*2.0+Ixx2.*Izz3.*m2.*t6.*t8.*t18.*t31.*t33.*2.0+Ixx3.*Izz2.*m2.*t6.*t8.*t18.*t31.*t33.*2.0+Ixx3.*Izz3.*m2.*t6.*t8.*t18.*t30.*t33.*2.0-Ixx3.*Izz3.*m3.*t6.*t8.*t14.*t30.*t36.*4.0+Ixx3.*Izz3.*m2.*t6.*t8.*t18.*t31.*t33.*4.0-Ixx2.*Izz3.*m2.*t6.*t8.*t18.*t30.*t36.*2.0-Ixx3.*Izz2.*m2.*t6.*t8.*t18.*t30.*t36.*2.0-Ixx3.*Izz2.*m3.*t6.*t8.*t20.*t30.*t33.*2.0-Ixx3.*Izz3.*m2.*t6.*t8.*t18.*t30.*t36.*4.0+Ixx2.*Izz3.*m3.*t6.*t8.*t20.*t30.*t36.*4.0+Ixx3.*Izz2.*m3.*t6.*t8.*t20.*t30.*t36.*2.0;
et106 = Iyy2.*Iyy3.*m3.*t6.*t8.*t20.*t30.*t36.*-2.0+Ixx3.*Izz3.*m3.*t6.*t8.*t20.*t30.*t36.*4.0-Ixx3.*Izz3.*m3.*t8.*t14.*t30.*t33.*t37.*4.0-Ixx3.*Izz3.*m3.*t8.*t14.*t31.*t33.*t37.*8.0-Ixx3.*Izz3.*m2.*t8.*t18.*t30.*t33.*t37.*4.0+Ixx3.*Izz3.*m3.*t8.*t14.*t30.*t36.*t37.*8.0-Ixx3.*Izz3.*m2.*t8.*t18.*t31.*t33.*t37.*8.0+Ixx3.*Izz2.*m3.*t8.*t20.*t30.*t33.*t37.*4.0+Ixx3.*Izz2.*m3.*t8.*t20.*t31.*t33.*t37.*4.0+Ixx3.*Izz3.*m2.*t8.*t18.*t30.*t36.*t37.*8.0-Ixx2.*Izz3.*m3.*t8.*t20.*t30.*t36.*t37.*4.0-Ixx3.*Izz2.*m3.*t8.*t20.*t30.*t36.*t37.*4.0-Iyy2.*Izz3.*m3.*t6.*t8.*t14.*t30.*t33.*2.0-Iyy2.*Izz3.*m3.*t6.*t8.*t14.*t31.*t33.*2.0-Iyy2.*Izz3.*m2.*t6.*t8.*t18.*t30.*t33.*2.0+Iyy2.*Izz3.*m3.*t6.*t8.*t14.*t30.*t36.*2.0-Iyy2.*Izz3.*m2.*t6.*t8.*t18.*t31.*t33.*2.0+Iyy2.*Izz3.*m2.*t6.*t8.*t18.*t30.*t36.*2.0;
et107 = Iyy2.*Izz3.*m3.*t6.*t8.*t20.*t30.*t33.*-2.0-Iyy3.*Izz2.*m3.*t6.*t8.*t20.*t30.*t33.*2.0+Iyy2.*Izz3.*m3.*t6.*t8.*t20.*t31.*t33.*2.0+Iyy3.*Izz2.*m3.*t6.*t8.*t20.*t30.*t36.*2.0-Iyy3.*Izz3.*m3.*t6.*t8.*t20.*t30.*t36.*4.0-Iyy2.*Izz3.*m3.*t8.*t20.*t31.*t33.*t37.*4.0+Iyy2.*Izz3.*m3.*t8.*t20.*t30.*t36.*t37.*4.0-Izz2.*Izz3.*m3.*t6.*t8.*t14.*t30.*t33.*2.0-Izz2.*Izz3.*m3.*t6.*t8.*t14.*t31.*t33.*2.0-Izz2.*Izz3.*m2.*t6.*t8.*t18.*t30.*t33.*2.0+Izz2.*Izz3.*m3.*t6.*t8.*t14.*t30.*t36.*2.0-Izz2.*Izz3.*m2.*t6.*t8.*t18.*t31.*t33.*2.0+Izz2.*Izz3.*m2.*t6.*t8.*t18.*t30.*t36.*2.0+Ixx1.*g.*lcm3.*m2.*m3.*t5.*t8.*t18.*2.0+Ixx2.*g.*lcm3.*m2.*m3.*t8.*t18.*t34.*2.0+Ixx3.*g.*lcm3.*m2.*m3.*t8.*t18.*t34.*2.0+Iyy2.*g.*lcm3.*m2.*m3.*t5.*t8.*t18.*2.0+Iyy3.*g.*lcm3.*m2.*m3.*t5.*t8.*t18.*2.0-Iyy2.*g.*lcm3.*m2.*m3.*t8.*t18.*t34.*2.0;
et108 = Iyy3.*g.*lcm3.*m2.*m3.*t8.*t18.*t34.*-2.0+Izz2.*g.*lcm3.*m2.*m3.*t5.*t8.*t18.*2.0+Izz3.*g.*lcm3.*m2.*m3.*t5.*t8.*t18.*2.0-Izz2.*g.*lcm3.*m2.*m3.*t8.*t18.*t34.*2.0-Izz3.*g.*lcm3.*m2.*m3.*t8.*t18.*t34.*2.0-Ixx1.*l2.*lcm3.*m2.*m3.*t8.*t18.*t30.*2.0-Ixx1.*l2.*lcm3.*m2.*m3.*t8.*t18.*t31.*2.0-Ixx3.*l2.*lcm3.*m2.*m3.*t8.*t18.*t30.*2.0-Ixx3.*l2.*lcm3.*m2.*m3.*t8.*t18.*t31.*8.0+Ixx3.*l2.*lcm3.*m2.*m3.*t18.*t30.*t49.*2.0+Ixx3.*l2.*lcm3.*m2.*m3.*t18.*t31.*t49.*8.0-Iyy2.*l2.*lcm3.*m2.*m3.*t8.*t18.*t30.*2.0-Iyy2.*l2.*lcm3.*m2.*m3.*t8.*t18.*t31.*2.0-Iyy3.*l2.*lcm3.*m2.*m3.*t8.*t18.*t30.*2.0-Iyy3.*l2.*lcm3.*m2.*m3.*t8.*t18.*t32.*2.0-Izz2.*l2.*lcm3.*m2.*m3.*t8.*t18.*t30.*2.0-Izz2.*l2.*lcm3.*m2.*m3.*t8.*t18.*t31.*2.0+Izz3.*l2.*lcm3.*m2.*m3.*t8.*t18.*t31.*6.0;
et109 = Izz3.*l2.*lcm3.*m2.*m3.*t18.*t30.*t49.*-2.0-Izz3.*l2.*lcm3.*m2.*m3.*t18.*t31.*t49.*8.0-Iyy3.*l2.*lcm3.*m3.*t2.*t5.*t7.*t8.*2.0+Ixx1.*g.*l2.*t5.*t6.*t8.*t20.*t26.*4.0-Ixx3.*g.*l2.*t5.*t6.*t8.*t20.*t26.*2.0+Ixx2.*g.*l2.*t6.*t8.*t20.*t26.*t34.*4.0+Ixx3.*g.*l2.*t6.*t8.*t20.*t26.*t34.*2.0+Ixx3.*g.*l2.*t5.*t8.*t20.*t26.*t37.*2.0-Ixx3.*g.*l2.*t8.*t20.*t26.*t34.*t37.*2.0+Iyy2.*g.*l2.*t5.*t6.*t8.*t20.*t26.*4.0-Iyy2.*g.*l2.*t6.*t8.*t20.*t26.*t34.*4.0+Izz2.*g.*l2.*t5.*t6.*t8.*t20.*t26.*4.0+Izz3.*g.*l2.*t5.*t6.*t8.*t20.*t26.*6.0-Izz2.*g.*l2.*t6.*t8.*t20.*t26.*t34.*4.0-Izz3.*g.*l2.*t6.*t8.*t20.*t26.*t34.*2.0-Izz3.*g.*l2.*t5.*t8.*t20.*t26.*t37.*2.0+Izz3.*g.*l2.*t8.*t20.*t26.*t34.*t37.*2.0-Ixx3.*g.*lcm3.*t8.*t14.*t26.*t34.*t35.*2.0;
et110 = Izz3.*g.*lcm3.*t8.*t14.*t26.*t34.*t35.*2.0-Ixx3.*m2.*m3.*qp1.*qp2.*t5.*t14.*t18.*4.0+Ixx2.*m2.*m3.*qp1.*qp2.*t5.*t18.*t20.*4.0+Ixx3.*m2.*m3.*qp1.*qp2.*t5.*t18.*t20.*2.0+Ixx3.*m2.*m3.*qp1.*qp2.*t14.*t18.*t34.*4.0-Ixx2.*m2.*m3.*qp1.*qp2.*t18.*t20.*t34.*4.0-Ixx3.*m2.*m3.*qp1.*qp2.*t18.*t20.*t34.*4.0+Ixx3.*m2.*m3.*qp2.*qp3.*t18.*t20.*t44-Iyy3.*m2.*m3.*qp1.*qp2.*t5.*t14.*t18.*4.0-Iyy3.*m2.*m3.*qp1.*qp2.*t5.*t18.*t20.*2.0+Iyy3.*m2.*m3.*qp1.*qp2.*t14.*t18.*t34.*4.0+Iyy3.*m2.*m3.*qp1.*qp2.*t18.*t20.*t34.*4.0+Iyy3.*m2.*m3.*qp2.*qp3.*t18.*t20.*t44.*3.0+Izz3.*m2.*m3.*qp1.*qp2.*t5.*t14.*t18.*4.0-Izz3.*m2.*m3.*qp1.*qp2.*t14.*t18.*t34.*4.0-Ixx3.*m2.*m3.*t8.*t18.*t20.*t31.*t37.*4.0+Ixx2.*l2.*qp1.*qp2.*t5.*t6.*t22.*t26.*8.0+Ixx3.*l2.*qp1.*qp2.*t5.*t6.*t22.*t26.*4.0+Ixx3.*l2.*qp1.*qp3.*t7.*t8.*t22.*t26.*2.0;
et111 = Ixx2.*l2.*qp1.*qp2.*t6.*t22.*t26.*t34.*-8.0+Ixx1.*l2.*qp1.*qp2.*t5.*t22.*t26.*t37.*1.2e+1-Ixx3.*l2.*qp1.*qp2.*t6.*t22.*t26.*t34.*4.0+Ixx2.*l2.*qp1.*qp2.*t5.*t22.*t26.*t37.*4.0-Ixx3.*l2.*qp1.*qp2.*t5.*t22.*t26.*t37.*4.0+Ixx3.*l2.*qp1.*qp2.*t5.*t22.*t26.*t39.*8.0+Ixx3.*l2.*qp1.*qp3.*t8.*t22.*t26.*t47.*2.0-Ixx3.*l2.*qp1.*qp3.*t7.*t22.*t26.*t49.*4.0+Ixx2.*l2.*qp1.*qp2.*t22.*t26.*t34.*t37.*8.0+Ixx3.*l2.*qp1.*qp2.*t22.*t26.*t34.*t37.*4.0-Ixx3.*l2.*qp1.*qp2.*t22.*t26.*t34.*t39.*8.0-Iyy2.*l2.*qp1.*qp2.*t5.*t6.*t22.*t26.*4.0-Iyy3.*l2.*qp1.*qp2.*t5.*t6.*t22.*t26.*4.0+Iyy3.*l2.*qp1.*qp3.*t7.*t8.*t22.*t26.*6.0+Iyy2.*l2.*qp1.*qp2.*t6.*t22.*t26.*t34.*8.0+Iyy3.*l2.*qp1.*qp2.*t6.*t22.*t26.*t34.*4.0+Iyy2.*l2.*qp1.*qp2.*t5.*t22.*t26.*t37.*4.0-Iyy3.*l2.*qp1.*qp2.*t5.*t22.*t26.*t37.*4.0;
et112 = Iyy2.*l2.*qp1.*qp3.*t8.*t22.*t26.*t47.*4.0-Iyy3.*l2.*qp1.*qp3.*t8.*t22.*t26.*t47.*2.0-Iyy3.*l2.*qp1.*qp3.*t7.*t22.*t26.*t49.*4.0-Iyy2.*l2.*qp1.*qp2.*t22.*t26.*t34.*t37.*8.0+Iyy3.*l2.*qp1.*qp2.*t22.*t26.*t34.*t37.*4.0-Izz2.*l2.*qp1.*qp2.*t5.*t6.*t22.*t26.*8.0-Izz3.*l2.*qp1.*qp3.*t7.*t8.*t22.*t26.*2.0+Izz2.*l2.*qp1.*qp2.*t6.*t22.*t26.*t34.*8.0+Izz3.*l2.*qp1.*qp2.*t6.*t22.*t26.*t34.*4.0+Izz2.*l2.*qp1.*qp2.*t5.*t22.*t26.*t37.*8.0+Izz3.*l2.*qp1.*qp2.*t5.*t22.*t26.*t37.*1.2e+1-Izz3.*l2.*qp1.*qp2.*t5.*t22.*t26.*t39.*8.0+Izz3.*l2.*qp1.*qp3.*t8.*t22.*t26.*t47.*2.0+Izz3.*l2.*qp1.*qp3.*t7.*t22.*t26.*t49.*4.0-Izz2.*l2.*qp1.*qp2.*t22.*t26.*t34.*t37.*8.0-Izz3.*l2.*qp1.*qp2.*t22.*t26.*t34.*t37.*4.0+Izz3.*l2.*qp1.*qp2.*t22.*t26.*t34.*t39.*8.0+Ixx1.*lcm3.*qp1.*qp2.*t5.*t6.*t15.*t26.*4.0;
et113 = Ixx2.*lcm3.*qp1.*qp2.*t5.*t6.*t15.*t26.*4.0-Ixx3.*lcm3.*qp1.*qp2.*t5.*t6.*t15.*t26.*4.0+Ixx3.*lcm3.*qp1.*qp2.*t6.*t15.*t26.*t34.*8.0+Ixx3.*lcm3.*qp1.*qp2.*t5.*t15.*t26.*t37.*1.2e+1-Ixx3.*lcm3.*qp1.*qp2.*t15.*t26.*t34.*t37.*1.6e+1-Iyy3.*lcm3.*qp1.*qp2.*t5.*t6.*t15.*t26.*8.0+Iyy3.*lcm3.*qp1.*qp2.*t6.*t15.*t26.*t34.*8.0+Iyy3.*lcm3.*qp1.*qp3.*t8.*t15.*t26.*t47.*4.0+Izz3.*lcm3.*qp1.*qp2.*t5.*t6.*t15.*t26.*8.0-Izz3.*lcm3.*qp1.*qp2.*t6.*t15.*t26.*t34.*8.0-Izz3.*lcm3.*qp1.*qp2.*t5.*t15.*t26.*t37.*1.2e+1+Izz3.*lcm3.*qp1.*qp2.*t15.*t26.*t34.*t37.*1.6e+1+Ixx1.*l2.*t8.*t22.*t26.*t30.*t33.*t35.*6.0-Ixx2.*l2.*t8.*t22.*t26.*t31.*t33.*t35.*6.0+Ixx3.*l2.*t8.*t22.*t26.*t30.*t33.*t35.*4.0+Ixx2.*l2.*t8.*t22.*t26.*t30.*t35.*t36.*4.0+Ixx3.*l2.*t8.*t22.*t26.*t32.*t33.*t35.*2.0+Ixx3.*l2.*t8.*t22.*t26.*t30.*t33.*t38.*4.0;
et114 = Ixx3.*l2.*t8.*t22.*t26.*t30.*t35.*t36.*-2.0+Ixx3.*l2.*t8.*t22.*t26.*t31.*t33.*t38.*4.0-Ixx3.*l2.*t8.*t22.*t26.*t30.*t36.*t38.*4.0+Iyy2.*l2.*t8.*t22.*t26.*t30.*t33.*t35.*6.0+Iyy2.*l2.*t8.*t22.*t26.*t31.*t33.*t35.*4.0-Iyy2.*l2.*t8.*t22.*t26.*t30.*t35.*t36.*6.0+Iyy3.*l2.*t8.*t22.*t26.*t32.*t33.*t35.*2.0+Iyy3.*l2.*t8.*t22.*t26.*t30.*t35.*t36.*2.0+Izz2.*l2.*t8.*t22.*t26.*t30.*t33.*t35.*6.0+Izz2.*l2.*t8.*t22.*t26.*t31.*t33.*t35.*6.0+Izz3.*l2.*t8.*t22.*t26.*t30.*t33.*t35.*2.0-Izz3.*l2.*t8.*t22.*t26.*t31.*t33.*t35.*2.0-Izz2.*l2.*t8.*t22.*t26.*t30.*t35.*t36.*4.0-Izz3.*l2.*t8.*t22.*t26.*t32.*t33.*t35.*2.0-Izz3.*l2.*t8.*t22.*t26.*t30.*t33.*t38.*4.0-Izz3.*l2.*t8.*t22.*t26.*t31.*t33.*t38.*4.0+Izz3.*l2.*t8.*t22.*t26.*t30.*t36.*t38.*4.0+Ixx3.*lcm3.*t8.*t15.*t26.*t30.*t33.*t35.*1.2e+1+Ixx3.*lcm3.*t8.*t15.*t26.*t31.*t33.*t35.*1.0e+1;
et115 = Ixx3.*lcm3.*t8.*t15.*t26.*t30.*t35.*t36.*-1.0e+1-Izz3.*lcm3.*t8.*t15.*t26.*t30.*t33.*t35.*1.2e+1-Izz3.*lcm3.*t8.*t15.*t26.*t31.*t33.*t35.*1.0e+1+Izz3.*lcm3.*t8.*t15.*t26.*t30.*t35.*t36.*1.0e+1-Ixx3.*m3.*t2.*t5.*t6.*t7.*t8.*t20.*2.0-Iyy3.*m3.*t2.*t5.*t6.*t7.*t8.*t20.*2.0+Izz3.*m3.*t2.*t5.*t6.*t7.*t8.*t20.*2.0+Ixx3.*qp1.*qp3.*t6.*t7.*t8.*t11.*t33.*2.0-Ixx3.*qp2.*qp3.*t5.*t7.*t23.*t26.*t35.*2.0+Ixx2.*qp1.*qp2.*t5.*t14.*t20.*t26.*t35.*8.0+Ixx2.*qp1.*qp2.*t14.*t20.*t26.*t34.*t35.*4.0-Iyy3.*qp1.*qp3.*t6.*t7.*t8.*t10.*t33.*2.0+Iyy3.*qp1.*qp3.*t6.*t7.*t8.*t13.*t33.*2.0-Iyy2.*qp2.*qp3.*t5.*t7.*t23.*t26.*t35.*4.0+Iyy3.*qp2.*qp3.*t5.*t7.*t23.*t26.*t35.*2.0-Izz3.*qp1.*qp3.*t6.*t7.*t8.*t11.*t33.*2.0-Izz3.*qp2.*qp3.*t5.*t7.*t23.*t26.*t35.*2.0+Ixx2.*t6.*t8.*t14.*t20.*t26.*t30.*t36.*4.0;
et116 = Ixx3.*t8.*t14.*t20.*t26.*t30.*t36.*t37.*-1.2e+1+Iyy3.*t6.*t8.*t14.*t20.*t26.*t30.*t33.*2.0+Iyy3.*t6.*t8.*t14.*t20.*t26.*t32.*t33.*4.0+Iyy3.*t6.*t8.*t14.*t20.*t26.*t30.*t36.*2.0-g.*l2.*lcm2.*m2.*t5.*t8.*t22.*t26.*2.0+g.*l2.*lcm2.*m2.*t8.*t22.*t26.*t34.*2.0+l2.*lcm3.*m2.*m3.*t1.*t6.*t7.*t18.*2.0-l2.*lcm3.*m2.*m3.*t3.*t6.*t18.*t33.*8.0-l2.*lcm3.*m3.*qp1.*qp2.*t5.*t6.*t11.*4.0+l2.*lcm3.*m3.*qp1.*qp2.*t5.*t6.*t13.*4.0+l2.*lcm3.*m3.*qp1.*qp3.*t7.*t8.*t11.*2.0+l2.*lcm3.*m3.*qp1.*qp2.*t6.*t11.*t34.*4.0+l2.*lcm3.*m3.*qp1.*qp2.*t5.*t10.*t39.*4.0-l2.*lcm3.*m3.*qp1.*qp2.*t5.*t13.*t37.*8.0+l2.*lcm3.*m3.*qp1.*qp2.*t5.*t13.*t39.*4.0-l2.*lcm3.*m3.*qp1.*qp3.*t8.*t11.*t47.*2.0-l2.*lcm3.*m3.*qp1.*qp2.*t10.*t34.*t39.*4.0-l2.*lcm3.*m3.*qp1.*qp2.*t13.*t34.*t39.*4.0;
et117 = g.*lcm2.*m2.*t5.*t6.*t8.*t23.*t26.*-2.0+g.*lcm3.*m2.*t5.*t8.*t14.*t18.*t26.*4.0+g.*lcm2.*m2.*t6.*t8.*t23.*t26.*t34.*2.0-g.*lcm3.*m2.*t8.*t14.*t18.*t26.*t34.*4.0+l2.*lcm3.*m3.*t8.*t10.*t30.*t33.*t35.*2.0+l2.*lcm3.*m3.*t8.*t21.*t25.*t30.*t33.*4.0+l2.*lcm3.*m3.*t8.*t21.*t25.*t31.*t33.*2.0+l2.*lcm3.*m3.*t8.*t10.*t30.*t33.*t38.*2.0-l2.*lcm3.*m3.*t8.*t10.*t30.*t35.*t36.*2.0-l2.*lcm3.*m3.*t8.*t13.*t30.*t33.*t35.*4.0+l2.*lcm3.*m3.*t8.*t10.*t31.*t33.*t38.*2.0+l2.*lcm3.*m3.*t8.*t13.*t31.*t33.*t35.*2.0-l2.*lcm3.*m3.*t8.*t21.*t25.*t30.*t36.*2.0-l2.*lcm3.*m3.*t8.*t10.*t30.*t36.*t38.*2.0+l2.*lcm3.*m3.*t8.*t13.*t30.*t33.*t38.*2.0+l2.*lcm3.*m3.*t8.*t13.*t31.*t33.*t38.*2.0-l2.*lcm3.*m3.*t8.*t13.*t30.*t36.*t38.*2.0+g.*m2.*t5.*t8.*t18.*t22.*t26.*t35.*2.0-g.*m2.*t8.*t18.*t22.*t26.*t34.*t35.*4.0;
et118 = l2.*m2.*t8.*t18.*t22.*t26.*t31.*t33.*-2.0+l2.*m2.*t8.*t18.*t22.*t26.*t32.*t33.*2.0+l2.*m2.*t8.*t18.*t22.*t26.*t30.*t36.*2.0+lcm3.*m2.*t8.*t15.*t18.*t26.*t30.*t33.*8.0+lcm3.*m2.*t8.*t15.*t18.*t26.*t31.*t33.*4.0-lcm3.*m2.*t8.*t15.*t18.*t26.*t30.*t36.*4.0-m3.*qp2.*qp3.*t5.*t7.*t10.*t20.*t35.*2.0+m3.*qp2.*qp3.*t5.*t7.*t11.*t20.*t35.*2.0-m2.*qp1.*qp2.*t5.*t14.*t18.*t20.*t26.*8.0+m3.*qp2.*qp3.*t5.*t7.*t13.*t20.*t35.*2.0+m2.*qp1.*qp2.*t5.*t18.*t23.*t26.*t38.*4.0+m2.*qp1.*qp2.*t14.*t18.*t20.*t26.*t34.*8.0-m2.*qp1.*qp2.*t18.*t23.*t26.*t34.*t38.*8.0-l2.*t2.*t5.*t7.*t8.*t22.*t26.*t35.*2.0+m2.*t6.*t8.*t18.*t23.*t26.*t30.*t36.*2.0-m2.*t8.*t18.*t23.*t26.*t30.*t36.*t37.*4.0+qp1.*qp3.*t6.*t7.*t8.*t14.*t23.*t27.*8.0+qp1.*qp3.*t7.*t8.*t14.*t23.*t27.*t37.*4.0;
et119 = t2.*t5.*t6.*t7.*t8.*t14.*t20.*t26.*-2.0-Ixx1.*Ixx3.*l2.*lcm3.*m3.*qp1.*qp2.*t5.*t6.*4.0-Ixx2.*Ixx3.*l2.*lcm3.*m3.*qp1.*qp2.*t6.*t34.*4.0+Ixx1.*Ixx3.*l2.*lcm3.*m3.*qp1.*qp2.*t5.*t37.*1.2e+1+Ixx2.*Ixx3.*l2.*lcm3.*m3.*qp1.*qp2.*t5.*t37.*4.0+Ixx2.*Ixx3.*l2.*lcm3.*m3.*qp1.*qp2.*t34.*t37.*8.0+Ixx1.*Iyy2.*l2.*lcm3.*m3.*qp1.*qp2.*t5.*t6.*4.0+Ixx1.*Iyy3.*l2.*lcm3.*m3.*qp1.*qp2.*t5.*t6.*4.0+Ixx2.*Iyy2.*l2.*lcm3.*m3.*qp1.*qp2.*t5.*t6.*4.0+Ixx2.*Iyy3.*l2.*lcm3.*m3.*qp1.*qp2.*t5.*t6.*8.0+Ixx3.*Iyy3.*l2.*lcm3.*m3.*qp1.*qp2.*t5.*t6.*4.0+Ixx3.*Iyy3.*l2.*lcm3.*m3.*qp1.*qp3.*t7.*t8.*2.0-Ixx2.*Iyy3.*l2.*lcm3.*m3.*qp1.*qp2.*t6.*t34.*4.0+Ixx3.*Iyy2.*l2.*lcm3.*m3.*qp1.*qp2.*t6.*t34.*4.0-Ixx3.*Iyy3.*l2.*lcm3.*m3.*qp1.*qp2.*t6.*t34.*4.0+Ixx3.*Iyy2.*l2.*lcm3.*m3.*qp1.*qp2.*t5.*t37.*4.0-Ixx3.*Iyy3.*l2.*lcm3.*m3.*qp1.*qp2.*t5.*t37.*4.0;
et120 = Ixx3.*Iyy3.*l2.*lcm3.*m3.*qp1.*qp3.*t8.*t47.*2.0-Ixx3.*Iyy3.*l2.*lcm3.*m3.*qp1.*qp3.*t7.*t49.*4.0-Ixx3.*Iyy2.*l2.*lcm3.*m3.*qp1.*qp2.*t34.*t37.*8.0+Ixx3.*Iyy3.*l2.*lcm3.*m3.*qp1.*qp2.*t34.*t37.*4.0+Ixx1.*Izz3.*l2.*lcm3.*m3.*qp1.*qp2.*t5.*t6.*8.0+Ixx2.*Izz3.*l2.*lcm3.*m3.*qp1.*qp2.*t5.*t6.*4.0-Ixx3.*Izz2.*l2.*lcm3.*m3.*qp1.*qp2.*t5.*t6.*4.0-Iyy2.*Iyy3.*l2.*lcm3.*m3.*qp1.*qp2.*t5.*t6.*4.0+Ixx2.*Izz3.*l2.*lcm3.*m3.*qp1.*qp2.*t6.*t34.*4.0+Ixx3.*Izz2.*l2.*lcm3.*m3.*qp1.*qp2.*t6.*t34.*4.0+Iyy2.*Iyy3.*l2.*lcm3.*m3.*qp1.*qp2.*t6.*t34.*4.0-Ixx1.*Izz3.*l2.*lcm3.*m3.*qp1.*qp2.*t5.*t37.*1.2e+1-Ixx2.*Izz3.*l2.*lcm3.*m3.*qp1.*qp2.*t5.*t37.*4.0+Ixx3.*Izz2.*l2.*lcm3.*m3.*qp1.*qp2.*t5.*t37.*8.0+Ixx3.*Izz3.*l2.*lcm3.*m3.*qp1.*qp2.*t5.*t37.*8.0-Ixx3.*Izz3.*l2.*lcm3.*m3.*qp1.*qp2.*t5.*t39.*8.0+Iyy2.*Iyy3.*l2.*lcm3.*m3.*qp1.*qp3.*t8.*t47.*4.0;
et121 = Ixx2.*Izz3.*l2.*lcm3.*m3.*qp1.*qp2.*t34.*t37.*-8.0-Ixx3.*Izz2.*l2.*lcm3.*m3.*qp1.*qp2.*t34.*t37.*8.0+Ixx3.*Izz3.*l2.*lcm3.*m3.*qp1.*qp2.*t34.*t39.*8.0+Iyy2.*Izz3.*l2.*lcm3.*m3.*qp1.*qp2.*t5.*t6.*4.0-Iyy3.*Izz2.*l2.*lcm3.*m3.*qp1.*qp2.*t5.*t6.*4.0-Iyy3.*Izz3.*l2.*lcm3.*m3.*qp1.*qp3.*t7.*t8.*2.0-Iyy2.*Izz3.*l2.*lcm3.*m3.*qp1.*qp2.*t6.*t34.*4.0+Iyy3.*Izz2.*l2.*lcm3.*m3.*qp1.*qp2.*t6.*t34.*4.0+Iyy3.*Izz3.*l2.*lcm3.*m3.*qp1.*qp2.*t6.*t34.*4.0-Iyy2.*Izz3.*l2.*lcm3.*m3.*qp1.*qp2.*t5.*t37.*4.0+Iyy3.*Izz3.*l2.*lcm3.*m3.*qp1.*qp2.*t5.*t37.*4.0+Iyy3.*Izz3.*l2.*lcm3.*m3.*qp1.*qp3.*t8.*t47.*2.0+Iyy3.*Izz3.*l2.*lcm3.*m3.*qp1.*qp3.*t7.*t49.*4.0+Iyy2.*Izz3.*l2.*lcm3.*m3.*qp1.*qp2.*t34.*t37.*8.0-Iyy3.*Izz3.*l2.*lcm3.*m3.*qp1.*qp2.*t34.*t37.*4.0+Izz2.*Izz3.*l2.*lcm3.*m3.*qp1.*qp2.*t5.*t6.*4.0-Izz2.*Izz3.*l2.*lcm3.*m3.*qp1.*qp2.*t6.*t34.*4.0;
et122 = Izz2.*Izz3.*l2.*lcm3.*m3.*qp1.*qp2.*t5.*t37.*-8.0+Izz2.*Izz3.*l2.*lcm3.*m3.*qp1.*qp2.*t34.*t37.*8.0+Ixx1.*Ixx3.*l2.*lcm3.*m3.*t8.*t30.*t33.*t35.*6.0-Ixx2.*Ixx3.*l2.*lcm3.*m3.*t8.*t31.*t33.*t35.*6.0+Ixx2.*Ixx3.*l2.*lcm3.*m3.*t8.*t30.*t35.*t36.*4.0+Ixx3.*Iyy2.*l2.*lcm3.*m3.*t8.*t30.*t33.*t35.*6.0+Ixx3.*Iyy2.*l2.*lcm3.*m3.*t8.*t31.*t33.*t35.*4.0-Ixx3.*Iyy2.*l2.*lcm3.*m3.*t8.*t30.*t35.*t36.*6.0+Ixx3.*Iyy3.*l2.*lcm3.*m3.*t8.*t32.*t33.*t35.*2.0+Ixx3.*Iyy3.*l2.*lcm3.*m3.*t8.*t30.*t35.*t36.*2.0-Ixx1.*Izz3.*l2.*lcm3.*m3.*t8.*t30.*t33.*t35.*6.0+Ixx3.*Izz2.*l2.*lcm3.*m3.*t8.*t30.*t33.*t35.*6.0+Ixx2.*Izz3.*l2.*lcm3.*m3.*t8.*t31.*t33.*t35.*6.0+Ixx3.*Izz2.*l2.*lcm3.*m3.*t8.*t31.*t33.*t35.*6.0+Ixx3.*Izz3.*l2.*lcm3.*m3.*t8.*t30.*t33.*t35.*2.0-Ixx3.*Izz3.*l2.*lcm3.*m3.*t8.*t31.*t33.*t35.*2.0-Ixx2.*Izz3.*l2.*lcm3.*m3.*t8.*t30.*t35.*t36.*4.0;
et123 = Ixx3.*Izz2.*l2.*lcm3.*m3.*t8.*t30.*t35.*t36.*-4.0-Ixx3.*Izz3.*l2.*lcm3.*m3.*t8.*t30.*t33.*t38.*4.0+Ixx3.*Izz3.*l2.*lcm3.*m3.*t8.*t30.*t35.*t36.*2.0-Ixx3.*Izz3.*l2.*lcm3.*m3.*t8.*t31.*t33.*t38.*4.0+Ixx3.*Izz3.*l2.*lcm3.*m3.*t8.*t30.*t36.*t38.*4.0-Iyy2.*Izz3.*l2.*lcm3.*m3.*t8.*t30.*t33.*t35.*6.0-Iyy2.*Izz3.*l2.*lcm3.*m3.*t8.*t31.*t33.*t35.*4.0+Iyy2.*Izz3.*l2.*lcm3.*m3.*t8.*t30.*t35.*t36.*6.0-Iyy3.*Izz3.*l2.*lcm3.*m3.*t8.*t32.*t33.*t35.*2.0-Iyy3.*Izz3.*l2.*lcm3.*m3.*t8.*t30.*t35.*t36.*2.0-Izz2.*Izz3.*l2.*lcm3.*m3.*t8.*t30.*t33.*t35.*6.0-Izz2.*Izz3.*l2.*lcm3.*m3.*t8.*t31.*t33.*t35.*6.0+Izz2.*Izz3.*l2.*lcm3.*m3.*t8.*t30.*t35.*t36.*4.0-Ixx3.*Iyy2.*m3.*qp2.*qp3.*t5.*t7.*t20.*t35.*4.0-Iyy2.*Iyy3.*m3.*qp2.*qp3.*t5.*t7.*t20.*t35.*4.0+Iyy2.*Izz3.*m3.*qp2.*qp3.*t5.*t7.*t20.*t35.*4.0-Iyy3.*Izz3.*m3.*qp2.*qp3.*t5.*t7.*t20.*t35.*4.0;
et124 = Iyy3.*g.*l2.*lcm2.*lcm3.*m2.*m3.*t5.*t8.*-2.0+Iyy3.*g.*l2.*lcm2.*lcm3.*m2.*m3.*t8.*t34.*2.0-Ixx3.*g.*lcm2.*m2.*m3.*t5.*t6.*t8.*t20.*2.0+Ixx3.*g.*lcm3.*m2.*m3.*t5.*t8.*t18.*t35.*2.0+Ixx3.*g.*lcm2.*m2.*m3.*t6.*t8.*t20.*t34.*2.0-Ixx3.*g.*lcm3.*m2.*m3.*t8.*t18.*t34.*t35.*4.0-Iyy3.*g.*lcm2.*m2.*m3.*t5.*t6.*t8.*t20.*2.0+Iyy3.*g.*lcm2.*m2.*m3.*t6.*t8.*t20.*t34.*2.0+Izz3.*g.*lcm2.*m2.*m3.*t5.*t6.*t8.*t20.*2.0-Izz3.*g.*lcm3.*m2.*m3.*t5.*t8.*t18.*t35.*2.0-Izz3.*g.*lcm2.*m2.*m3.*t6.*t8.*t20.*t34.*2.0+Izz3.*g.*lcm3.*m2.*m3.*t8.*t18.*t34.*t35.*4.0+Ixx1.*l2.*lcm3.*m2.*m3.*t8.*t18.*t30.*t33.*2.0-Ixx2.*l2.*lcm3.*m2.*m3.*t8.*t18.*t30.*t33.*2.0-Ixx2.*l2.*lcm3.*m2.*m3.*t8.*t18.*t31.*t33.*2.0-Ixx3.*l2.*lcm3.*m2.*m3.*t8.*t18.*t30.*t33.*2.0-Ixx3.*l2.*lcm3.*m2.*m3.*t8.*t18.*t31.*t33.*2.0;
et125 = Ixx2.*l2.*lcm3.*m2.*m3.*t8.*t18.*t30.*t36.*2.0+Ixx3.*l2.*lcm3.*m2.*m3.*t8.*t18.*t30.*t36.*2.0+Iyy2.*l2.*lcm3.*m2.*m3.*t8.*t18.*t30.*t33.*4.0+Iyy2.*l2.*lcm3.*m2.*m3.*t8.*t18.*t31.*t33.*2.0+Iyy3.*l2.*lcm3.*m2.*m3.*t8.*t18.*t30.*t33.*2.0-Iyy2.*l2.*lcm3.*m2.*m3.*t8.*t18.*t30.*t36.*2.0+Iyy3.*l2.*lcm3.*m2.*m3.*t8.*t18.*t32.*t33.*2.0+Izz2.*l2.*lcm3.*m2.*m3.*t8.*t18.*t30.*t33.*4.0+Izz2.*l2.*lcm3.*m2.*m3.*t8.*t18.*t31.*t33.*2.0+Izz3.*l2.*lcm3.*m2.*m3.*t8.*t18.*t30.*t33.*4.0+Izz3.*l2.*lcm3.*m2.*m3.*t8.*t18.*t31.*t33.*2.0-Izz2.*l2.*lcm3.*m2.*m3.*t8.*t18.*t30.*t36.*2.0-Izz3.*l2.*lcm3.*m2.*m3.*t8.*t18.*t30.*t36.*2.0-Ixx3.*l2.*lcm3.*m3.*t2.*t5.*t7.*t8.*t35.*2.0+Izz3.*l2.*lcm3.*m3.*t2.*t5.*t7.*t8.*t35.*2.0+Ixx3.*m2.*m3.*qp1.*qp2.*t5.*t14.*t18.*t35.*8.0+Ixx3.*m2.*m3.*qp1.*qp2.*t5.*t18.*t20.*t38.*8.0;
et126 = Ixx3.*m2.*m3.*qp1.*qp2.*t14.*t18.*t34.*t35.*-8.0+Ixx2.*m2.*m3.*qp1.*qp2.*t18.*t20.*t34.*t35.*4.0-Ixx3.*m2.*m3.*qp1.*qp2.*t18.*t20.*t34.*t38.*1.6e+1-Izz3.*m2.*m3.*qp1.*qp2.*t5.*t14.*t18.*t35.*8.0+Izz3.*m2.*m3.*qp1.*qp2.*t14.*t18.*t34.*t35.*8.0+Ixx3.*m2.*m3.*t6.*t8.*t14.*t18.*t30.*t33.*4.0+Ixx3.*m2.*m3.*t6.*t8.*t14.*t18.*t31.*t33.*4.0-Ixx3.*m2.*m3.*t6.*t8.*t14.*t18.*t30.*t36.*4.0+Ixx2.*m2.*m3.*t6.*t8.*t18.*t20.*t30.*t36.*2.0+Ixx3.*m2.*m3.*t6.*t8.*t18.*t20.*t30.*t36.*4.0-Ixx3.*m2.*m3.*t8.*t18.*t20.*t30.*t36.*t37.*8.0-Izz3.*m2.*m3.*t6.*t8.*t14.*t18.*t30.*t33.*4.0-Izz3.*m2.*m3.*t6.*t8.*t14.*t18.*t31.*t33.*4.0+Izz3.*m2.*m3.*t6.*t8.*t14.*t18.*t30.*t36.*4.0-Ixx3.*l2.*qp2.*qp3.*t5.*t6.*t7.*t22.*t26.*4.0-Ixx3.*l2.*qp2.*qp3.*t5.*t7.*t22.*t26.*t37.*2.0;
et127 = Iyy2.*l2.*qp2.*qp3.*t5.*t6.*t7.*t22.*t26.*4.0+Iyy3.*l2.*qp2.*qp3.*t5.*t6.*t7.*t22.*t26.*4.0-Iyy2.*l2.*qp2.*qp3.*t5.*t7.*t22.*t26.*t37.*4.0+Iyy3.*l2.*qp2.*qp3.*t5.*t7.*t22.*t26.*t37.*2.0+Izz3.*l2.*qp2.*qp3.*t5.*t6.*t7.*t22.*t26.*8.0-Izz3.*l2.*qp2.*qp3.*t5.*t7.*t22.*t26.*t37.*2.0+Ixx3.*lcm3.*qp2.*qp3.*t5.*t6.*t7.*t15.*t26.*2.0-Ixx3.*lcm3.*qp2.*qp3.*t5.*t7.*t15.*t26.*t37.*4.0-Izz3.*lcm3.*qp2.*qp3.*t5.*t6.*t7.*t15.*t26.*2.0+Izz3.*lcm3.*qp2.*qp3.*t5.*t7.*t15.*t26.*t37.*4.0-Ixx3.*qp1.*qp3.*t6.*t7.*t8.*t23.*t26.*t33.*2.0+Ixx3.*qp1.*qp3.*t7.*t8.*t14.*t20.*t26.*t37.*4.0+Iyy3.*qp1.*qp3.*t6.*t7.*t8.*t14.*t20.*t26.*8.0+Iyy3.*qp1.*qp3.*t6.*t7.*t8.*t23.*t26.*t33.*2.0-g.*l2.*lcm2.*m2.*t5.*t8.*t22.*t26.*t35.*2.0+g.*l2.*lcm2.*m2.*t8.*t22.*t26.*t34.*t35.*2.0+g.*l2.*m2.*t5.*t6.*t8.*t18.*t20.*t26.*8.0;
et128 = g.*l2.*m2.*t6.*t8.*t18.*t20.*t26.*t34.*-8.0+l2.*lcm3.*m3.*qp2.*qp3.*t5.*t6.*t7.*t11.*4.0-l2.*lcm3.*m3.*qp2.*qp3.*t5.*t6.*t7.*t13.*2.0-l2.*lcm3.*m3.*qp2.*qp3.*t5.*t7.*t10.*t37.*2.0+l2.*lcm3.*m3.*qp2.*qp3.*t5.*t7.*t13.*t37.*2.0-g.*lcm2.*m2.*t5.*t6.*t8.*t14.*t20.*t26.*2.0+g.*lcm2.*m2.*t6.*t8.*t14.*t20.*t26.*t34.*2.0-l2.*m2.*qp1.*qp2.*t5.*t6.*t18.*t22.*t26.*1.2e+1+l2.*m2.*qp1.*qp2.*t6.*t18.*t22.*t26.*t34.*1.6e+1+l2.*m2.*qp1.*qp2.*t5.*t18.*t22.*t26.*t37.*1.2e+1+l2.*m2.*qp1.*qp3.*t8.*t18.*t22.*t26.*t47.*4.0-l2.*m2.*qp1.*qp2.*t18.*t22.*t26.*t34.*t37.*1.6e+1+l2.*m2.*t8.*t18.*t22.*t26.*t30.*t33.*t35.*1.2e+1+l2.*m2.*t8.*t18.*t22.*t26.*t31.*t33.*t35.*1.0e+1-l2.*m2.*t8.*t18.*t22.*t26.*t30.*t35.*t36.*1.0e+1-l2.*qp1.*qp3.*t7.*t8.*t24.*t27.*t33.*t35.*4.0;
et129 = m3.*qp1.*qp3.*t6.*t7.*t8.*t10.*t20.*t33.*-2.0+m3.*qp1.*qp3.*t6.*t7.*t8.*t11.*t20.*t33.*2.0+m3.*qp1.*qp3.*t6.*t7.*t8.*t13.*t20.*t33.*2.0+m2.*t6.*t8.*t14.*t18.*t20.*t26.*t30.*t33.*1.8e+1+m2.*t6.*t8.*t14.*t18.*t20.*t26.*t31.*t33.*1.0e+1-m2.*t6.*t8.*t14.*t18.*t20.*t26.*t30.*t36.*1.0e+1-qp1.*qp3.*t6.*t7.*t8.*t14.*t23.*t27.*t33.*8.0-qp1.*qp3.*t7.*t8.*t15.*t22.*t27.*t33.*t35.*8.0-qp1.*qp3.*t7.*t8.*t14.*t23.*t27.*t33.*t37.*4.0+Iyy2.*Iyy3.*Izz3.*qp1.*qp3.*t6.*t7.*t8.*t33.*4.0+Ixx3.*Iyy2.*l2.*lcm3.*m3.*qp2.*qp3.*t5.*t6.*t7.*2.0-Ixx3.*Iyy3.*l2.*lcm3.*m3.*qp2.*qp3.*t5.*t6.*t7.*4.0-Ixx3.*Iyy2.*l2.*lcm3.*m3.*qp2.*qp3.*t5.*t7.*t37.*4.0+Ixx3.*Iyy3.*l2.*lcm3.*m3.*qp2.*qp3.*t5.*t7.*t37.*2.0+Iyy2.*Iyy3.*l2.*lcm3.*m3.*qp2.*qp3.*t5.*t6.*t7.*2.0+Ixx3.*Izz3.*l2.*lcm3.*m3.*qp2.*qp3.*t5.*t6.*t7.*2.0;
et130 = Iyy2.*Izz3.*l2.*lcm3.*m3.*qp2.*qp3.*t5.*t6.*t7.*-2.0+Iyy3.*Izz3.*l2.*lcm3.*m3.*qp2.*qp3.*t5.*t6.*t7.*6.0+Iyy2.*Izz3.*l2.*lcm3.*m3.*qp2.*qp3.*t5.*t7.*t37.*4.0-Iyy3.*Izz3.*l2.*lcm3.*m3.*qp2.*qp3.*t5.*t7.*t37.*2.0+Iyy2.*Izz3.*m3.*qp1.*qp3.*t6.*t7.*t8.*t20.*t33.*4.0-Ixx3.*g.*l2.*lcm2.*lcm3.*m2.*m3.*t5.*t8.*t35.*2.0+Ixx3.*g.*l2.*lcm2.*lcm3.*m2.*m3.*t8.*t34.*t35.*2.0+Izz3.*g.*l2.*lcm2.*lcm3.*m2.*m3.*t5.*t8.*t35.*2.0-Izz3.*g.*l2.*lcm2.*lcm3.*m2.*m3.*t8.*t34.*t35.*2.0+Ixx1.*l2.*lcm3.*m2.*m3.*qp1.*qp2.*t5.*t6.*t18.*4.0+Ixx2.*l2.*lcm3.*m2.*m3.*qp1.*qp2.*t5.*t6.*t18.*4.0-Ixx3.*l2.*lcm3.*m2.*m3.*qp1.*qp2.*t5.*t6.*t18.*4.0+Ixx3.*l2.*lcm3.*m2.*m3.*qp1.*qp2.*t6.*t18.*t34.*8.0+Ixx3.*l2.*lcm3.*m2.*m3.*qp1.*qp2.*t5.*t18.*t37.*1.2e+1-Ixx3.*l2.*lcm3.*m2.*m3.*qp1.*qp2.*t18.*t34.*t37.*1.6e+1;
et131 = Iyy3.*l2.*lcm3.*m2.*m3.*qp1.*qp2.*t5.*t6.*t18.*-8.0+Iyy3.*l2.*lcm3.*m2.*m3.*qp1.*qp2.*t6.*t18.*t34.*8.0+Iyy3.*l2.*lcm3.*m2.*m3.*qp1.*qp3.*t8.*t18.*t47.*4.0+Izz3.*l2.*lcm3.*m2.*m3.*qp1.*qp2.*t5.*t6.*t18.*8.0-Izz3.*l2.*lcm3.*m2.*m3.*qp1.*qp2.*t6.*t18.*t34.*8.0-Izz3.*l2.*lcm3.*m2.*m3.*qp1.*qp2.*t5.*t18.*t37.*1.2e+1+Izz3.*l2.*lcm3.*m2.*m3.*qp1.*qp2.*t18.*t34.*t37.*1.6e+1+Ixx3.*l2.*lcm3.*m2.*m3.*t8.*t18.*t30.*t33.*t35.*1.2e+1+Ixx3.*l2.*lcm3.*m2.*m3.*t8.*t18.*t31.*t33.*t35.*1.0e+1-Ixx3.*l2.*lcm3.*m2.*m3.*t8.*t18.*t30.*t35.*t36.*1.0e+1-Izz3.*l2.*lcm3.*m2.*m3.*t8.*t18.*t30.*t33.*t35.*1.2e+1-Izz3.*l2.*lcm3.*m2.*m3.*t8.*t18.*t31.*t33.*t35.*1.0e+1+Izz3.*l2.*lcm3.*m2.*m3.*t8.*t18.*t30.*t35.*t36.*1.0e+1-Ixx3.*l2.*qp1.*qp3.*t7.*t8.*t22.*t26.*t33.*t35.*6.0-Iyy2.*l2.*qp1.*qp3.*t7.*t8.*t22.*t26.*t33.*t35.*4.0;
et132 = Iyy3.*l2.*qp1.*qp3.*t7.*t8.*t22.*t26.*t33.*t35.*-2.0+Izz3.*l2.*qp1.*qp3.*t7.*t8.*t22.*t26.*t33.*t35.*2.0-Ixx3.*lcm3.*qp1.*qp3.*t7.*t8.*t15.*t26.*t33.*t35.*4.0+Izz3.*lcm3.*qp1.*qp3.*t7.*t8.*t15.*t26.*t33.*t35.*4.0-Iyy3.*qp1.*qp3.*t6.*t7.*t8.*t14.*t20.*t26.*t33.*6.0-l2.*lcm3.*m3.*qp1.*qp3.*t7.*t8.*t10.*t33.*t35.*2.0+l2.*lcm3.*m3.*qp1.*qp3.*t7.*t8.*t13.*t33.*t35.*2.0+l2.*m2.*qp2.*qp3.*t5.*t6.*t7.*t18.*t22.*t26.*4.0-l2.*m2.*qp2.*qp3.*t5.*t7.*t18.*t22.*t26.*t37.*4.0+m2.*qp1.*qp3.*t6.*t7.*t8.*t14.*t18.*t20.*t26.*4.0+Ixx3.*l2.*lcm3.*m2.*m3.*qp2.*qp3.*t5.*t6.*t7.*t18.*2.0-Ixx3.*l2.*lcm3.*m2.*m3.*qp2.*qp3.*t5.*t7.*t18.*t37.*4.0-Izz3.*l2.*lcm3.*m2.*m3.*qp2.*qp3.*t5.*t6.*t7.*t18.*2.0+Izz3.*l2.*lcm3.*m2.*m3.*qp2.*qp3.*t5.*t7.*t18.*t37.*4.0-l2.*m2.*qp1.*qp3.*t7.*t8.*t18.*t22.*t26.*t33.*t35.*4.0;
et133 = m2.*qp1.*qp3.*t6.*t7.*t8.*t14.*t18.*t20.*t26.*t33.*-4.0-Ixx3.*Iyy2.*l2.*lcm3.*m3.*qp1.*qp3.*t7.*t8.*t33.*t35.*4.0-Ixx3.*Iyy3.*l2.*lcm3.*m3.*qp1.*qp3.*t7.*t8.*t33.*t35.*2.0+Iyy2.*Izz3.*l2.*lcm3.*m3.*qp1.*qp3.*t7.*t8.*t33.*t35.*4.0+Iyy3.*Izz3.*l2.*lcm3.*m3.*qp1.*qp3.*t7.*t8.*t33.*t35.*2.0-Ixx3.*l2.*lcm3.*m2.*m3.*qp1.*qp3.*t7.*t8.*t18.*t33.*t35.*4.0+Izz3.*l2.*lcm3.*m2.*m3.*qp1.*qp3.*t7.*t8.*t18.*t33.*t35.*4.0;
qpp = [t274.*(et1+et2+et3+et4+et5+et6+et7+et8+et9+et10+et11+et12+et13+et14+et15+et16+et17+et18+et19+et20+et21+et22+et23);(t274.*(et24+et25+et26+et27+et28+et29+et30+et31+et32+et33+et34+et35+et36+et37+et38+et39+et40+et41+et42+et43+et44+et45+et46+et47+et48+et49+et50+et51+et52+et53+et54))./2.0;(t274.*(et55+et56+et57+et58+et59+et60+et61+et62+et63+et64+et65+et66+et67+et68+et69+et70+et71+et72+et73+et74+et75+et76+et77+et78+et79+et80+et81+et82+et83+et84+et85+et86+et87+et88+et89+et90+et91+et92+et93+et94+et95+et96+et97+et98+et99+et100+et101+et102+et103+et104+et105+et106+et107+et108+et109+et110+et111+et112+et113+et114+et115+et116+et117+et118+et119+et120+et121+et122+et123+et124+et125+et126+et127+et128+et129+et130+et131+et132+et133))./2.0];
end
